simulink library "outp"  (R2021b)
(part 10 of 11)

  UnitConverter274/1 -> VOUTP_AmbDimENFlash_enum/1  "VOUTP_AmbDimENFlash_enum"
  VBCM_AmbLinkDriStaFlash_enum/1 -> VBCM_AmbLinkDriStaFlash_enum_Inproc/1  "VBCM_AmbLinkDriStaFlash_enum"
  VBCM_AmbLinkDriStaFlash_enum_Inproc/1 -> UnitConverter275/1
  UnitConverter275/1 -> VOUTP_AmbLinkDriStaFlash_enum/1  "VOUTP_AmbLinkDriStaFlash_enum"
  VBCM_AmbPwrWarnENFlash_enum/1 -> VBCM_AmbPwrWarnENFlash_enum_Inproc/1  "VBCM_AmbPwrWarnENFlash_enum"
  VBCM_AmbPwrWarnENFlash_enum_Inproc/1 -> UnitConverter276/1
  UnitConverter276/1 -> VOUTP_AmbPwrWarnENFlash_enum/1  "VOUTP_AmbPwrWarnENFlash_enum"
  VBCM_AmbODAENFlash_enum/1 -> VBCM_AmbODAENFlash_enum_Inproc/1  "VBCM_AmbODAENFlash_enum"
  VBCM_AmbODAENFlash_enum_Inproc/1 -> UnitConverter277/1
  UnitConverter277/1 -> VOUTP_AmbODAENFlash_enum/1  "VOUTP_AmbODAENFlash_enum"
  VBCM_AmbColorSta1_enum/1 -> VBCM_AmbColorSta1_enum_Inproc/1  "VBCM_AmbColorSta1_enum"
  VBCM_AmbColorSta1_enum_Inproc/1 -> UnitConverter278/1
  UnitConverter278/1 -> VOUTP_AmbColorSta1_enum/1  "VOUTP_AmbColorSta1_enum"
  VBCM_AmbColorSta2_enum/1 -> VBCM_AmbColorSta2_enum_Inproc/1  "VBCM_AmbColorSta2_enum"
  VBCM_AmbColorSta2_enum_Inproc/1 -> UnitConverter279/1
  UnitConverter279/1 -> VOUTP_AmbColorSta2_enum/1  "VOUTP_AmbColorSta2_enum"
  VBCM_AmbColorSta3_enum/1 -> VBCM_AmbColorSta3_enum_Inproc/1  "VBCM_AmbColorSta3_enum"
  VBCM_AmbColorSta3_enum_Inproc/1 -> UnitConverter280/1
  UnitConverter280/1 -> VOUTP_AmbColorSta3_enum/1  "VOUTP_AmbColorSta3_enum"
  VBCM_AmbColorSta4_enum/1 -> VBCM_AmbColorSta4_enum_Inproc/1  "VBCM_AmbColorSta4_enum"
  VBCM_AmbColorSta4_enum_Inproc/1 -> UnitConverter281/1
  UnitConverter281/1 -> VOUTP_AmbColorSta4_enum/1  "VOUTP_AmbColorSta4_enum"
  VBCM_AmbColorSta5_enum/1 -> VBCM_AmbColorSta5_enum_Inproc/1  "VBCM_AmbColorSta5_enum"
  VBCM_AmbColorSta5_enum_Inproc/1 -> UnitConverter282/1
  UnitConverter282/1 -> VOUTP_AmbColorSta5_enum/1  "VOUTP_AmbColorSta5_enum"
  VBCM_AmbColorSta7_enum/1 -> VBCM_AmbColorSta7_enum_Inproc/1  "VBCM_AmbColorSta7_enum"
  VBCM_AmbColorSta7_enum_Inproc/1 -> UnitConverter283/1
  UnitConverter283/1 -> VOUTP_AmbColorSta7_enum/1  "VOUTP_AmbColorSta7_enum"
  VBCM_AmbBrightnessSta1_enum/1 -> VBCM_AmbBrightnessSta1_enum_Inproc/1  "VBCM_AmbBrightnessSta1_enum"
  VBCM_AmbBrightnessSta1_enum_Inproc/1 -> UnitConverter284/1
  UnitConverter284/1 -> VOUTP_AmbBrightnessSta1_enum/1  "VOUTP_AmbBrightnessSta1_enum"
  VBCM_AmbBrightnessSta2_enum/1 -> VBCM_AmbBrightnessSta2_enum_Inproc/1  "VBCM_AmbBrightnessSta2_enum"
  VBCM_AmbBrightnessSta2_enum_Inproc/1 -> UnitConverter285/1
  UnitConverter285/1 -> VOUTP_AmbBrightnessSta2_enum/1  "VOUTP_AmbBrightnessSta2_enum"
  VBCM_AmbBrightnessSta3_enum/1 -> VBCM_AmbBrightnessSta3_enum_Inproc/1  "VBCM_AmbBrightnessSta3_enum"
  VBCM_AmbBrightnessSta3_enum_Inproc/1 -> UnitConverter286/1
  UnitConverter286/1 -> VOUTP_AmbBrightnessSta3_enum/1  "VOUTP_AmbBrightnessSta3_enum"
  VBCM_AmbBrightnessSta4_enum/1 -> VBCM_AmbBrightnessSta4_enum_Inproc/1  "VBCM_AmbBrightnessSta4_enum"
  VBCM_AmbBrightnessSta4_enum_Inproc/1 -> UnitConverter287/1
  UnitConverter287/1 -> VOUTP_AmbBrightnessSta4_enum/1  "VOUTP_AmbBrightnessSta4_enum"
  VBCM_AmbBrightnessSta5_enum/1 -> VBCM_AmbBrightnessSta5_enum_Inproc/1  "VBCM_AmbBrightnessSta5_enum"
  VBCM_AmbBrightnessSta5_enum_Inproc/1 -> UnitConverter288/1
  UnitConverter288/1 -> VOUTP_AmbBrightnessSta5_enum/1  "VOUTP_AmbBrightnessSta5_enum"
  VBCM_AmbBrightnessSta7_enum/1 -> VBCM_AmbBrightnessSta7_enum_Inproc/1  "VBCM_AmbBrightnessSta7_enum"
  VBCM_AmbBrightnessSta7_enum_Inproc/1 -> UnitConverter289/1
  UnitConverter289/1 -> VOUTP_AmbBrightnessSta7_enum/1  "VOUTP_AmbBrightnessSta7_enum"
  VBCM_HazardIND_flg/1 -> VBCM_HazardIND_flg_Inproc/1  "VBCM_HazardIND_flg"
  VBCM_HazardIND_flg_Inproc/1 -> UnitConverter290/1
  UnitConverter290/1 -> VOUTP_HazardIND_flg/1  "VOUTP_HazardIND_flg"
  VBCM_DimSwSta_flg/1 -> VBCM_DimSwSta_flg_Inproc/1  "VBCM_DimSwSta_flg"
  VBCM_DimSwSta_flg_Inproc/1 -> UnitConverter291/1
  UnitConverter291/1 -> VOUTP_DimSwSta_flg/1  "VOUTP_DimSwSta_flg"
  VBCM_PassSWSta_flg/1 -> VBCM_PassSWSta_flg_Inproc/1  "VBCM_PassSWSta_flg"
  VBCM_PassSWSta_flg_Inproc/1 -> UnitConverter292/1
  UnitConverter292/1 -> VOUTP_PassSWSta_flg/1  "VOUTP_PassSWSta_flg"
  VBCM_FWipSwSta_enum/1 -> VBCM_FWipSwSta_enum_Inproc/1  "VBCM_FWipSwSta_enum"
  VBCM_FWipSwSta_enum_Inproc/1 -> UnitConverter293/1
  UnitConverter293/1 -> VOUTP_FWipSwSta_enum/1  "VOUTP_FWipSwSta_enum"
  VBCM_FWasSwSta_enum/1 -> VBCM_FWasSwSta_enum_Inproc/1  "VBCM_FWasSwSta_enum"
  VBCM_FWasSwSta_enum_Inproc/1 -> UnitConverter294/1
  UnitConverter294/1 -> VOUTP_FWasSwSta_enum/1  "VOUTP_FWasSwSta_enum"
  VBCM_TurnSwSta_enum/1 -> VBCM_TurnSwSta_enum_Inproc/1  "VBCM_TurnSwSta_enum"
  VBCM_TurnSwSta_enum_Inproc/1 -> UnitConverter295/1
  UnitConverter295/1 -> VOUTP_TurnSwSta_enum/1  "VOUTP_TurnSwSta_enum"
  VBCM_TurnSwTSetSta_enum/1 -> VBCM_TurnSwTSetSta_enum_Inproc/1  "VBCM_TurnSwTSetSta_enum"
  VBCM_TurnSwTSetSta_enum_Inproc/1 -> UnitConverter296/1
  UnitConverter296/1 -> VOUTP_TurnSwTSetSta_enum/1  "VOUTP_TurnSwTSetSta_enum"
  VBCM_SPTGENFun_flg/1 -> VBCM_SPTGENFun_flg_Inproc/1  "VBCM_SPTGENFun_flg"
  VBCM_SPTGENFun_flg_Inproc/1 -> UnitConverter297/1
  UnitConverter297/1 -> VOUTP_SPTGENFun_flg/1  "VOUTP_SPTGENFun_flg"
  VBCM_SPTGENFunMem_enum/1 -> VBCM_SPTGENFunMem_enum_Inproc/1  "VBCM_SPTGENFunMem_enum"
  VBCM_SPTGENFunMem_enum_Inproc/1 -> UnitConverter298/1
  UnitConverter298/1 -> VOUTP_SPTGENFunMem_enum/1  "VOUTP_SPTGENFunMem_enum"
  VBCM_OutMode_enum/1 -> VBCM_OutMode_enum_Inproc/1  "VBCM_OutMode_enum"
  VBCM_OutMode_enum_Inproc/1 -> UnitConverter299/1
  UnitConverter299/1 -> VOUTP_OutMode_enum/1  "VOUTP_OutMode_enum"
  VBCM_TurnSwTimeSetSta123_enum/1 -> VBCM_TurnSwTimeSetSta123_enum_Inproc/1  "VBCM_TurnSwTimeSetSta123_enum"
  VBCM_TurnSwTimeSetSta123_enum_Inproc/1 -> UnitConverter300/1
  UnitConverter300/1 -> VOUTP_TurnSwTimeSetSta123_enum/1  "VOUTP_TurnSwTimeSetSta123_enum"
  VBCM_TurnSwTimeSetSta457_enum/1 -> VBCM_TurnSwTimeSetSta457_enum_Inproc/1  "VBCM_TurnSwTimeSetSta457_enum"
  VBCM_TurnSwTimeSetSta457_enum_Inproc/1 -> UnitConverter301/1
  UnitConverter301/1 -> VOUTP_TurnSwTimeSetSta457_enum/1  "VOUTP_TurnSwTimeSetSta457_enum"
  VBCM_FDLHandleLampCmd_flg/1 -> VBCM_FDLHandleLampCmd_flg_Inproc/1  "VBCM_FDLHandleLampCmd_flg"
  VBCM_FDLHandleLampCmd_flg_Inproc/1 -> UnitConverter302/1
  UnitConverter302/1 -> VOUTP_FDLHandleLampCmd_flg/1  "VOUTP_FDLHandleLampCmd_flg"
  VBCM_FDRHandleLampCmd_flg/1 -> VBCM_FDRHandleLampCmd_flg_Inproc/1  "VBCM_FDRHandleLampCmd_flg"
  VBCM_FDRHandleLampCmd_flg_Inproc/1 -> UnitConverter303/1
  UnitConverter303/1 -> VOUTP_FDRHandleLampCmd_flg/1  "VOUTP_FDRHandleLampCmd_flg"
  VBCM_FDHandleCmd_enum/1 -> VBCM_FDHandleCmd_enum_Inproc/1  "VBCM_FDHandleCmd_enum"
  VBCM_FDHandleCmd_enum_Inproc/1 -> UnitConverter304/1
  UnitConverter304/1 -> VOUTP_FDHandleCmd_enum/1  "VOUTP_FDHandleCmd_enum"
  VBCM_HBeamADB_flg/1 -> VBCM_HBeamADB_flg_Inproc/1  "VBCM_HBeamADB_flg"
  VBCM_HBeamADB_flg_Inproc/1 -> UnitConverter305/1
  UnitConverter305/1 -> VOUTP_HBeamADB_flg/1  "VOUTP_HBeamADB_flg"
  VBCM_WalkInUnLkENMem_enum/1 -> VBCM_WalkInUnLkENMem_enum_Inproc/1  "VBCM_WalkInUnLkENMem_enum"
  VBCM_WalkInUnLkENMem_enum_Inproc/1 -> UnitConverter306/1
  UnitConverter306/1 -> VOUTP_WalkInUnLkENMem_enum/1  "VOUTP_WalkInUnLkENMem_enum"
  VBCM_WalkOutLkENMem_enum/1 -> VBCM_WalkOutLkENMem_enum_Inproc/1  "VBCM_WalkOutLkENMem_enum"
  VBCM_WalkOutLkENMem_enum_Inproc/1 -> UnitConverter307/1
  UnitConverter307/1 -> VOUTP_WalkOutLkENMem_enum/1  "VOUTP_WalkOutLkENMem_enum"
  VBCM_RmLpModeENMem_enum/1 -> VBCM_RmLpModeENMem_enum_Inproc/1  "VBCM_RmLpModeENMem_enum"
  VBCM_RmLpModeENMem_enum_Inproc/1 -> UnitConverter308/1
  UnitConverter308/1 -> VOUTP_RmLpModeENMem_enum/1  "VOUTP_RmLpModeENMem_enum"
  VBCM_LockSettingStaMem_enum/1 -> VBCM_LockSettingStaMem_enum_Inproc/1  "VBCM_LockSettingStaMem_enum"
  VBCM_LockSettingStaMem_enum_Inproc/1 -> UnitConverter309/1
  UnitConverter309/1 -> VOUTP_LockSettingStaMem_enum/1  "VOUTP_LockSettingStaMem_enum"
  VBCM_FollowMeENMem_enum/1 -> VBCM_FollowMeENMem_enum_Inproc/1  "VBCM_FollowMeENMem_enum"
  VBCM_FollowMeENMem_enum_Inproc/1 -> UnitConverter310/1
  UnitConverter310/1 -> VOUTP_FollowMeENMem_enum/1  "VOUTP_FollowMeENMem_enum"
  VBCM_WalkInUnLkENFunSta_flg/1 -> VBCM_WalkInUnLkENFunSta_flg_Inproc/1  "VBCM_WalkInUnLkENFunSta_flg"
  VBCM_WalkInUnLkENFunSta_flg_Inproc/1 -> UnitConverter311/1
  UnitConverter311/1 -> VOUTP_WalkInUnLkENFunSta_flg/1  "VOUTP_WalkInUnLkENFunSta_flg"
  VBCM_WalkOutLkENFunSta_flg/1 -> VBCM_WalkOutLkENFunSta_flg_Inproc/1  "VBCM_WalkOutLkENFunSta_flg"
  VBCM_WalkOutLkENFunSta_flg_Inproc/1 -> UnitConverter312/1
  UnitConverter312/1 -> VOUTP_WalkOutLkENFunSta_flg/1  "VOUTP_WalkOutLkENFunSta_flg"
  VBCM_RmLpModeENFunSta_flg/1 -> VBCM_RmLpModeENFunSta_flg_Inproc/1  "VBCM_RmLpModeENFunSta_flg"
  VBCM_RmLpModeENFunSta_flg_Inproc/1 -> UnitConverter313/1
  UnitConverter313/1 -> VOUTP_RmLpModeENFunSta_flg/1  "VOUTP_RmLpModeENFunSta_flg"
  VBCM_FollowMeENFunSta_flg/1 -> VBCM_FollowMeENFunSta_flg_Inproc/1  "VBCM_FollowMeENFunSta_flg"
  VBCM_FollowMeENFunSta_flg_Inproc/1 -> UnitConverter314/1
  UnitConverter314/1 -> VOUTP_FollowMeENFunSta_flg/1  "VOUTP_FollowMeENFunSta_flg"
  VBCM_HoodRelCmd_flg/1 -> VBCM_HoodRelCmd_flg_Inproc/1  "VBCM_HoodRelCmd_flg"
  VBCM_HoodRelCmd_flg_Inproc/1 -> UnitConverter315/1
  UnitConverter315/1 -> VOUTP_HoodRelCmd_flg/1  "VOUTP_HoodRelCmd_flg"
  VBCM_WelcomeLight_enum/1 -> VBCM_WelcomeLight_enum_Inproc/1  "VBCM_WelcomeLight_enum"
  VBCM_WelcomeLight_enum_Inproc/1 -> UnitConverter316/1
  UnitConverter316/1 -> VOUTP_WelcomeLight_enum/1  "VOUTP_WelcomeLight_enum"
  VBCM_PTGOpenHeightSta_enum/1 -> VBCM_PTGOpenHeightSta_enum_Inproc/1  "VBCM_PTGOpenHeightSta_enum"
  VBCM_PTGOpenHeightSta_enum_Inproc/1 -> UnitConverter317/1
  UnitConverter317/1 -> VOUTP_PTGOpenHeightSta_enum/1  "VOUTP_PTGOpenHeightSta_enum"
  VBCM_UserHeightSet_cnt/1 -> VBCM_UserHeightSet_cnt_Inproc/1  "VBCM_UserHeightSet_cnt"
  VBCM_UserHeightSet_cnt_Inproc/1 -> UnitConverter318/1
  UnitConverter318/1 -> VOUTP_UserHeightSet_cnt/1  "VOUTP_UserHeightSet_cnt"
  VBCM_PTGUserHeight1_cnt/1 -> VBCM_PTGUserHeight1_cnt_Inproc/1  "VBCM_PTGUserHeight1_cnt"
  VBCM_PTGUserHeight1_cnt_Inproc/1 -> UnitConverter319/1
  UnitConverter319/1 -> VOUTP_PTGUserHeight1_cnt/1  "VOUTP_PTGUserHeight1_cnt"
  VBCM_PTGUserHeight2_cnt/1 -> VBCM_PTGUserHeight2_cnt_Inproc/1  "VBCM_PTGUserHeight2_cnt"
  VBCM_PTGUserHeight2_cnt_Inproc/1 -> UnitConverter320/1
  UnitConverter320/1 -> VOUTP_PTGUserHeight2_cnt/1  "VOUTP_PTGUserHeight2_cnt"
  VBCM_PTGUserHeight3_cnt/1 -> VBCM_PTGUserHeight3_cnt_Inproc/1  "VBCM_PTGUserHeight3_cnt"
  VBCM_PTGUserHeight3_cnt_Inproc/1 -> UnitConverter321/1
  UnitConverter321/1 -> VOUTP_PTGUserHeight3_cnt/1  "VOUTP_PTGUserHeight3_cnt"
  VBCM_PTGUserHeight4_cnt/1 -> VBCM_PTGUserHeight4_cnt_Inproc/1  "VBCM_PTGUserHeight4_cnt"
  VBCM_PTGUserHeight4_cnt_Inproc/1 -> UnitConverter322/1
  UnitConverter322/1 -> VOUTP_PTGUserHeight4_cnt/1  "VOUTP_PTGUserHeight4_cnt"
  VBCM_PTGUserHeight5_cnt/1 -> VBCM_PTGUserHeight5_cnt_Inproc/1  "VBCM_PTGUserHeight5_cnt"
  VBCM_PTGUserHeight5_cnt_Inproc/1 -> UnitConverter323/1
  UnitConverter323/1 -> VOUTP_PTGUserHeight5_cnt/1  "VOUTP_PTGUserHeight5_cnt"
  VBCM_PTGUserHeight7_cnt/1 -> VBCM_PTGUserHeight7_cnt_Inproc/1  "VBCM_PTGUserHeight7_cnt"
  VBCM_PTGUserHeight7_cnt_Inproc/1 -> UnitConverter324/1
  UnitConverter324/1 -> VOUTP_PTGUserHeight7_cnt/1  "VOUTP_PTGUserHeight7_cnt"
  VBCM_PTGOpenHeight12_enum/1 -> VBCM_PTGOpenHeight12_enum_Inproc/1  "VBCM_PTGOpenHeight12_enum"
  VBCM_PTGOpenHeight12_enum_Inproc/1 -> UnitConverter325/1
  UnitConverter325/1 -> VOUTP_PTGOpenHeight12_enum/1  "VOUTP_PTGOpenHeight12_enum"
  VBCM_PTGOpenHeight34_enum/1 -> VBCM_PTGOpenHeight34_enum_Inproc/1  "VBCM_PTGOpenHeight34_enum"
  VBCM_PTGOpenHeight34_enum_Inproc/1 -> UnitConverter326/1
  UnitConverter326/1 -> VOUTP_PTGOpenHeight34_enum/1  "VOUTP_PTGOpenHeight34_enum"
  VBCM_PTGOpenHeight57_enum/1 -> VBCM_PTGOpenHeight57_enum_Inproc/1  "VBCM_PTGOpenHeight57_enum"
  VBCM_PTGOpenHeight57_enum_Inproc/1 -> UnitConverter327/1
  UnitConverter327/1 -> VOUTP_PTGOpenHeight57_enum/1  "VOUTP_PTGOpenHeight57_enum"
  VBCM_SenstivityPosnCmd_enum/1 -> VBCM_SenstivityPosnCmd_enum_Inproc/1  "VBCM_SenstivityPosnCmd_enum"
  VBCM_SenstivityPosnCmd_enum_Inproc/1 -> UnitConverter328/1
  UnitConverter328/1 -> VOUTP_SenstivityPosnCmd_enum/1  "VOUTP_SenstivityPosnCmd_enum"
  VBCM_TimeGapLevelSta_enum/1 -> VBCM_TimeGapLevelSta_enum_Inproc/1  "VBCM_TimeGapLevelSta_enum"
  VBCM_TimeGapLevelSta_enum_Inproc/1 -> UnitConverter329/1
  UnitConverter329/1 -> VOUTP_TimeGapLevelSta_enum/1  "VOUTP_TimeGapLevelSta_enum"
  VBCM_ACCLevelMem12_enum/1 -> VBCM_ACCLevelMem12_enum_Inproc/1  "VBCM_ACCLevelMem12_enum"
  VBCM_ACCLevelMem12_enum_Inproc/1 -> UnitConverter330/1
  UnitConverter330/1 -> VOUTP_ACCLevelMem12_enum/1  "VOUTP_ACCLevelMem12_enum"
  VBCM_ACCLevelMem34_enum/1 -> VBCM_ACCLevelMem34_enum_Inproc/1  "VBCM_ACCLevelMem34_enum"
  VBCM_ACCLevelMem34_enum_Inproc/1 -> UnitConverter331/1
  UnitConverter331/1 -> VOUTP_ACCLevelMem34_enum/1  "VOUTP_ACCLevelMem34_enum"
  VBCM_ACCLevelMem57_enum/1 -> VBCM_ACCLevelMem57_enum_Inproc/1  "VBCM_ACCLevelMem57_enum"
  VBCM_ACCLevelMem57_enum_Inproc/1 -> UnitConverter332/1
  UnitConverter332/1 -> VOUTP_ACCLevelMem57_enum/1  "VOUTP_ACCLevelMem57_enum"
  VBCM_LRightStaCmd_flg/1 -> VBCM_LRightStaCmd_flg_Inproc/1  "VBCM_LRightStaCmd_flg"
  VBCM_LRightStaCmd_flg_Inproc/1 -> UnitConverter333/1
  UnitConverter333/1 -> VOUTP_LRightStaCmd_flg/1  "VOUTP_LRightStaCmd_flg"
  VBCM_LLeftStaCmd_flg/1 -> VBCM_LLeftStaCmd_flg_Inproc/1  "VBCM_LLeftStaCmd_flg"
  VBCM_LLeftStaCmd_flg_Inproc/1 -> UnitConverter334/1
  UnitConverter334/1 -> VOUTP_LLeftStaCmd_flg/1  "VOUTP_LLeftStaCmd_flg"
  VBCM_AutoLockSta_flg/1 -> VBCM_AutoLockSta_flg_Inproc/1  "VBCM_AutoLockSta_flg"
  VBCM_AutoLockSta_flg_Inproc/1 -> UnitConverter335/1
  UnitConverter335/1 -> VOUTP_AutoLockSta_flg/1  "VOUTP_AutoLockSta_flg"
  VBCM_AutoLockMem_enum/1 -> VBCM_AutoLockMem_enum_Inproc/1  "VBCM_AutoLockMem_enum"
  VBCM_AutoLockMem_enum_Inproc/1 -> UnitConverter336/1
  UnitConverter336/1 -> VOUTP_AutoLockMem_enum/1  "VOUTP_AutoLockMem_enum"
  VBCM_AutoUnlockSta_flg/1 -> VBCM_AutoUnlockSta_flg_Inproc/1  "VBCM_AutoUnlockSta_flg"
  VBCM_AutoUnlockSta_flg_Inproc/1 -> UnitConverter337/1
  UnitConverter337/1 -> VOUTP_AutoUnlockSta_flg/1  "VOUTP_AutoUnlockSta_flg"
  VBCM_AutoUnlockMem_enum/1 -> VBCM_AutoUnlockMem_enum_Inproc/1  "VBCM_AutoUnlockMem_enum"
  VBCM_AutoUnlockMem_enum_Inproc/1 -> UnitConverter338/1
  UnitConverter338/1 -> VOUTP_AutoUnlockMem_enum/1  "VOUTP_AutoUnlockMem_enum"
  VBCM_HMIKey1FuncSta_enum/1 -> VBCM_HMIKey1FuncSta_enum_Inproc/1  "VBCM_HMIKey1FuncSta_enum"
  VBCM_HMIKey1FuncSta_enum_Inproc/1 -> UnitConverter339/1
  UnitConverter339/1 -> VOUTP_HMIKey1FuncSta_enum/1  "VOUTP_HMIKey1FuncSta_enum"
  VBCM_HMIKey2FuncSta_enum/1 -> VBCM_HMIKey2FuncSta_enum_Inproc/1  "VBCM_HMIKey2FuncSta_enum"
  VBCM_HMIKey2FuncSta_enum_Inproc/1 -> UnitConverter340/1
  UnitConverter340/1 -> VOUTP_HMIKey2FuncSta_enum/1  "VOUTP_HMIKey2FuncSta_enum"
  VBCM_HMIKey3FuncSta_enum/1 -> VBCM_HMIKey3FuncSta_enum_Inproc/1  "VBCM_HMIKey3FuncSta_enum"
  VBCM_HMIKey3FuncSta_enum_Inproc/1 -> UnitConverter341/1
  UnitConverter341/1 -> VOUTP_HMIKey3FuncSta_enum/1  "VOUTP_HMIKey3FuncSta_enum"
  VBCM_HMIKey4FuncSta_enum/1 -> VBCM_HMIKey4FuncSta_enum_Inproc/1  "VBCM_HMIKey4FuncSta_enum"
  VBCM_HMIKey4FuncSta_enum_Inproc/1 -> UnitConverter342/1
  UnitConverter342/1 -> VOUTP_HMIKey4FuncSta_enum/1  "VOUTP_HMIKey4FuncSta_enum"
  VBCM_HMIKey5FuncSta_enum/1 -> VBCM_HMIKey5FuncSta_enum_Inproc/1  "VBCM_HMIKey5FuncSta_enum"
  VBCM_HMIKey5FuncSta_enum_Inproc/1 -> UnitConverter343/1
  UnitConverter343/1 -> VOUTP_HMIKey5FuncSta_enum/1  "VOUTP_HMIKey5FuncSta_enum"
  VBCM_HMIKey6FuncSta_enum/1 -> VBCM_HMIKey6FuncSta_enum_Inproc/1  "VBCM_HMIKey6FuncSta_enum"
  VBCM_HMIKey6FuncSta_enum_Inproc/1 -> UnitConverter344/1
  UnitConverter344/1 -> VOUTP_HMIKey6FuncSta_enum/1  "VOUTP_HMIKey6FuncSta_enum"
  VBCM_HMIKey7FuncSta_enum/1 -> VBCM_HMIKey7FuncSta_enum_Inproc/1  "VBCM_HMIKey7FuncSta_enum"
  VBCM_HMIKey7FuncSta_enum_Inproc/1 -> UnitConverter345/1
  UnitConverter345/1 -> VOUTP_HMIKey7FuncSta_enum/1  "VOUTP_HMIKey7FuncSta_enum"
  VBCM_HMIKey8FuncSta_enum/1 -> VBCM_HMIKey8FuncSta_enum_Inproc/1  "VBCM_HMIKey8FuncSta_enum"
  VBCM_HMIKey8FuncSta_enum_Inproc/1 -> UnitConverter346/1
  UnitConverter346/1 -> VOUTP_HMIKey8FuncSta_enum/1  "VOUTP_HMIKey8FuncSta_enum"
  VBCM_AutoWipHSpdENSta_flg/1 -> VBCM_AutoWipHSpdENSta_flg_Inproc/1  "VBCM_AutoWipHSpdENSta_flg"
  VBCM_AutoWipHSpdENSta_flg_Inproc/1 -> UnitConverter347/1
  UnitConverter347/1 -> VOUTP_AutoWipHSpdENSta_flg/1  "VOUTP_AutoWipHSpdENSta_flg"
  VBCM_DrvWdwReqAP_enum/1 -> VBCM_DrvWdwReqAP_enum_Inproc/1  "VBCM_DrvWdwReqAP_enum"
  VBCM_DrvWdwReqAP_enum_Inproc/1 -> UnitConverter348/1
  UnitConverter348/1 -> VOUTP_DrvWdwReqAP_enum/1  "VOUTP_DrvWdwReqAP_enum"
  VBCM_PasWdwReqAP_enum/1 -> VBCM_PasWdwReqAP_enum_Inproc/1  "VBCM_PasWdwReqAP_enum"
  VBCM_PasWdwReqAP_enum_Inproc/1 -> UnitConverter349/1
  UnitConverter349/1 -> VOUTP_PasWdwReqAP_enum/1  "VOUTP_PasWdwReqAP_enum"
  VBCM_DrRWdwReqAP_enum/1 -> VBCM_DrRWdwReqAP_enum_Inproc/1  "VBCM_DrRWdwReqAP_enum"
  VBCM_DrRWdwReqAP_enum_Inproc/1 -> UnitConverter350/1
  UnitConverter350/1 -> VOUTP_DrRWdwReqAP_enum/1  "VOUTP_DrRWdwReqAP_enum"
  VBCM_PsRWdwReqAP_enum/1 -> VBCM_PsRWdwReqAP_enum_Inproc/1  "VBCM_PsRWdwReqAP_enum"
  VBCM_PsRWdwReqAP_enum_Inproc/1 -> UnitConverter351/1
  UnitConverter351/1 -> VOUTP_PsRWdwReqAP_enum/1  "VOUTP_PsRWdwReqAP_enum"
  VBCM_CLWinLockDrSta_flg/1 -> VBCM_CLWinLockDrSta_flg_Inproc/1  "VBCM_CLWinLockDrSta_flg"
  VBCM_CLWinLockDrSta_flg_Inproc/1 -> UnitConverter352/1
  UnitConverter352/1 -> VOUTP_CLWinLockDrSta_flg/1  "VOUTP_CLWinLockDrSta_flg"
  VBCM_CLWinLockDrStaMem_enum/1 -> VBCM_CLWinLockDrStaMem_enum_Inproc/1  "VBCM_CLWinLockDrStaMem_enum"
  VBCM_CLWinLockDrStaMem_enum_Inproc/1 -> UnitConverter353/1
  UnitConverter353/1 -> VOUTP_CLWinLockDrStaMem_enum/1  "VOUTP_CLWinLockDrStaMem_enum"
  VBCM_WinLFOpenedSta_pct/1 -> VBCM_WinLFOpenedSta_pct_Inproc/1  "VBCM_WinLFOpenedSta_pct"
  VBCM_WinLFOpenedSta_pct_Inproc/1 -> UnitConverter354/1
  UnitConverter354/1 -> VOUTP_WinLFOpenedSta_pct/1  "VOUTP_WinLFOpenedSta_pct"
  VBCM_WinRFOpenedSta_pct/1 -> VBCM_WinRFOpenedSta_pct_Inproc/1  "VBCM_WinRFOpenedSta_pct"
  VBCM_WinRFOpenedSta_pct_Inproc/1 -> UnitConverter355/1
  UnitConverter355/1 -> VOUTP_WinRFOpenedSta_pct/1  "VOUTP_WinRFOpenedSta_pct"
  VBCM_WinLROpenedSta_pct/1 -> VBCM_WinLROpenedSta_pct_Inproc/1  "VBCM_WinLROpenedSta_pct"
  VBCM_WinLROpenedSta_pct_Inproc/1 -> UnitConverter356/1
  UnitConverter356/1 -> VOUTP_WinLROpenedSta_pct/1  "VOUTP_WinLROpenedSta_pct"
  VBCM_WinRROpenedSta_pct/1 -> VBCM_WinRROpenedSta_pct_Inproc/1  "VBCM_WinRROpenedSta_pct"
  VBCM_WinRROpenedSta_pct_Inproc/1 -> UnitConverter357/1
  UnitConverter357/1 -> VOUTP_WinRROpenedSta_pct/1  "VOUTP_WinRROpenedSta_pct"
  VDDM_C3BMS6RCDTC_raw32/1 -> VDDM_C3BMS6RCDTC_raw32_Inproc/1  "VDDM_C3BMS6RCDTC_raw32"
  VDDM_C3BMS6RCDTC_raw32_Inproc/1 -> UnitConverter358/1
  UnitConverter358/1 -> VOUTP_C3BMS6RCDTC_raw32/1  "VOUTP_C3BMS6RCDTC_raw32"
  VDDM_C3BMS6CSDTC_raw32/1 -> VDDM_C3BMS6CSDTC_raw32_Inproc/1  "VDDM_C3BMS6CSDTC_raw32"
  VDDM_C3BMS6CSDTC_raw32_Inproc/1 -> UnitConverter359/1
  UnitConverter359/1 -> VOUTP_C3BMS6CSDTC_raw32/1  "VOUTP_C3BMS6CSDTC_raw32"
  VDDM_C3BMS6LCDTC_raw32/1 -> VDDM_C3BMS6LCDTC_raw32_Inproc/1  "VDDM_C3BMS6LCDTC_raw32"
  VDDM_C3BMS6LCDTC_raw32_Inproc/1 -> UnitConverter360/1
  UnitConverter360/1 -> VOUTP_C3BMS6LCDTC_raw32/1  "VOUTP_C3BMS6LCDTC_raw32"
  VDDM_C3BMS1RCDTC_raw32/1 -> VDDM_C3BMS1RCDTC_raw32_Inproc/1  "VDDM_C3BMS1RCDTC_raw32"
  VDDM_C3BMS1RCDTC_raw32_Inproc/1 -> UnitConverter361/1
  UnitConverter361/1 -> VOUTP_C3BMS1RCDTC_raw32/1  "VOUTP_C3BMS1RCDTC_raw32"
  VDDM_C3BMS1CSDTC_raw32/1 -> VDDM_C3BMS1CSDTC_raw32_Inproc/1  "VDDM_C3BMS1CSDTC_raw32"
  VDDM_C3BMS1CSDTC_raw32_Inproc/1 -> UnitConverter362/1
  UnitConverter362/1 -> VOUTP_C3BMS1CSDTC_raw32/1  "VOUTP_C3BMS1CSDTC_raw32"
  VDDM_C3BMS1LCDTC_raw32/1 -> VDDM_C3BMS1LCDTC_raw32_Inproc/1  "VDDM_C3BMS1LCDTC_raw32"
  VDDM_C3BMS1LCDTC_raw32_Inproc/1 -> UnitConverter363/1
  UnitConverter363/1 -> VOUTP_C3BMS1LCDTC_raw32/1  "VOUTP_C3BMS1LCDTC_raw32"
  VDDM_C3CCU1RCDTC_raw32/1 -> VDDM_C3CCU1RCDTC_raw32_Inproc/1  "VDDM_C3CCU1RCDTC_raw32"
  VDDM_C3CCU1RCDTC_raw32_Inproc/1 -> UnitConverter364/1
  UnitConverter364/1 -> VOUTP_C3CCU1RCDTC_raw32/1  "VOUTP_C3CCU1RCDTC_raw32"
  VDDM_C3CCU1CSDTC_raw32/1 -> VDDM_C3CCU1CSDTC_raw32_Inproc/1  "VDDM_C3CCU1CSDTC_raw32"
  VDDM_C3CCU1CSDTC_raw32_Inproc/1 -> UnitConverter365/1
  UnitConverter365/1 -> VOUTP_C3CCU1CSDTC_raw32/1  "VOUTP_C3CCU1CSDTC_raw32"
  VDDM_C3CCU1LCDTC_raw32/1 -> VDDM_C3CCU1LCDTC_raw32_Inproc/1  "VDDM_C3CCU1LCDTC_raw32"
  VDDM_C3CCU1LCDTC_raw32_Inproc/1 -> UnitConverter366/1
  UnitConverter366/1 -> VOUTP_C3CCU1LCDTC_raw32/1  "VOUTP_C3CCU1LCDTC_raw32"
  VDDM_C3CCU2RCDTC_raw32/1 -> VDDM_C3CCU2RCDTC_raw32_Inproc/1  "VDDM_C3CCU2RCDTC_raw32"
  VDDM_C3CCU2RCDTC_raw32_Inproc/1 -> UnitConverter367/1
  UnitConverter367/1 -> VOUTP_C3CCU2RCDTC_raw32/1  "VOUTP_C3CCU2RCDTC_raw32"
  VDDM_C3CCU2CSDTC_raw32/1 -> VDDM_C3CCU2CSDTC_raw32_Inproc/1  "VDDM_C3CCU2CSDTC_raw32"
  VDDM_C3CCU2CSDTC_raw32_Inproc/1 -> UnitConverter368/1
  UnitConverter368/1 -> VOUTP_C3CCU2CSDTC_raw32/1  "VOUTP_C3CCU2CSDTC_raw32"
  VDDM_C3CCU2LCDTC_raw32/1 -> VDDM_C3CCU2LCDTC_raw32_Inproc/1  "VDDM_C3CCU2LCDTC_raw32"
  VDDM_C3CCU2LCDTC_raw32_Inproc/1 -> UnitConverter369/1
  UnitConverter369/1 -> VOUTP_C3CCU2LCDTC_raw32/1  "VOUTP_C3CCU2LCDTC_raw32"
  VDDM_C1ABM1RCDTC_raw32/1 -> VDDM_C1ABM1RCDTC_raw32_Inproc/1  "VDDM_C1ABM1RCDTC_raw32"
  VDDM_C1ABM1RCDTC_raw32_Inproc/1 -> UnitConverter370/1
  UnitConverter370/1 -> VOUTP_C1ABM1RCDTC_raw32/1  "VOUTP_C1ABM1RCDTC_raw32"
  VDDM_C1ABM1CSDTC_raw32/1 -> VDDM_C1ABM1CSDTC_raw32_Inproc/1  "VDDM_C1ABM1CSDTC_raw32"
  VDDM_C1ABM1CSDTC_raw32_Inproc/1 -> UnitConverter371/1
  UnitConverter371/1 -> VOUTP_C1ABM1CSDTC_raw32/1  "VOUTP_C1ABM1CSDTC_raw32"
  VDDM_C1ABM1LCDTC_raw32/1 -> VDDM_C1ABM1LCDTC_raw32_Inproc/1  "VDDM_C1ABM1LCDTC_raw32"
  VDDM_C1ABM1LCDTC_raw32_Inproc/1 -> UnitConverter372/1
  UnitConverter372/1 -> VOUTP_C1ABM1LCDTC_raw32/1  "VOUTP_C1ABM1LCDTC_raw32"
  VDDM_Lv1ErrDTC_raw32/1 -> VDDM_Lv1ErrDTC_raw32_Inproc/1  "VDDM_Lv1ErrDTC_raw32"
  VDDM_Lv1ErrDTC_raw32_Inproc/1 -> UnitConverter373/1
  UnitConverter373/1 -> VOUTP_Lv1ErrDTC_raw32/1  "VOUTP_Lv1ErrDTC_raw32"
  VDDM_Lv2ErrDTC_raw32/1 -> VDDM_Lv2ErrDTC_raw32_Inproc/1  "VDDM_Lv2ErrDTC_raw32"
  VDDM_Lv2ErrDTC_raw32_Inproc/1 -> UnitConverter374/1
  UnitConverter374/1 -> VOUTP_Lv2ErrDTC_raw32/1  "VOUTP_Lv2ErrDTC_raw32"
  VDDM_Lv3ErrDTC_raw32/1 -> VDDM_Lv3ErrDTC_raw32_Inproc/1  "VDDM_Lv3ErrDTC_raw32"
  VDDM_Lv3ErrDTC_raw32_Inproc/1 -> UnitConverter375/1
  UnitConverter375/1 -> VOUTP_Lv3ErrDTC_raw32/1  "VOUTP_Lv3ErrDTC_raw32"
  VDDM_Lv4ErrDTC_raw32/1 -> VDDM_Lv4ErrDTC_raw32_Inproc/1  "VDDM_Lv4ErrDTC_raw32"
  VDDM_Lv4ErrDTC_raw32_Inproc/1 -> UnitConverter376/1
  UnitConverter376/1 -> VOUTP_Lv4ErrDTC_raw32/1  "VOUTP_Lv4ErrDTC_raw32"
  VDDM_BrkSWErrDTC_raw32/1 -> VDDM_BrkSWErrDTC_raw32_Inproc/1  "VDDM_BrkSWErrDTC_raw32"
  VDDM_BrkSWErrDTC_raw32_Inproc/1 -> UnitConverter377/1
  UnitConverter377/1 -> VOUTP_BrkSWErrDTC_raw32/1  "VOUTP_BrkSWErrDTC_raw32"
  VDDM_BrkSWNoBacDTC_raw32/1 -> VDDM_BrkSWNoBacDTC_raw32_Inproc/1  "VDDM_BrkSWNoBacDTC_raw32"
  VDDM_BrkSWNoBacDTC_raw32_Inproc/1 -> UnitConverter378/1
  UnitConverter378/1 -> VOUTP_BrkSWNoBacDTC_raw32/1  "VOUTP_BrkSWNoBacDTC_raw32"
  VDDM_KeyAuthDTC_raw32/1 -> VDDM_KeyAuthDTC_raw32_Inproc/1  "VDDM_KeyAuthDTC_raw32"
  VDDM_KeyAuthDTC_raw32_Inproc/1 -> UnitConverter379/1
  UnitConverter379/1 -> VOUTP_KeyAuthDTC_raw32/1  "VOUTP_KeyAuthDTC_raw32"
  VDDM_ONtoRdyDTC_raw32/1 -> VDDM_ONtoRdyDTC_raw32_Inproc/1  "VDDM_ONtoRdyDTC_raw32"
  VDDM_ONtoRdyDTC_raw32_Inproc/1 -> UnitConverter380/1
  UnitConverter380/1 -> VOUTP_ONtoRdyDTC_raw32/1  "VOUTP_ONtoRdyDTC_raw32"
  VDDM_HVB4PreDTC_raw32/1 -> VDDM_HVB4PreDTC_raw32_Inproc/1  "VDDM_HVB4PreDTC_raw32"
  VDDM_HVB4PreDTC_raw32_Inproc/1 -> UnitConverter381/1
  UnitConverter381/1 -> VOUTP_HVB4PreDTC_raw32/1  "VOUTP_HVB4PreDTC_raw32"
  VDDM_MCU4PreDTC_raw32/1 -> VDDM_MCU4PreDTC_raw32_Inproc/1  "VDDM_MCU4PreDTC_raw32"
  VDDM_MCU4PreDTC_raw32_Inproc/1 -> UnitConverter382/1
  UnitConverter382/1 -> VOUTP_MCU4PreDTC_raw32/1  "VOUTP_MCU4PreDTC_raw32"
  VDDM_DCDC4PreDTC_raw32/1 -> VDDM_DCDC4PreDTC_raw32_Inproc/1  "VDDM_DCDC4PreDTC_raw32"
  VDDM_DCDC4PreDTC_raw32_Inproc/1 -> UnitConverter383/1
  UnitConverter383/1 -> VOUTP_DCDC4PreDTC_raw32/1  "VOUTP_DCDC4PreDTC_raw32"
  VDDM_HVRlyCloDTC_raw32/1 -> VDDM_HVRlyCloDTC_raw32_Inproc/1  "VDDM_HVRlyCloDTC_raw32"
  VDDM_HVRlyCloDTC_raw32_Inproc/1 -> UnitConverter384/1
  UnitConverter384/1 -> VOUTP_HVRlyCloDTC_raw32/1  "VOUTP_HVRlyCloDTC_raw32"
  VDDM_BMSRdyDTC_raw32/1 -> VDDM_BMSRdyDTC_raw32_Inproc/1  "VDDM_BMSRdyDTC_raw32"
  VDDM_BMSRdyDTC_raw32_Inproc/1 -> UnitConverter385/1
  UnitConverter385/1 -> VOUTP_BMSRdyDTC_raw32/1  "VOUTP_BMSRdyDTC_raw32"
  VDDM_DCDCEnaDTC_raw32/1 -> VDDM_DCDCEnaDTC_raw32_Inproc/1  "VDDM_DCDCEnaDTC_raw32"
  VDDM_DCDCEnaDTC_raw32_Inproc/1 -> UnitConverter386/1
  UnitConverter386/1 -> VOUTP_DCDCEnaDTC_raw32/1  "VOUTP_DCDCEnaDTC_raw32"
  VDDM_HiLvSaChkDTC_raw32/1 -> VDDM_HiLvSaChkDTC_raw32_Inproc/1  "VDDM_HiLvSaChkDTC_raw32"
  VDDM_HiLvSaChkDTC_raw32_Inproc/1 -> UnitConverter387/1
  UnitConverter387/1 -> VOUTP_HiLvSaChkDTC_raw32/1  "VOUTP_HiLvSaChkDTC_raw32"
  VDDM_MidLvSaChkDTC_raw32/1 -> VDDM_MidLvSaChkDTC_raw32_Inproc/1  "VDDM_MidLvSaChkDTC_raw32"
  VDDM_MidLvSaChkDTC_raw32_Inproc/1 -> UnitConverter388/1
  UnitConverter388/1 -> VOUTP_MidLvSaChkDTC_raw32/1  "VOUTP_MidLvSaChkDTC_raw32"
  VDDM_MCUDisDTC_raw32/1 -> VDDM_MCUDisDTC_raw32_Inproc/1  "VDDM_MCUDisDTC_raw32"
  VDDM_MCUDisDTC_raw32_Inproc/1 -> UnitConverter389/1
  UnitConverter389/1 -> VOUTP_MCUDisDTC_raw32/1  "VOUTP_MCUDisDTC_raw32"
  VDDM_DCDCDisDTC_raw32/1 -> VDDM_DCDCDisDTC_raw32_Inproc/1  "VDDM_DCDCDisDTC_raw32"
  VDDM_DCDCDisDTC_raw32_Inproc/1 -> UnitConverter390/1
  UnitConverter390/1 -> VOUTP_DCDCDisDTC_raw32/1  "VOUTP_DCDCDisDTC_raw32"
  VDDM_HVRlyOpDTC_raw32/1 -> VDDM_HVRlyOpDTC_raw32_Inproc/1  "VDDM_HVRlyOpDTC_raw32"
  VDDM_HVRlyOpDTC_raw32_Inproc/1 -> UnitConverter391/1
  UnitConverter391/1 -> VOUTP_HVRlyOpDTC_raw32/1  "VOUTP_HVRlyOpDTC_raw32"
  VDDM_MCUActDTC_raw32/1 -> VDDM_MCUActDTC_raw32_Inproc/1  "VDDM_MCUActDTC_raw32"
  VDDM_MCUActDTC_raw32_Inproc/1 -> UnitConverter392/1
  UnitConverter392/1 -> VOUTP_MCUActDTC_raw32/1  "VOUTP_MCUActDTC_raw32"
  VDDM_OBC4PreDTC_raw32/1 -> VDDM_OBC4PreDTC_raw32_Inproc/1  "VDDM_OBC4PreDTC_raw32"
  VDDM_OBC4PreDTC_raw32_Inproc/1 -> UnitConverter393/1
  UnitConverter393/1 -> VOUTP_OBC4PreDTC_raw32/1  "VOUTP_OBC4PreDTC_raw32"
  VDDM_IniLVLoDTC_raw32/1 -> VDDM_IniLVLoDTC_raw32_Inproc/1  "VDDM_IniLVLoDTC_raw32"
  VDDM_IniLVLoDTC_raw32_Inproc/1 -> UnitConverter394/1
  UnitConverter394/1 -> VOUTP_IniLVLoDTC_raw32/1  "VOUTP_IniLVLoDTC_raw32"
  VDDM_LVSupLoDTC_raw32/1 -> VDDM_LVSupLoDTC_raw32_Inproc/1  "VDDM_LVSupLoDTC_raw32"
  VDDM_LVSupLoDTC_raw32_Inproc/1 -> UnitConverter395/1
  UnitConverter395/1 -> VOUTP_LVSupLoDTC_raw32/1  "VOUTP_LVSupLoDTC_raw32"
  VDDM_LVSupHiDTC_raw32/1 -> VDDM_LVSupHiDTC_raw32_Inproc/1  "VDDM_LVSupHiDTC_raw32"
  VDDM_LVSupHiDTC_raw32_Inproc/1 -> UnitConverter396/1
  UnitConverter396/1 -> VOUTP_LVSupHiDTC_raw32/1  "VOUTP_LVSupHiDTC_raw32"
  VDDM_DrStSWDTC_raw32/1 -> VDDM_DrStSWDTC_raw32_Inproc/1  "VDDM_DrStSWDTC_raw32"
  VDDM_DrStSWDTC_raw32_Inproc/1 -> UnitConverter397/1
  UnitConverter397/1 -> VOUTP_DrStSWDTC_raw32/1  "VOUTP_DrStSWDTC_raw32"
  VDDM_FLDoorSWDTC_raw32/1 -> VDDM_FLDoorSWDTC_raw32_Inproc/1  "VDDM_FLDoorSWDTC_raw32"
  VDDM_FLDoorSWDTC_raw32_Inproc/1 -> UnitConverter398/1
  UnitConverter398/1 -> VOUTP_FLDoorSWDTC_raw32/1  "VOUTP_FLDoorSWDTC_raw32"
  VDDM_RLDoorSWDTC_raw32/1 -> VDDM_RLDoorSWDTC_raw32_Inproc/1  "VDDM_RLDoorSWDTC_raw32"
  VDDM_RLDoorSWDTC_raw32_Inproc/1 -> UnitConverter399/1
  UnitConverter399/1 -> VOUTP_RLDoorSWDTC_raw32/1  "VOUTP_RLDoorSWDTC_raw32"
  VDDM_FRDoorSWDTC_raw32/1 -> VDDM_FRDoorSWDTC_raw32_Inproc/1  "VDDM_FRDoorSWDTC_raw32"
  VDDM_FRDoorSWDTC_raw32_Inproc/1 -> UnitConverter400/1
  UnitConverter400/1 -> VOUTP_FRDoorSWDTC_raw32/1  "VOUTP_FRDoorSWDTC_raw32"
  VDDM_RRDoorSWDTC_raw32/1 -> VDDM_RRDoorSWDTC_raw32_Inproc/1  "VDDM_RRDoorSWDTC_raw32"
  VDDM_RRDoorSWDTC_raw32_Inproc/1 -> UnitConverter401/1
  UnitConverter401/1 -> VOUTP_RRDoorSWDTC_raw32/1  "VOUTP_RRDoorSWDTC_raw32"
  VDDM_HoodSWDTC_raw32/1 -> VDDM_HoodSWDTC_raw32_Inproc/1  "VDDM_HoodSWDTC_raw32"
  VDDM_HoodSWDTC_raw32_Inproc/1 -> UnitConverter402/1
  UnitConverter402/1 -> VOUTP_HoodSWDTC_raw32/1  "VOUTP_HoodSWDTC_raw32"
  VDDM_TailgaSWDTC_raw32/1 -> VDDM_TailgaSWDTC_raw32_Inproc/1  "VDDM_TailgaSWDTC_raw32"
  VDDM_TailgaSWDTC_raw32_Inproc/1 -> UnitConverter403/1
  UnitConverter403/1 -> VOUTP_TailgaSWDTC_raw32/1  "VOUTP_TailgaSWDTC_raw32"
  VDDM_EDriveSysErrVCUErr_flg/1 -> VDDM_EDriveSysErrVCUErr_flg_Inproc/1  "VDDM_EDriveSysErrVCUErr_flg"
  VDDM_EDriveSysErrVCUErr_flg_Inproc/1 -> UnitConverter404/1
  UnitConverter404/1 -> VOUTP_EDriveSysErrVCUErr_flg/1  "VOUTP_EDriveSysErrVCUErr_flg"
  VDDM_VehMalfunLevel_enum/1 -> VDDM_VehMalfunLevel_enum_Inproc/1  "VDDM_VehMalfunLevel_enum"
  VDDM_VehMalfunLevel_enum_Inproc/1 -> UnitConverter405/1
  UnitConverter405/1 -> VOUTP_VehMalfunLevel_enum/1  "VOUTP_VehMalfunLevel_enum"
  VDDM_APS1SigOoRDTC_raw32/1 -> VDDM_APS1SigOoRDTC_raw32_Inproc/1  "VDDM_APS1SigOoRDTC_raw32"
  VDDM_APS1SigOoRDTC_raw32_Inproc/1 -> UnitConverter406/1
  UnitConverter406/1 -> VOUTP_APS1SigOoRDTC_raw32/1  "VOUTP_APS1SigOoRDTC_raw32"
  VDDM_APS2SigOoRDTC_raw32/1 -> VDDM_APS2SigOoRDTC_raw32_Inproc/1  "VDDM_APS2SigOoRDTC_raw32"
  VDDM_APS2SigOoRDTC_raw32_Inproc/1 -> UnitConverter407/1
  UnitConverter407/1 -> VOUTP_APS2SigOoRDTC_raw32/1  "VOUTP_APS2SigOoRDTC_raw32"
  VDDM_APSCorrErrDTC_raw32/1 -> VDDM_APSCorrErrDTC_raw32_Inproc/1  "VDDM_APSCorrErrDTC_raw32"
  VDDM_APSCorrErrDTC_raw32_Inproc/1 -> UnitConverter408/1
  UnitConverter408/1 -> VOUTP_APSCorrErrDTC_raw32/1  "VOUTP_APSCorrErrDTC_raw32"
  VDDM_MCUF1NoComDTC_raw32/1 -> VDDM_MCUF1NoComDTC_raw32_Inproc/1  "VDDM_MCUF1NoComDTC_raw32"
  VDDM_MCUF1NoComDTC_raw32_Inproc/1 -> UnitConverter409/1
  UnitConverter409/1 -> VOUTP_MCUF1NoComDTC_raw32/1  "VOUTP_MCUF1NoComDTC_raw32"
  VDDM_MCUR1NoComDTC_raw32/1 -> VDDM_MCUR1NoComDTC_raw32_Inproc/1  "VDDM_MCUR1NoComDTC_raw32"
  VDDM_MCUR1NoComDTC_raw32_Inproc/1 -> UnitConverter410/1
  UnitConverter410/1 -> VOUTP_MCUR1NoComDTC_raw32/1  "VOUTP_MCUR1NoComDTC_raw32"
  VDDM_Shifter1NoComDTC_raw32/1 -> VDDM_Shifter1NoComDTC_raw32_Inproc/1  "VDDM_Shifter1NoComDTC_raw32"
  VDDM_Shifter1NoComDTC_raw32_Inproc/1 -> UnitConverter411/1
  UnitConverter411/1 -> VOUTP_Shifter1NoComDTC_raw32/1  "VOUTP_Shifter1NoComDTC_raw32"
  VDDM_ESC7NoComDTC_raw32/1 -> VDDM_ESC7NoComDTC_raw32_Inproc/1  "VDDM_ESC7NoComDTC_raw32"
  VDDM_ESC7NoComDTC_raw32_Inproc/1 -> UnitConverter412/1
  UnitConverter412/1 -> VOUTP_ESC7NoComDTC_raw32/1  "VOUTP_ESC7NoComDTC_raw32"
  VDDM_ESC1NoComDTC_raw32/1 -> VDDM_ESC1NoComDTC_raw32_Inproc/1  "VDDM_ESC1NoComDTC_raw32"
  VDDM_ESC1NoComDTC_raw32_Inproc/1 -> UnitConverter413/1
  UnitConverter413/1 -> VOUTP_ESC1NoComDTC_raw32/1  "VOUTP_ESC1NoComDTC_raw32"
  VDDM_ESC5NoComDTC_raw32/1 -> VDDM_ESC5NoComDTC_raw32_Inproc/1  "VDDM_ESC5NoComDTC_raw32"
  VDDM_ESC5NoComDTC_raw32_Inproc/1 -> UnitConverter414/1
  UnitConverter414/1 -> VOUTP_ESC5NoComDTC_raw32/1  "VOUTP_ESC5NoComDTC_raw32"
  VDDM_EnterNewOperCyc_flg/1 -> VDDM_EnterNewOperCyc_flg_Inproc/1  "VDDM_EnterNewOperCyc_flg"
  VDDM_EnterNewOperCyc_flg_Inproc/1 -> UnitConverter415/1
  UnitConverter415/1 -> VOUTP_EnterNewOperCyc_flg/1  "VOUTP_EnterNewOperCyc_flg"
  VDDM_DiagHCrashDTC_raw32/1 -> VDDM_DiagHCrashDTC_raw32_Inproc/1  "VDDM_DiagHCrashDTC_raw32"
  VDDM_DiagHCrashDTC_raw32_Inproc/1 -> UnitConverter416/1
  UnitConverter416/1 -> VOUTP_DiagHCrashDTC_raw32/1  "VOUTP_DiagHCrashDTC_raw32"
  VDDM_DiagFLTSDTC_raw32/1 -> VDDM_DiagFLTSDTC_raw32_Inproc/1  "VDDM_DiagFLTSDTC_raw32"
  VDDM_DiagFLTSDTC_raw32_Inproc/1 -> UnitConverter417/1
  UnitConverter417/1 -> VOUTP_DiagFLTSDTC_raw32/1  "VOUTP_DiagFLTSDTC_raw32"
  VDDM_DiagFRTSDTC_raw32/1 -> VDDM_DiagFRTSDTC_raw32_Inproc/1  "VDDM_DiagFRTSDTC_raw32"
  VDDM_DiagFRTSDTC_raw32_Inproc/1 -> UnitConverter418/1
  UnitConverter418/1 -> VOUTP_DiagFRTSDTC_raw32/1  "VOUTP_DiagFRTSDTC_raw32"
  VDDM_DiagRLTSDTC_raw32/1 -> VDDM_DiagRLTSDTC_raw32_Inproc/1  "VDDM_DiagRLTSDTC_raw32"
  VDDM_DiagRLTSDTC_raw32_Inproc/1 -> UnitConverter419/1
  UnitConverter419/1 -> VOUTP_DiagRLTSDTC_raw32/1  "VOUTP_DiagRLTSDTC_raw32"
  VDDM_DiagRRTSDTC_raw32/1 -> VDDM_DiagRRTSDTC_raw32_Inproc/1  "VDDM_DiagRRTSDTC_raw32"
  VDDM_DiagRRTSDTC_raw32_Inproc/1 -> UnitConverter420/1
  UnitConverter420/1 -> VOUTP_DiagRRTSDTC_raw32/1  "VOUTP_DiagRRTSDTC_raw32"
  VDDM_FCLUSSDTC_raw32/1 -> VDDM_FCLUSSDTC_raw32_Inproc/1  "VDDM_FCLUSSDTC_raw32"
  VDDM_FCLUSSDTC_raw32_Inproc/1 -> UnitConverter421/1
  UnitConverter421/1 -> VOUTP_FCLUSSDTC_raw32/1  "VOUTP_FCLUSSDTC_raw32"
  VDDM_FMLUSSDTC_raw32/1 -> VDDM_FMLUSSDTC_raw32_Inproc/1  "VDDM_FMLUSSDTC_raw32"
  VDDM_FMLUSSDTC_raw32_Inproc/1 -> UnitConverter422/1
  UnitConverter422/1 -> VOUTP_FMLUSSDTC_raw32/1  "VOUTP_FMLUSSDTC_raw32"
  VDDM_FMRUSSDTC_raw32/1 -> VDDM_FMRUSSDTC_raw32_Inproc/1  "VDDM_FMRUSSDTC_raw32"
  VDDM_FMRUSSDTC_raw32_Inproc/1 -> UnitConverter423/1
  UnitConverter423/1 -> VOUTP_FMRUSSDTC_raw32/1  "VOUTP_FMRUSSDTC_raw32"
  VDDM_FCRUSSDTC_raw32/1 -> VDDM_FCRUSSDTC_raw32_Inproc/1  "VDDM_FCRUSSDTC_raw32"
  VDDM_FCRUSSDTC_raw32_Inproc/1 -> UnitConverter424/1
  UnitConverter424/1 -> VOUTP_FCRUSSDTC_raw32/1  "VOUTP_FCRUSSDTC_raw32"
  VDDM_RCLUSSDTC_raw32/1 -> VDDM_RCLUSSDTC_raw32_Inproc/1  "VDDM_RCLUSSDTC_raw32"
  VDDM_RCLUSSDTC_raw32_Inproc/1 -> UnitConverter425/1
  UnitConverter425/1 -> VOUTP_RCLUSSDTC_raw32/1  "VOUTP_RCLUSSDTC_raw32"
  VDDM_RMLUSSDTC_raw32/1 -> VDDM_RMLUSSDTC_raw32_Inproc/1  "VDDM_RMLUSSDTC_raw32"
  VDDM_RMLUSSDTC_raw32_Inproc/1 -> UnitConverter426/1
  UnitConverter426/1 -> VOUTP_RMLUSSDTC_raw32/1  "VOUTP_RMLUSSDTC_raw32"
  VDDM_RMRUSSDTC_raw32/1 -> VDDM_RMRUSSDTC_raw32_Inproc/1  "VDDM_RMRUSSDTC_raw32"
  VDDM_RMRUSSDTC_raw32_Inproc/1 -> UnitConverter427/1
  UnitConverter427/1 -> VOUTP_RMRUSSDTC_raw32/1  "VOUTP_RMRUSSDTC_raw32"
  VDDM_RCRUSSDTC_raw32/1 -> VDDM_RCRUSSDTC_raw32_Inproc/1  "VDDM_RCRUSSDTC_raw32"
  VDDM_RCRUSSDTC_raw32_Inproc/1 -> UnitConverter428/1
  UnitConverter428/1 -> VOUTP_RCRUSSDTC_raw32/1  "VOUTP_RCRUSSDTC_raw32"
  VDDM_FLLUSSDTC_raw32/1 -> VDDM_FLLUSSDTC_raw32_Inproc/1  "VDDM_FLLUSSDTC_raw32"
  VDDM_FLLUSSDTC_raw32_Inproc/1 -> UnitConverter429/1
  UnitConverter429/1 -> VOUTP_FLLUSSDTC_raw32/1  "VOUTP_FLLUSSDTC_raw32"
  VDDM_FLRUSSDTC_raw32/1 -> VDDM_FLRUSSDTC_raw32_Inproc/1  "VDDM_FLRUSSDTC_raw32"
  VDDM_FLRUSSDTC_raw32_Inproc/1 -> UnitConverter430/1
  UnitConverter430/1 -> VOUTP_FLRUSSDTC_raw32/1  "VOUTP_FLRUSSDTC_raw32"
  VDDM_RLLUSSDTC_raw32/1 -> VDDM_RLLUSSDTC_raw32_Inproc/1  "VDDM_RLLUSSDTC_raw32"
  VDDM_RLLUSSDTC_raw32_Inproc/1 -> UnitConverter431/1
  UnitConverter431/1 -> VOUTP_RLLUSSDTC_raw32/1  "VOUTP_RLLUSSDTC_raw32"
  VDDM_RLRUSSDTC_raw32/1 -> VDDM_RLRUSSDTC_raw32_Inproc/1  "VDDM_RLRUSSDTC_raw32"
  VDDM_RLRUSSDTC_raw32_Inproc/1 -> UnitConverter432/1
  UnitConverter432/1 -> VOUTP_RLRUSSDTC_raw32/1  "VOUTP_RLRUSSDTC_raw32"
  VDDM_FCM2NoComDTC_raw32/1 -> VDDM_FCM2NoComDTC_raw32_Inproc/1  "VDDM_FCM2NoComDTC_raw32"
  VDDM_FCM2NoComDTC_raw32_Inproc/1 -> UnitConverter433/1
  UnitConverter433/1 -> VOUTP_FCM2NoComDTC_raw32/1  "VOUTP_FCM2NoComDTC_raw32"
  VDDM_FCM2RCErrDTC_raw32/1 -> VDDM_FCM2RCErrDTC_raw32_Inproc/1  "VDDM_FCM2RCErrDTC_raw32"
  VDDM_FCM2RCErrDTC_raw32_Inproc/1 -> UnitConverter434/1
  UnitConverter434/1 -> VOUTP_FCM2RCErrDTC_raw32/1  "VOUTP_FCM2RCErrDTC_raw32"
  VDDM_FCM2CSErrDTC_raw32/1 -> VDDM_FCM2CSErrDTC_raw32_Inproc/1  "VDDM_FCM2CSErrDTC_raw32"
  VDDM_FCM2CSErrDTC_raw32_Inproc/1 -> UnitConverter435/1
  UnitConverter435/1 -> VOUTP_FCM2CSErrDTC_raw32/1  "VOUTP_FCM2CSErrDTC_raw32"
  VDDM_FCM3NoComDTC_raw32/1 -> VDDM_FCM3NoComDTC_raw32_Inproc/1  "VDDM_FCM3NoComDTC_raw32"
  VDDM_FCM3NoComDTC_raw32_Inproc/1 -> UnitConverter436/1
  UnitConverter436/1 -> VOUTP_FCM3NoComDTC_raw32/1  "VOUTP_FCM3NoComDTC_raw32"
  VDDM_FCM3RCErrDTC_raw32/1 -> VDDM_FCM3RCErrDTC_raw32_Inproc/1  "VDDM_FCM3RCErrDTC_raw32"
  VDDM_FCM3RCErrDTC_raw32_Inproc/1 -> UnitConverter437/1
  UnitConverter437/1 -> VOUTP_FCM3RCErrDTC_raw32/1  "VOUTP_FCM3RCErrDTC_raw32"
  VDDM_FCM3CSErrDTC_raw32/1 -> VDDM_FCM3CSErrDTC_raw32_Inproc/1  "VDDM_FCM3CSErrDTC_raw32"
  VDDM_FCM3CSErrDTC_raw32_Inproc/1 -> UnitConverter438/1
  UnitConverter438/1 -> VOUTP_FCM3CSErrDTC_raw32/1  "VOUTP_FCM3CSErrDTC_raw32"
  VDDM_FCM4NoComDTC_raw32/1 -> VDDM_FCM4NoComDTC_raw32_Inproc/1  "VDDM_FCM4NoComDTC_raw32"
  VDDM_FCM4NoComDTC_raw32_Inproc/1 -> UnitConverter439/1
  UnitConverter439/1 -> VOUTP_FCM4NoComDTC_raw32/1  "VOUTP_FCM4NoComDTC_raw32"
  VDDM_FCM4CSErrDTC_raw32/1 -> VDDM_FCM4CSErrDTC_raw32_Inproc/1  "VDDM_FCM4CSErrDTC_raw32"
  VDDM_FCM4CSErrDTC_raw32_Inproc/1 -> UnitConverter440/1
  UnitConverter440/1 -> VOUTP_FCM4CSErrDTC_raw32/1  "VOUTP_FCM4CSErrDTC_raw32"
  VDDM_FCM5NoComDTC_raw32/1 -> VDDM_FCM5NoComDTC_raw32_Inproc/1  "VDDM_FCM5NoComDTC_raw32"
  VDDM_FCM5NoComDTC_raw32_Inproc/1 -> UnitConverter441/1
  UnitConverter441/1 -> VOUTP_FCM5NoComDTC_raw32/1  "VOUTP_FCM5NoComDTC_raw32"
  VDDM_FCM5CSErrDTC_raw32/1 -> VDDM_FCM5CSErrDTC_raw32_Inproc/1  "VDDM_FCM5CSErrDTC_raw32"
  VDDM_FCM5CSErrDTC_raw32_Inproc/1 -> UnitConverter442/1
  UnitConverter442/1 -> VOUTP_FCM5CSErrDTC_raw32/1  "VOUTP_FCM5CSErrDTC_raw32"
  VDDM_ZoneSCPNoComDTC_raw32/1 -> VDDM_ZoneSCPNoComDTC_raw32_Inproc/1  "VDDM_ZoneSCPNoComDTC_raw32"
  VDDM_ZoneSCPNoComDTC_raw32_Inproc/1 -> UnitConverter443/1
  UnitConverter443/1 -> VOUTP_ZoneSCPNoComDTC_raw32/1  "VOUTP_ZoneSCPNoComDTC_raw32"
  VDDM_BMSSigErrDetDTC_raw32/1 -> VDDM_BMSSigErrDetDTC_raw32_Inproc/1  "VDDM_BMSSigErrDetDTC_raw32"
  VDDM_BMSSigErrDetDTC_raw32_Inproc/1 -> UnitConverter444/1
  UnitConverter444/1 -> VOUTP_BMSSigErrDetDTC_raw32/1  "VOUTP_BMSSigErrDetDTC_raw32"
  VDDM_FCMACCSigErrDetDTC_raw32/1 -> VDDM_FCMACCSigErrDetDTC_raw32_Inproc/1  "VDDM_FCMACCSigErrDetDTC_raw32"
  VDDM_FCMACCSigErrDetDTC_raw32_Inproc/1 -> UnitConverter445/1
  UnitConverter445/1 -> VOUTP_FCMACCSigErrDetDTC_raw32/1  "VOUTP_FCMACCSigErrDetDTC_raw32"
  VDDM_FrMCUSigErrDetDTC_raw32/1 -> VDDM_FrMCUSigErrDetDTC_raw32_Inproc/1  "VDDM_FrMCUSigErrDetDTC_raw32"
  VDDM_FrMCUSigErrDetDTC_raw32_Inproc/1 -> UnitConverter446/1
  UnitConverter446/1 -> VOUTP_FrMCUSigErrDetDTC_raw32/1  "VOUTP_FrMCUSigErrDetDTC_raw32"
  VDDM_RrMCUSigErrDetDTC_raw32/1 -> VDDM_RrMCUSigErrDetDTC_raw32_Inproc/1  "VDDM_RrMCUSigErrDetDTC_raw32"
  VDDM_RrMCUSigErrDetDTC_raw32_Inproc/1 -> UnitConverter447/1
  UnitConverter447/1 -> VOUTP_RrMCUSigErrDetDTC_raw32/1  "VOUTP_RrMCUSigErrDetDTC_raw32"
  VDDM_CCUSigErrDetDTC_raw32/1 -> VDDM_CCUSigErrDetDTC_raw32_Inproc/1  "VDDM_CCUSigErrDetDTC_raw32"
  VDDM_CCUSigErrDetDTC_raw32_Inproc/1 -> UnitConverter448/1
  UnitConverter448/1 -> VOUTP_CCUSigErrDetDTC_raw32/1  "VOUTP_CCUSigErrDetDTC_raw32"
  VDDM_ACCAccelCmdErrDetDTC_raw32/1 -> VDDM_ACCAccelCmdErrDetDTC_raw32_Inproc/1  "VDDM_ACCAccelCmdErrDetDTC_raw32"
  VDDM_ACCAccelCmdErrDetDTC_raw32_Inproc/1 -> UnitConverter449/1
  UnitConverter449/1 -> VOUTP_ACCAccelCmdErrDetDTC_raw32/1  "VOUTP_ACCAccelCmdErrDetDTC_raw32"
  VDDM_ACCMalfuncDetDTC_raw32/1 -> VDDM_ACCMalfuncDetDTC_raw32_Inproc/1  "VDDM_ACCMalfuncDetDTC_raw32"
  VDDM_ACCMalfuncDetDTC_raw32_Inproc/1 -> UnitConverter450/1
  UnitConverter450/1 -> VOUTP_ACCMalfuncDetDTC_raw32/1  "VOUTP_ACCMalfuncDetDTC_raw32"
  VDDM_CCMalfuncDetDTC_raw32/1 -> VDDM_CCMalfuncDetDTC_raw32_Inproc/1  "VDDM_CCMalfuncDetDTC_raw32"
  VDDM_CCMalfuncDetDTC_raw32_Inproc/1 -> UnitConverter451/1
  UnitConverter451/1 -> VOUTP_CCMalfuncDetDTC_raw32/1  "VOUTP_CCMalfuncDetDTC_raw32"
  VDDM_MSAMalfuncDetDTC_raw32/1 -> VDDM_MSAMalfuncDetDTC_raw32_Inproc/1  "VDDM_MSAMalfuncDetDTC_raw32"
  VDDM_MSAMalfuncDetDTC_raw32_Inproc/1 -> UnitConverter452/1
  UnitConverter452/1 -> VOUTP_MSAMalfuncDetDTC_raw32/1  "VOUTP_MSAMalfuncDetDTC_raw32"
  VDDM_ISAMalfuncDetDTC_raw32/1 -> VDDM_ISAMalfuncDetDTC_raw32_Inproc/1  "VDDM_ISAMalfuncDetDTC_raw32"
  VDDM_ISAMalfuncDetDTC_raw32_Inproc/1 -> UnitConverter453/1
  UnitConverter453/1 -> VOUTP_ISAMalfuncDetDTC_raw32/1  "VOUTP_ISAMalfuncDetDTC_raw32"
  VDDM_MCUF1RCErrDTC_raw32/1 -> VDDM_MCUF1RCErrDTC_raw32_Inproc/1  "VDDM_MCUF1RCErrDTC_raw32"
  VDDM_MCUF1RCErrDTC_raw32_Inproc/1 -> UnitConverter454/1
  UnitConverter454/1 -> VOUTP_MCUF1RCErrDTC_raw32/1  "VOUTP_MCUF1RCErrDTC_raw32"
  VDDM_MCUR1RCErrDTC_raw32/1 -> VDDM_MCUR1RCErrDTC_raw32_Inproc/1  "VDDM_MCUR1RCErrDTC_raw32"
  VDDM_MCUR1RCErrDTC_raw32_Inproc/1 -> UnitConverter455/1
  UnitConverter455/1 -> VOUTP_MCUR1RCErrDTC_raw32/1  "VOUTP_MCUR1RCErrDTC_raw32"
  VDDM_MCUF1CSErrDTC_raw32/1 -> VDDM_MCUF1CSErrDTC_raw32_Inproc/1  "VDDM_MCUF1CSErrDTC_raw32"
  VDDM_MCUF1CSErrDTC_raw32_Inproc/1 -> UnitConverter456/1
  UnitConverter456/1 -> VOUTP_MCUF1CSErrDTC_raw32/1  "VOUTP_MCUF1CSErrDTC_raw32"
  VDDM_MCUR1CSErrDTC_raw32/1 -> VDDM_MCUR1CSErrDTC_raw32_Inproc/1  "VDDM_MCUR1CSErrDTC_raw32"
  VDDM_MCUR1CSErrDTC_raw32_Inproc/1 -> UnitConverter457/1
  UnitConverter457/1 -> VOUTP_MCUR1CSErrDTC_raw32/1  "VOUTP_MCUR1CSErrDTC_raw32"
  VDDM_Shifter1RCErrDTC_raw32/1 -> VDDM_Shifter1RCErrDTC_raw32_Inproc/1  "VDDM_Shifter1RCErrDTC_raw32"
  VDDM_Shifter1RCErrDTC_raw32_Inproc/1 -> UnitConverter458/1
  UnitConverter458/1 -> VOUTP_Shifter1RCErrDTC_raw32/1  "VOUTP_Shifter1RCErrDTC_raw32"
  VDDM_Shifter1CSErrDTC_raw32/1 -> VDDM_Shifter1CSErrDTC_raw32_Inproc/1  "VDDM_Shifter1CSErrDTC_raw32"
  VDDM_Shifter1CSErrDTC_raw32_Inproc/1 -> UnitConverter459/1
  UnitConverter459/1 -> VOUTP_Shifter1CSErrDTC_raw32/1  "VOUTP_Shifter1CSErrDTC_raw32"
  VDDM_ESC7RCErrDTC_raw32/1 -> VDDM_ESC7RCErrDTC_raw32_Inproc/1  "VDDM_ESC7RCErrDTC_raw32"
  VDDM_ESC7RCErrDTC_raw32_Inproc/1 -> UnitConverter460/1
  UnitConverter460/1 -> VOUTP_ESC7RCErrDTC_raw32/1  "VOUTP_ESC7RCErrDTC_raw32"
  VDDM_ESC7CSErrDTC_raw32/1 -> VDDM_ESC7CSErrDTC_raw32_Inproc/1  "VDDM_ESC7CSErrDTC_raw32"
  VDDM_ESC7CSErrDTC_raw32_Inproc/1 -> UnitConverter461/1
  UnitConverter461/1 -> VOUTP_ESC7CSErrDTC_raw32/1  "VOUTP_ESC7CSErrDTC_raw32"
  VDDM_ESC1RCErrDTC_raw32/1 -> VDDM_ESC1RCErrDTC_raw32_Inproc/1  "VDDM_ESC1RCErrDTC_raw32"
  VDDM_ESC1RCErrDTC_raw32_Inproc/1 -> UnitConverter462/1
  UnitConverter462/1 -> VOUTP_ESC1RCErrDTC_raw32/1  "VOUTP_ESC1RCErrDTC_raw32"
  VDDM_ESC1CSErrDTC_raw32/1 -> VDDM_ESC1CSErrDTC_raw32_Inproc/1  "VDDM_ESC1CSErrDTC_raw32"
  VDDM_ESC1CSErrDTC_raw32_Inproc/1 -> UnitConverter463/1
  UnitConverter463/1 -> VOUTP_ESC1CSErrDTC_raw32/1  "VOUTP_ESC1CSErrDTC_raw32"
  VDDM_ESC5RCErrDTC_raw32/1 -> VDDM_ESC5RCErrDTC_raw32_Inproc/1  "VDDM_ESC5RCErrDTC_raw32"
  VDDM_ESC5RCErrDTC_raw32_Inproc/1 -> UnitConverter464/1
  UnitConverter464/1 -> VOUTP_ESC5RCErrDTC_raw32/1  "VOUTP_ESC5RCErrDTC_raw32"
  VDDM_ESC5CSErrDTC_raw32/1 -> VDDM_ESC5CSErrDTC_raw32_Inproc/1  "VDDM_ESC5CSErrDTC_raw32"
  VDDM_ESC5CSErrDTC_raw32_Inproc/1 -> UnitConverter465/1
  UnitConverter465/1 -> VOUTP_ESC5CSErrDTC_raw32/1  "VOUTP_ESC5CSErrDTC_raw32"
  VDDM_FrMCUTqErrDTC_raw32/1 -> VDDM_FrMCUTqErrDTC_raw32_Inproc/1  "VDDM_FrMCUTqErrDTC_raw32"
  VDDM_FrMCUTqErrDTC_raw32_Inproc/1 -> UnitConverter466/1
  UnitConverter466/1 -> VOUTP_FrMCUTqErrDTC_raw32/1  "VOUTP_FrMCUTqErrDTC_raw32"
  VDDM_RrMCUTqErrDTC_raw32/1 -> VDDM_RrMCUTqErrDTC_raw32_Inproc/1  "VDDM_RrMCUTqErrDTC_raw32"
  VDDM_RrMCUTqErrDTC_raw32_Inproc/1 -> UnitConverter467/1
  UnitConverter467/1 -> VOUTP_RrMCUTqErrDTC_raw32/1  "VOUTP_RrMCUTqErrDTC_raw32"
  VDDM_LFBatwarnDTC_raw32/1 -> VDDM_LFBatwarnDTC_raw32_Inproc/1  "VDDM_LFBatwarnDTC_raw32"
  VDDM_LFBatwarnDTC_raw32_Inproc/1 -> UnitConverter468/1
  UnitConverter468/1 -> VOUTP_LFBatwarnDTC_raw32/1  "VOUTP_LFBatwarnDTC_raw32"
  VDDM_RFBatwarnDTC_raw32/1 -> VDDM_RFBatwarnDTC_raw32_Inproc/1  "VDDM_RFBatwarnDTC_raw32"
  VDDM_RFBatwarnDTC_raw32_Inproc/1 -> UnitConverter469/1
  UnitConverter469/1 -> VOUTP_RFBatwarnDTC_raw32/1  "VOUTP_RFBatwarnDTC_raw32"
  VDDM_LRBatwarnDTC_raw32/1 -> VDDM_LRBatwarnDTC_raw32_Inproc/1  "VDDM_LRBatwarnDTC_raw32"
  VDDM_LRBatwarnDTC_raw32_Inproc/1 -> UnitConverter470/1
  UnitConverter470/1 -> VOUTP_LRBatwarnDTC_raw32/1  "VOUTP_LRBatwarnDTC_raw32"
  VDDM_RRBatwarnDTC_raw32/1 -> VDDM_RRBatwarnDTC_raw32_Inproc/1  "VDDM_RRBatwarnDTC_raw32"
  VDDM_RRBatwarnDTC_raw32_Inproc/1 -> UnitConverter471/1
  UnitConverter471/1 -> VOUTP_RRBatwarnDTC_raw32/1  "VOUTP_RRBatwarnDTC_raw32"
  VDDM_LFPressIndiDTC_raw32/1 -> VDDM_LFPressIndiDTC_raw32_Inproc/1  "VDDM_LFPressIndiDTC_raw32"
  VDDM_LFPressIndiDTC_raw32_Inproc/1 -> UnitConverter472/1
  UnitConverter472/1 -> VOUTP_LFPressIndiDTC_raw32/1  "VOUTP_LFPressIndiDTC_raw32"
  VDDM_RFPressIndiDTC_raw32/1 -> VDDM_RFPressIndiDTC_raw32_Inproc/1  "VDDM_RFPressIndiDTC_raw32"
  VDDM_RFPressIndiDTC_raw32_Inproc/1 -> UnitConverter473/1
  UnitConverter473/1 -> VOUTP_RFPressIndiDTC_raw32/1  "VOUTP_RFPressIndiDTC_raw32"
  VDDM_LRPressIndiDTC_raw32/1 -> VDDM_LRPressIndiDTC_raw32_Inproc/1  "VDDM_LRPressIndiDTC_raw32"
  VDDM_LRPressIndiDTC_raw32_Inproc/1 -> UnitConverter474/1
  UnitConverter474/1 -> VOUTP_LRPressIndiDTC_raw32/1  "VOUTP_LRPressIndiDTC_raw32"
  VDDM_RRPressIndiDTC_raw32/1 -> VDDM_RRPressIndiDTC_raw32_Inproc/1  "VDDM_RRPressIndiDTC_raw32"
  VDDM_RRPressIndiDTC_raw32_Inproc/1 -> UnitConverter475/1
  UnitConverter475/1 -> VOUTP_RRPressIndiDTC_raw32/1  "VOUTP_RRPressIndiDTC_raw32"
  VDDM_LFWheelTmpHighDTC_raw32/1 -> VDDM_LFWheelTmpHighDTC_raw32_Inproc/1  "VDDM_LFWheelTmpHighDTC_raw32"
  VDDM_LFWheelTmpHighDTC_raw32_Inproc/1 -> UnitConverter476/1
  UnitConverter476/1 -> VOUTP_LFWheelTmpHighDTC_raw32/1  "VOUTP_LFWheelTmpHighDTC_raw32"
  VDDM_RFWheelTmpHighDTC_raw32/1 -> VDDM_RFWheelTmpHighDTC_raw32_Inproc/1  "VDDM_RFWheelTmpHighDTC_raw32"
  VDDM_RFWheelTmpHighDTC_raw32_Inproc/1 -> UnitConverter477/1
  UnitConverter477/1 -> VOUTP_RFWheelTmpHighDTC_raw32/1  "VOUTP_RFWheelTmpHighDTC_raw32"
  VDDM_LRWheelTmpHighDTC_raw32/1 -> VDDM_LRWheelTmpHighDTC_raw32_Inproc/1  "VDDM_LRWheelTmpHighDTC_raw32"
  VDDM_LRWheelTmpHighDTC_raw32_Inproc/1 -> UnitConverter478/1
  UnitConverter478/1 -> VOUTP_LRWheelTmpHighDTC_raw32/1  "VOUTP_LRWheelTmpHighDTC_raw32"
  VDDM_RRWheelTmpHighDTC_raw32/1 -> VDDM_RRWheelTmpHighDTC_raw32_Inproc/1  "VDDM_RRWheelTmpHighDTC_raw32"
  VDDM_RRWheelTmpHighDTC_raw32_Inproc/1 -> UnitConverter479/1
  UnitConverter479/1 -> VOUTP_RRWheelTmpHighDTC_raw32/1  "VOUTP_RRWheelTmpHighDTC_raw32"
  VDDM_LFSensorFailDTC_raw32/1 -> VDDM_LFSensorFailDTC_raw32_Inproc/1  "VDDM_LFSensorFailDTC_raw32"
  VDDM_LFSensorFailDTC_raw32_Inproc/1 -> UnitConverter480/1
  UnitConverter480/1 -> VOUTP_LFSensorFailDTC_raw32/1  "VOUTP_LFSensorFailDTC_raw32"
  VDDM_RFSensorFailDTC_raw32/1 -> VDDM_RFSensorFailDTC_raw32_Inproc/1  "VDDM_RFSensorFailDTC_raw32"
  VDDM_RFSensorFailDTC_raw32_Inproc/1 -> UnitConverter481/1
  UnitConverter481/1 -> VOUTP_RFSensorFailDTC_raw32/1  "VOUTP_RFSensorFailDTC_raw32"
  VDDM_LRSensorFailDTC_raw32/1 -> VDDM_LRSensorFailDTC_raw32_Inproc/1  "VDDM_LRSensorFailDTC_raw32"
  VDDM_LRSensorFailDTC_raw32_Inproc/1 -> UnitConverter482/1
  UnitConverter482/1 -> VOUTP_LRSensorFailDTC_raw32/1  "VOUTP_LRSensorFailDTC_raw32"
  VDDM_RRSensorFailDTC_raw32/1 -> VDDM_RRSensorFailDTC_raw32_Inproc/1  "VDDM_RRSensorFailDTC_raw32"
  VDDM_RRSensorFailDTC_raw32_Inproc/1 -> UnitConverter483/1
  UnitConverter483/1 -> VOUTP_RRSensorFailDTC_raw32/1  "VOUTP_RRSensorFailDTC_raw32"
  VDDM_C1EPAS2LCDTC_raw32/1 -> VDDM_C1EPAS2LCDTC_raw32_Inproc/1  "VDDM_C1EPAS2LCDTC_raw32"
  VDDM_C1EPAS2LCDTC_raw32_Inproc/1 -> UnitConverter484/1
  UnitConverter484/1 -> VOUTP_C1EPAS2LCDTC_raw32/1  "VOUTP_C1EPAS2LCDTC_raw32"
  VDDM_5vAPS1PwrErrDTC_raw32/1 -> VDDM_5vAPS1PwrErrDTC_raw32_Inproc/1  "VDDM_5vAPS1PwrErrDTC_raw32"
  VDDM_5vAPS1PwrErrDTC_raw32_Inproc/1 -> UnitConverter485/1
  UnitConverter485/1 -> VOUTP_5vAPS1PwrErrDTC_raw32/1  "VOUTP_5vAPS1PwrErrDTC_raw32"
  VDDM_5vAPS2PwrErrDTC_raw32/1 -> VDDM_5vAPS2PwrErrDTC_raw32_Inproc/1  "VDDM_5vAPS2PwrErrDTC_raw32"
  VDDM_5vAPS2PwrErrDTC_raw32_Inproc/1 -> UnitConverter486/1
  UnitConverter486/1 -> VOUTP_5vAPS2PwrErrDTC_raw32/1  "VOUTP_5vAPS2PwrErrDTC_raw32"
  VDDM_EPBLockTODTC_raw32/1 -> VDDM_EPBLockTODTC_raw32_Inproc/1  "VDDM_EPBLockTODTC_raw32"
  VDDM_EPBLockTODTC_raw32_Inproc/1 -> UnitConverter487/1
  UnitConverter487/1 -> VOUTP_EPBLockTODTC_raw32/1  "VOUTP_EPBLockTODTC_raw32"
  VDDM_EPBUnlockTODTC_raw32/1 -> VDDM_EPBUnlockTODTC_raw32_Inproc/1  "VDDM_EPBUnlockTODTC_raw32"
  VDDM_EPBUnlockTODTC_raw32_Inproc/1 -> UnitConverter488/1
  UnitConverter488/1 -> VOUTP_EPBUnlockTODTC_raw32/1  "VOUTP_EPBUnlockTODTC_raw32"
  VDDM_LimpHomeActTmp_flg/1 -> VDDM_LimpHomeActTmp_flg_Inproc/1  "VDDM_LimpHomeActTmp_flg"
  VDDM_LimpHomeActTmp_flg_Inproc/1 -> UnitConverter489/1
  UnitConverter489/1 -> VOUTP_LimpHomeActTmp_flg/1  "VOUTP_LimpHomeActTmp_flg"
  VDDM_DTCDetect_enum/1 -> VDDM_DTCDetect_enum_Inproc/1  "VDDM_DTCDetect_enum"
  VDDM_DTCDetect_enum_Inproc/1 -> UnitConverter490/1
  UnitConverter490/1 -> VOUTP_DTCDetect_enum/1  "VOUTP_DTCDetect_enum"
  VDDM_EngagePFail_flg/1 -> VDDM_EngagePFail_flg_Inproc/1  "VDDM_EngagePFail_flg"
  VDDM_EngagePFail_flg_Inproc/1 -> UnitConverter491/1
  UnitConverter491/1 -> VOUTP_EngagePFail_flg/1  "VOUTP_EngagePFail_flg"
  VDDM_DisengagePFail_flg/1 -> VDDM_DisengagePFail_flg_Inproc/1  "VDDM_DisengagePFail_flg"
  VDDM_DisengagePFail_flg_Inproc/1 -> UnitConverter492/1
  UnitConverter492/1 -> VOUTP_DisengagePFail_flg/1  "VOUTP_DisengagePFail_flg"
  VDDM_VCURAPSErrLv2_flg/1 -> VDDM_VCURAPSErrLv2_flg_Inproc/1  "VDDM_VCURAPSErrLv2_flg"
  VDDM_VCURAPSErrLv2_flg_Inproc/1 -> UnitConverter493/1
  UnitConverter493/1 -> VOUTP_VCURAPSErrLv2_flg/1  "VOUTP_VCURAPSErrLv2_flg"
  VDDM_VCURAPSErrLv3_flg/1 -> VDDM_VCURAPSErrLv3_flg_Inproc/1  "VDDM_VCURAPSErrLv3_flg"
  VDDM_VCURAPSErrLv3_flg_Inproc/1 -> UnitConverter494/1
  UnitConverter494/1 -> VOUTP_VCURAPSErrLv3_flg/1  "VOUTP_VCURAPSErrLv3_flg"
  VDDM_EDriveSysErrShifterErr_flg/1 -> VDDM_EDriveSysErrShifterErr_flg_Inproc/1  "VDDM_EDriveSysErrShifterErr_flg"
  VDDM_EDriveSysErrShifterErr_flg_Inproc/1 -> UnitConverter495/1
  UnitConverter495/1 -> VOUTP_EDriveSysErrShifterErr_flg/1  "VOUTP_EDriveSysErrShifterErr_flg"
  VDDM_LVSysErrPwrOutErr_flg/1 -> VDDM_LVSysErrPwrOutErr_flg_Inproc/1  "VDDM_LVSysErrPwrOutErr_flg"
  VDDM_LVSysErrPwrOutErr_flg_Inproc/1 -> UnitConverter496/1
  UnitConverter496/1 -> VOUTP_LVSysErrPwrOutErr_flg/1  "VOUTP_LVSysErrPwrOutErr_flg"
  VDDM_HVRlyOpFail_flg/1 -> VDDM_HVRlyOpFail_flg_Inproc/1  "VDDM_HVRlyOpFail_flg"
  VDDM_HVRlyOpFail_flg_Inproc/1 -> UnitConverter497/1
  UnitConverter497/1 -> VOUTP_HVRlyOpFail_flg/1  "VOUTP_HVRlyOpFail_flg"
  VDDM_MCUActDisFail_flg/1 -> VDDM_MCUActDisFail_flg_Inproc/1  "VDDM_MCUActDisFail_flg"
  VDDM_MCUActDisFail_flg_Inproc/1 -> UnitConverter498/1
  UnitConverter498/1 -> VOUTP_MCUActDisFail_flg/1  "VOUTP_MCUActDisFail_flg"
  VDDM_VCUBrkSWSta_enum/1 -> VDDM_VCUBrkSWSta_enum_Inproc/1  "VDDM_VCUBrkSWSta_enum"
  VDDM_VCUBrkSWSta_enum_Inproc/1 -> UnitConverter499/1
  UnitConverter499/1 -> VOUTP_VCUBrkSWSta_enum/1  "VOUTP_VCUBrkSWSta_enum"
  VDDM_VCUFLDoorSta_flg/1 -> VDDM_VCUFLDoorSta_flg_Inproc/1  "VDDM_VCUFLDoorSta_flg"
  VDDM_VCUFLDoorSta_flg_Inproc/1 -> UnitConverter500/1
  UnitConverter500/1 -> VOUTP_VCUFLDoorSta_flg/1  "VOUTP_VCUFLDoorSta_flg"
  VDDM_VCUFRDoorSta_flg/1 -> VDDM_VCUFRDoorSta_flg_Inproc/1  "VDDM_VCUFRDoorSta_flg"
  VDDM_VCUFRDoorSta_flg_Inproc/1 -> UnitConverter501/1
  UnitConverter501/1 -> VOUTP_VCUFRDoorSta_flg/1  "VOUTP_VCUFRDoorSta_flg"
  VDDM_VCURLDoorSta_flg/1 -> VDDM_VCURLDoorSta_flg_Inproc/1  "VDDM_VCURLDoorSta_flg"
  VDDM_VCURLDoorSta_flg_Inproc/1 -> UnitConverter502/1
  UnitConverter502/1 -> VOUTP_VCURLDoorSta_flg/1  "VOUTP_VCURLDoorSta_flg"
  VDDM_VCURRDoorSta_flg/1 -> VDDM_VCURRDoorSta_flg_Inproc/1  "VDDM_VCURRDoorSta_flg"
  VDDM_VCURRDoorSta_flg_Inproc/1 -> UnitConverter503/1
  UnitConverter503/1 -> VOUTP_VCURRDoorSta_flg/1  "VOUTP_VCURRDoorSta_flg"
  VDDM_SysAllowReadySta_flg/1 -> VDDM_SysAllowReadySta_flg_Inproc/1  "VDDM_SysAllowReadySta_flg"
  VDDM_SysAllowReadySta_flg_Inproc/1 -> UnitConverter504/1
  UnitConverter504/1 -> VOUTP_SysAllowReadySta_flg/1  "VOUTP_SysAllowReadySta_flg"
  VDDM_VCUHoodSWSta_flg/1 -> VDDM_VCUHoodSWSta_flg_Inproc/1  "VDDM_VCUHoodSWSta_flg"
  VDDM_VCUHoodSWSta_flg_Inproc/1 -> UnitConverter505/1
  UnitConverter505/1 -> VOUTP_VCUHoodSWSta_flg/1  "VOUTP_VCUHoodSWSta_flg"
  VDDM_VCUTailgateSWSta_flg/1 -> VDDM_VCUTailgateSWSta_flg_Inproc/1  "VDDM_VCUTailgateSWSta_flg"
  VDDM_VCUTailgateSWSta_flg_Inproc/1 -> UnitConverter506/1
  UnitConverter506/1 -> VOUTP_VCUTailgateSWSta_flg/1  "VOUTP_VCUTailgateSWSta_flg"
  VDDM_CAN1BusErrorDTC_raw32/1 -> VDDM_CAN1BusErrorDTC_raw32_Inproc/1  "VDDM_CAN1BusErrorDTC_raw32"
  VDDM_CAN1BusErrorDTC_raw32_Inproc/1 -> UnitConverter507/1
  UnitConverter507/1 -> VOUTP_CAN1BusErrorDTC_raw32/1  "VOUTP_CAN1BusErrorDTC_raw32"
  VDDM_CAN2BusErrorDTC_raw32/1 -> VDDM_CAN2BusErrorDTC_raw32_Inproc/1  "VDDM_CAN2BusErrorDTC_raw32"
  VDDM_CAN2BusErrorDTC_raw32_Inproc/1 -> UnitConverter508/1
  UnitConverter508/1 -> VOUTP_CAN2BusErrorDTC_raw32/1  "VOUTP_CAN2BusErrorDTC_raw32"
  VDDM_CAN3BusErrorDTC_raw32/1 -> VDDM_CAN3BusErrorDTC_raw32_Inproc/1  "VDDM_CAN3BusErrorDTC_raw32"
  VDDM_CAN3BusErrorDTC_raw32_Inproc/1 -> UnitConverter509/1
  UnitConverter509/1 -> VOUTP_CAN3BusErrorDTC_raw32/1  "VOUTP_CAN3BusErrorDTC_raw32"
  VDDM_CAN4BusErrorDTC_raw32/1 -> VDDM_CAN4BusErrorDTC_raw32_Inproc/1  "VDDM_CAN4BusErrorDTC_raw32"
  VDDM_CAN4BusErrorDTC_raw32_Inproc/1 -> UnitConverter510/1
  UnitConverter510/1 -> VOUTP_CAN4BusErrorDTC_raw32/1  "VOUTP_CAN4BusErrorDTC_raw32"
  VDDM_CAN5BusErrorDTC_raw32/1 -> VDDM_CAN5BusErrorDTC_raw32_Inproc/1  "VDDM_CAN5BusErrorDTC_raw32"
  VDDM_CAN5BusErrorDTC_raw32_Inproc/1 -> UnitConverter511/1
  UnitConverter511/1 -> VOUTP_CAN5BusErrorDTC_raw32/1  "VOUTP_CAN5BusErrorDTC_raw32"
  VDDM_CAN6BusErrorDTC_raw32/1 -> VDDM_CAN6BusErrorDTC_raw32_Inproc/1  "VDDM_CAN6BusErrorDTC_raw32"
  VDDM_CAN6BusErrorDTC_raw32_Inproc/1 -> UnitConverter512/1
  UnitConverter512/1 -> VOUTP_CAN6BusErrorDTC_raw32/1  "VOUTP_CAN6BusErrorDTC_raw32"
  VDDM_CAN1BusOffDTC_raw32/1 -> VDDM_CAN1BusOffDTC_raw32_Inproc/1  "VDDM_CAN1BusOffDTC_raw32"
  VDDM_CAN1BusOffDTC_raw32_Inproc/1 -> UnitConverter513/1
  UnitConverter513/1 -> VOUTP_CAN1BusOffDTC_raw32/1  "VOUTP_CAN1BusOffDTC_raw32"
  VDDM_CAN2BusOffDTC_raw32/1 -> VDDM_CAN2BusOffDTC_raw32_Inproc/1  "VDDM_CAN2BusOffDTC_raw32"
  VDDM_CAN2BusOffDTC_raw32_Inproc/1 -> UnitConverter514/1
  UnitConverter514/1 -> VOUTP_CAN2BusOffDTC_raw32/1  "VOUTP_CAN2BusOffDTC_raw32"
  VDDM_CAN3BusOffDTC_raw32/1 -> VDDM_CAN3BusOffDTC_raw32_Inproc/1  "VDDM_CAN3BusOffDTC_raw32"
  VDDM_CAN3BusOffDTC_raw32_Inproc/1 -> UnitConverter515/1
  UnitConverter515/1 -> VOUTP_CAN3BusOffDTC_raw32/1  "VOUTP_CAN3BusOffDTC_raw32"
  VDDM_CAN4BusOffDTC_raw32/1 -> VDDM_CAN4BusOffDTC_raw32_Inproc/1  "VDDM_CAN4BusOffDTC_raw32"
  VDDM_CAN4BusOffDTC_raw32_Inproc/1 -> UnitConverter516/1
  UnitConverter516/1 -> VOUTP_CAN4BusOffDTC_raw32/1  "VOUTP_CAN4BusOffDTC_raw32"
  VDDM_CAN5BusOffDTC_raw32/1 -> VDDM_CAN5BusOffDTC_raw32_Inproc/1  "VDDM_CAN5BusOffDTC_raw32"
  VDDM_CAN5BusOffDTC_raw32_Inproc/1 -> UnitConverter517/1
  UnitConverter517/1 -> VOUTP_CAN5BusOffDTC_raw32/1  "VOUTP_CAN5BusOffDTC_raw32"
  VDDM_CAN6BusOffDTC_raw32/1 -> VDDM_CAN6BusOffDTC_raw32_Inproc/1  "VDDM_CAN6BusOffDTC_raw32"
  VDDM_CAN6BusOffDTC_raw32_Inproc/1 -> UnitConverter518/1
  UnitConverter518/1 -> VOUTP_CAN6BusOffDTC_raw32/1  "VOUTP_CAN6BusOffDTC_raw32"
  VDHP_ActAPSPosn_pct/1 -> VDHP_ActAPSPosn_pct_Inproc/1  "VDHP_ActAPSPosn_pct"
  VDHP_ActAPSPosn_pct_Inproc/1 -> UnitConverter519/1
  UnitConverter519/1 -> VOUTP_ActAPSPosn_pct/1  "VOUTP_ActAPSPosn_pct"
  VDHP_EAPS1MIN_pct/1 -> VDHP_EAPS1MIN_pct_Inproc/1  "VDHP_EAPS1MIN_pct"
  VDHP_EAPS1MIN_pct_Inproc/1 -> UnitConverter520/1
  UnitConverter520/1 -> VOUTP_EAPS1MIN_pct/1  "VOUTP_EAPS1MIN_pct"
  VDHP_EAPS2MIN_pct/1 -> VDHP_EAPS2MIN_pct_Inproc/1  "VDHP_EAPS2MIN_pct"
  VDHP_EAPS2MIN_pct_Inproc/1 -> UnitConverter521/1
  UnitConverter521/1 -> VOUTP_EAPS2MIN_pct/1  "VOUTP_EAPS2MIN_pct"
  VDHP_ResetPedalZeroPosStart_flg/1 -> VDHP_ResetPedalZeroPosStart_flg_Inproc/1  "VDHP_ResetPedalZeroPosStart_flg"
  VDHP_ResetPedalZeroPosStart_flg_Inproc/1 -> UnitConverter522/1
  UnitConverter522/1 -> VOUTP_ResetPedalZeroPosStart_flg/1  "VOUTP_ResetPedalZeroPosStart_flg"
  VDHP_EAPS1NRM_pct/1 -> VDHP_EAPS1NRM_pct_Inproc/1  "VDHP_EAPS1NRM_pct"
  VDHP_EAPS1NRM_pct_Inproc/1 -> UnitConverter523/1
  UnitConverter523/1 -> VOUTP_EAPS1NRM_pct/1  "VOUTP_EAPS1NRM_pct"
  VDHP_EAPS2NRM_pct/1 -> VDHP_EAPS2NRM_pct_Inproc/1  "VDHP_EAPS2NRM_pct"
  VDHP_EAPS2NRM_pct_Inproc/1 -> UnitConverter524/1
  UnitConverter524/1 -> VOUTP_EAPS2NRM_pct/1  "VOUTP_EAPS2NRM_pct"
  VDKC_DKCTimeSN_cnt/1 -> VDKC_DKCTimeSN_cnt_Inproc/1  "VDKC_DKCTimeSN_cnt"
  VDKC_DKCTimeSN_cnt_Inproc/1 -> UnitConverter525/1
  UnitConverter525/1 -> VOUTP_DKCTimeSN_cnt/1  "VOUTP_DKCTimeSN_cnt"
  VDKC_DKCAuthSta_enum/1 -> VDKC_DKCAuthSta_enum_Inproc/1  "VDKC_DKCAuthSta_enum"
  VDKC_DKCAuthSta_enum_Inproc/1 -> UnitConverter526/1
  UnitConverter526/1 -> VOUTP_DKCAuthSta_enum/1  "VOUTP_DKCAuthSta_enum"
  VDKC_TimeSNDKCFbk_cnt/1 -> VDKC_TimeSNDKCFbk_cnt_Inproc/1  "VDKC_TimeSNDKCFbk_cnt"
  VDKC_TimeSNDKCFbk_cnt_Inproc/1 -> UnitConverter527/1
  UnitConverter527/1 -> VOUTP_TimeSNDKCFbk_cnt/1  "VOUTP_TimeSNDKCFbk_cnt"
  VDKC_KeyMissSta_flg/1 -> VDKC_KeyMissSta_flg_Inproc/1  "VDKC_KeyMissSta_flg"
  VDKC_KeyMissSta_flg_Inproc/1 -> UnitConverter528/1
  UnitConverter528/1 -> VOUTP_KeyMissSta_flg/1  "VOUTP_KeyMissSta_flg"
  VDKC_KeyModeSta_enum/1 -> VDKC_KeyModeSta_enum_Inproc/1  "VDKC_KeyModeSta_enum"
  VDKC_KeyModeSta_enum_Inproc/1 -> UnitConverter529/1
  UnitConverter529/1 -> VOUTP_KeyModeSta_enum/1  "VOUTP_KeyModeSta_enum"
  VDKC_DkeyShowIVISta_enum/1 -> VDKC_DkeyShowIVISta_enum_Inproc/1  "VDKC_DkeyShowIVISta_enum"
  VDKC_DkeyShowIVISta_enum_Inproc/1 -> UnitConverter530/1
  UnitConverter530/1 -> VOUTP_DkeyShowIVISta_enum/1  "VOUTP_DkeyShowIVISta_enum"
  VDKC_KeyAreaPS_enum/1 -> VDKC_KeyAreaPS_enum_Inproc/1  "VDKC_KeyAreaPS_enum"
  VDKC_KeyAreaPS_enum_Inproc/1 -> UnitConverter531/1
  UnitConverter531/1 -> VOUTP_KeyAreaPS_enum/1  "VOUTP_KeyAreaPS_enum"
  VDKC_KeyAreaLockUnlock_enum/1 -> VDKC_KeyAreaLockUnlock_enum_Inproc/1  "VDKC_KeyAreaLockUnlock_enum"
  VDKC_KeyAreaLockUnlock_enum_Inproc/1 -> UnitConverter532/1
  UnitConverter532/1 -> VOUTP_KeyAreaLockUnlock_enum/1  "VOUTP_KeyAreaLockUnlock_enum"
  VDKC_PCommandToBCM_enum/1 -> VDKC_PCommandToBCM_enum_Inproc/1  "VDKC_PCommandToBCM_enum"
  VDKC_PCommandToBCM_enum_Inproc/1 -> UnitConverter533/1
  UnitConverter533/1 -> VOUTP_PCommandToBCM_enum/1  "VOUTP_PCommandToBCM_enum"
  VDKC_DKeyWelcomeSta_enum/1 -> VDKC_DKeyWelcomeSta_enum_Inproc/1  "VDKC_DKeyWelcomeSta_enum"
  VDKC_DKeyWelcomeSta_enum_Inproc/1 -> UnitConverter534/1
  UnitConverter534/1 -> VOUTP_DKeyWelcomeSta_enum/1  "VOUTP_DKeyWelcomeSta_enum"
  VDKC_KeyAreaPTG_enum/1 -> VDKC_KeyAreaPTG_enum_Inproc/1  "VDKC_KeyAreaPTG_enum"
  VDKC_KeyAreaPTG_enum_Inproc/1 -> UnitConverter535/1
  UnitConverter535/1 -> VOUTP_KeyAreaPTG_enum/1  "VOUTP_KeyAreaPTG_enum"
  VDKC_KeyAreaSPTGSta_enum/1 -> VDKC_KeyAreaSPTGSta_enum_Inproc/1  "VDKC_KeyAreaSPTGSta_enum"
  VDKC_KeyAreaSPTGSta_enum_Inproc/1 -> UnitConverter536/1
  UnitConverter536/1 -> VOUTP_KeyAreaSPTGSta_enum/1  "VOUTP_KeyAreaSPTGSta_enum"
  VDKC_UIDLowPowerSta_enum/1 -> VDKC_UIDLowPowerSta_enum_Inproc/1  "VDKC_UIDLowPowerSta_enum"
  VDKC_UIDLowPowerSta_enum_Inproc/1 -> UnitConverter537/1
  UnitConverter537/1 -> VOUTP_UIDLowPowerSta_enum/1  "VOUTP_UIDLowPowerSta_enum"
  VDKC_DkeyAreaRAPSSta_enum/1 -> VDKC_DkeyAreaRAPSSta_enum_Inproc/1  "VDKC_DkeyAreaRAPSSta_enum"
  VDKC_DkeyAreaRAPSSta_enum_Inproc/1 -> UnitConverter538/1
  UnitConverter538/1 -> VOUTP_DkeyAreaRAPSSta_enum/1  "VOUTP_DkeyAreaRAPSSta_enum"
  VDKC_ParkingModeCmd_enum/1 -> VDKC_ParkingModeCmd_enum_Inproc/1  "VDKC_ParkingModeCmd_enum"
  VDKC_ParkingModeCmd_enum_Inproc/1 -> UnitConverter539/1
  UnitConverter539/1 -> VOUTP_ParkingModeCmd_enum/1  "VOUTP_ParkingModeCmd_enum"
  VDKC_KeyNumSta_enum/1 -> VDKC_KeyNumSta_enum_Inproc/1  "VDKC_KeyNumSta_enum"
  VDKC_KeyNumSta_enum_Inproc/1 -> UnitConverter540/1
  UnitConverter540/1 -> VOUTP_KeyNumSta_enum/1  "VOUTP_KeyNumSta_enum"
  VDKC_KeyTypeSta_enum/1 -> VDKC_KeyTypeSta_enum_Inproc/1  "VDKC_KeyTypeSta_enum"
  VDKC_KeyTypeSta_enum_Inproc/1 -> UnitConverter541/1
  UnitConverter541/1 -> VOUTP_KeyTypeSta_enum/1  "VOUTP_KeyTypeSta_enum"
  VDKC_FDCDKCAllowSleep_flg/1 -> VDKC_FDCDKCAllowSleep_flg_Inproc/1  "VDKC_FDCDKCAllowSleep_flg"
  VDKC_FDCDKCAllowSleep_flg_Inproc/1 -> UnitConverter542/1
  UnitConverter542/1 -> VOUTP_FDCDKCAllowSleep_flg/1  "VOUTP_FDCDKCAllowSleep_flg"
  VDSC_DISCTurn_flg/1 -> VDSC_DISCTurn_flg_Inproc/1  "VDSC_DISCTurn_flg"
  VDSC_DISCTurn_flg_Inproc/1 -> UnitConverter543/1
  UnitConverter543/1 -> VOUTP_DISCTurn_flg/1  "VOUTP_DISCTurn_flg"
  VDSC_DISCTargetSpd_kph/1 -> VDSC_DISCTargetSpd_kph_Inproc/1  "VDSC_DISCTargetSpd_kph"
  VDSC_DISCTargetSpd_kph_Inproc/1 -> UnitConverter544/1
  UnitConverter544/1 -> VOUTP_DISCTargetSpd_kph/1  "VOUTP_DISCTargetSpd_kph"
  VDSC_DISCSta_enum/1 -> VDSC_DISCSta_enum_Inproc/1  "VDSC_DISCSta_enum"
  VDSC_DISCSta_enum_Inproc/1 -> UnitConverter545/1
  UnitConverter545/1 -> VOUTP_DISCSta_enum/1  "VOUTP_DISCSta_enum"
  VDSC_DISCButtSta_flg/1 -> VDSC_DISCButtSta_flg_Inproc/1  "VDSC_DISCButtSta_flg"
  VDSC_DISCButtSta_flg_Inproc/1 -> UnitConverter546/1
  UnitConverter546/1 -> VOUTP_DISCButtSta_flg/1  "VOUTP_DISCButtSta_flg"
  VNMM_AllCANTxReq_flg/1 -> VNMM_AllCANTxReq_flg_Inproc/1  "VNMM_AllCANTxReq_flg"
  VNMM_AllCANTxReq_flg_Inproc/1 -> UnitConverter547/1
  UnitConverter547/1 -> VOUTP_AllCANTxReq_flg/1  "VOUTP_AllCANTxReq_flg"
  VNMM_NMmTxReq_flg/1 -> VNMM_NMmTxReq_flg_Inproc/1  "VNMM_NMmTxReq_flg"
  VNMM_NMmTxReq_flg_Inproc/1 -> UnitConverter548/1
  UnitConverter548/1 -> VOUTP_NMmTxReq_flg/1  "VOUTP_NMmTxReq_flg"
  VNMM_Awake_enum/1 -> VNMM_Awake_enum_Inproc/1  "VNMM_Awake_enum"
  VNMM_Awake_enum_Inproc/1 -> UnitConverter549/1
  UnitConverter549/1 -> VOUTP_Awake_enum/1  "VOUTP_Awake_enum"
  VNMM_CSB_flg/1 -> VNMM_CSB_flg_Inproc/1  "VNMM_CSB_flg"
  VNMM_CSB_flg_Inproc/1 -> UnitConverter550/1
  UnitConverter550/1 -> VOUTP_CSB_flg/1  "VOUTP_CSB_flg"
  VNMM_ErrorState_enum/1 -> VNMM_ErrorState_enum_Inproc/1  "VNMM_ErrorState_enum"
  VNMM_ErrorState_enum_Inproc/1 -> UnitConverter551/1
  UnitConverter551/1 -> VOUTP_ErrorState_enum/1  "VOUTP_ErrorState_enum"
  VNMM_NodeID_enum/1 -> VNMM_NodeID_enum_Inproc/1  "VNMM_NodeID_enum"
  VNMM_NodeID_enum_Inproc/1 -> UnitConverter552/1
  UnitConverter552/1 -> VOUTP_NodeID_enum/1  "VOUTP_NodeID_enum"
  VNMM_PNI_flg/1 -> VNMM_PNI_flg_Inproc/1  "VNMM_PNI_flg"
  VNMM_PNI_flg_Inproc/1 -> UnitConverter553/1
  UnitConverter553/1 -> VOUTP_PNI_flg/1  "VOUTP_PNI_flg"
  VNMM_RptMsgReq_flg/1 -> VNMM_RptMsgReq_flg_Inproc/1  "VNMM_RptMsgReq_flg"
  VNMM_RptMsgReq_flg_Inproc/1 -> UnitConverter554/1
  UnitConverter554/1 -> VOUTP_RptMsgReq_flg/1  "VOUTP_RptMsgReq_flg"
  VNMM_WakeUp_enum/1 -> VNMM_WakeUp_enum_Inproc/1  "VNMM_WakeUp_enum"
  VNMM_WakeUp_enum_Inproc/1 -> UnitConverter555/1
  UnitConverter555/1 -> VOUTP_WakeUp_enum/1  "VOUTP_WakeUp_enum"
  VNMM_ActiveWU_flg/1 -> VNMM_ActiveWU_flg_Inproc/1  "VNMM_ActiveWU_flg"
  VNMM_ActiveWU_flg_Inproc/1 -> UnitConverter556/1
  UnitConverter556/1 -> VOUTP_ActiveWU_flg/1  "VOUTP_ActiveWU_flg"
  VNMM_SysNMmSta_enum/1 -> VNMM_SysNMmSta_enum_Inproc/1  "VNMM_SysNMmSta_enum"
  VNMM_SysNMmSta_enum_Inproc/1 -> UnitConverter557/1
  UnitConverter557/1 -> VOUTP_SysNMmSta_enum/1  "VOUTP_SysNMmSta_enum"
  VNMM_NetworkReq_flg/1 -> VNMM_NetworkReq_flg_Inproc/1  "VNMM_NetworkReq_flg"
  VNMM_NetworkReq_flg_Inproc/1 -> UnitConverter558/1
  UnitConverter558/1 -> VOUTP_NetworkReq_flg/1  "VOUTP_NetworkReq_flg"
  VPMM_PowerUpState_enum/1 -> VPMM_PowerUpState_enum_Inproc/1  "VPMM_PowerUpState_enum"
  VPMM_PowerUpState_enum_Inproc/1 -> UnitConverter559/1
  UnitConverter559/1 -> VOUTP_PowerUpState_enum/1  "VOUTP_PowerUpState_enum"
  VPMM_PowerDownState_enum/1 -> VPMM_PowerDownState_enum_Inproc/1  "VPMM_PowerDownState_enum"
  VPMM_PowerDownState_enum_Inproc/1 -> UnitConverter560/1
  UnitConverter560/1 -> VOUTP_PowerDownState_enum/1  "VOUTP_PowerDownState_enum"
  VPMM_PowerUpFault_enum/1 -> VPMM_PowerUpFault_enum_Inproc/1  "VPMM_PowerUpFault_enum"
  VPMM_PowerUpFault_enum_Inproc/1 -> UnitConverter561/1
  UnitConverter561/1 -> VOUTP_PowerUpFault_enum/1  "VOUTP_PowerUpFault_enum"
  VPMM_PowerDownFault_enum/1 -> VPMM_PowerDownFault_enum_Inproc/1  "VPMM_PowerDownFault_enum"
  VPMM_PowerDownFault_enum_Inproc/1 -> UnitConverter562/1
  UnitConverter562/1 -> VOUTP_PowerDownFault_enum/1  "VOUTP_PowerDownFault_enum"
  VPMM_ActiveDischargeReq_flg/1 -> VPMM_ActiveDischargeReq_flg_Inproc/1  "VPMM_ActiveDischargeReq_flg"
  VPMM_ActiveDischargeReq_flg_Inproc/1 -> UnitConverter563/1
  UnitConverter563/1 -> VOUTP_ActiveDischargeReq_flg/1  "VOUTP_ActiveDischargeReq_flg"
  VPMM_DCDCEnaReq_flg/1 -> VPMM_DCDCEnaReq_flg_Inproc/1  "VPMM_DCDCEnaReq_flg"
  VPMM_DCDCEnaReq_flg_Inproc/1 -> UnitConverter564/1
  UnitConverter564/1 -> VOUTP_DCDCEnaReq_flg/1  "VOUTP_DCDCEnaReq_flg"
  VPMM_DCDCVoltSetpoint_V/1 -> VPMM_DCDCVoltSetpoint_V_Inproc/1  "VPMM_DCDCVoltSetpoint_V"
  VPMM_DCDCVoltSetpoint_V_Inproc/1 -> UnitConverter565/1
  UnitConverter565/1 -> VOUTP_DCDCVoltSetpoint_V/1  "VOUTP_DCDCVoltSetpoint_V"
  VPMM_HVBatCnctReq_flg/1 -> VPMM_HVBatCnctReq_flg_Inproc/1  "VPMM_HVBatCnctReq_flg"
  VPMM_HVBatCnctReq_flg_Inproc/1 -> UnitConverter566/1
  UnitConverter566/1 -> VOUTP_HVBatCnctReq_flg/1  "VOUTP_HVBatCnctReq_flg"
  VPMM_HVSysReadyToCharge_enum/1 -> VPMM_HVSysReadyToCharge_enum_Inproc/1  "VPMM_HVSysReadyToCharge_enum"
  VPMM_HVSysReadyToCharge_enum_Inproc/1 -> UnitConverter567/1
  UnitConverter567/1 -> VOUTP_HVSysReadyToCharge_enum/1  "VOUTP_HVSysReadyToCharge_enum"
  VPMM_PowerSta_enum/1 -> VPMM_PowerSta_enum_Inproc/1  "VPMM_PowerSta_enum"
  VPMM_PowerSta_enum_Inproc/1 -> UnitConverter568/1
  UnitConverter568/1 -> VOUTP_PowerSta_enum/1  "VOUTP_PowerSta_enum"
  VPMM_LVPwrSta_flg/1 -> VPMM_LVPwrSta_flg_Inproc/1  "VPMM_LVPwrSta_flg"
  VPMM_LVPwrSta_flg_Inproc/1 -> UnitConverter569/1
  UnitConverter569/1 -> VOUTP_LVPwrSta_flg/1  "VOUTP_LVPwrSta_flg"
  VPMM_HVPwrSta_flg/1 -> VPMM_HVPwrSta_flg_Inproc/1  "VPMM_HVPwrSta_flg"
  VPMM_HVPwrSta_flg_Inproc/1 -> UnitConverter570/1
  UnitConverter570/1 -> VOUTP_HVPwrSta_flg/1  "VOUTP_HVPwrSta_flg"
  VPMM_SysPowerMode_enum/1 -> VPMM_SysPowerMode_enum_Inproc/1  "VPMM_SysPowerMode_enum"
  VPMM_SysPowerMode_enum_Inproc/1 -> UnitConverter571/1
  UnitConverter571/1 -> VOUTP_SysPowerMode_enum/1  "VOUTP_SysPowerMode_enum"
  VPMM_FrMCUEnaReq_flg/1 -> VPMM_FrMCUEnaReq_flg_Inproc/1  "VPMM_FrMCUEnaReq_flg"
  VPMM_FrMCUEnaReq_flg_Inproc/1 -> UnitConverter572/1
  UnitConverter572/1 -> VOUTP_FrMCUEnaReq_flg/1  "VOUTP_FrMCUEnaReq_flg"
  VPMM_RrMCUEnaReq_flg/1 -> VPMM_RrMCUEnaReq_flg_Inproc/1  "VPMM_RrMCUEnaReq_flg"
  VPMM_RrMCUEnaReq_flg_Inproc/1 -> UnitConverter573/1
  UnitConverter573/1 -> VOUTP_RrMCUEnaReq_flg/1  "VOUTP_RrMCUEnaReq_flg"
  VPMM_DrivetrainSelect_enum/1 -> VPMM_DrivetrainSelect_enum_Inproc/1  "VPMM_DrivetrainSelect_enum"
  VPMM_DrivetrainSelect_enum_Inproc/1 -> UnitConverter574/1
  UnitConverter574/1 -> VOUTP_DrivetrainSelect_enum/1  "VOUTP_DrivetrainSelect_enum"
  VPMM_DrSeatSta_enum/1 -> VPMM_DrSeatSta_enum_Inproc/1  "VPMM_DrSeatSta_enum"
  VPMM_DrSeatSta_enum_Inproc/1 -> UnitConverter575/1
  UnitConverter575/1 -> VOUTP_DrSeatSta_enum/1  "VOUTP_DrSeatSta_enum"
  VPMM_PwrStaSelect_enum/1 -> VPMM_PwrStaSelect_enum_Inproc/1  "VPMM_PwrStaSelect_enum"
  VPMM_PwrStaSelect_enum_Inproc/1 -> UnitConverter576/1
  UnitConverter576/1 -> VOUTP_PwrStaSelect_enum/1  "VOUTP_PwrStaSelect_enum"
  VPMM_PwrStaConstraint_enum/1 -> VPMM_PwrStaConstraint_enum_Inproc/1  "VPMM_PwrStaConstraint_enum"
  VPMM_PwrStaConstraint_enum_Inproc/1 -> UnitConverter577/1
  UnitConverter577/1 -> VOUTP_PwrStaConstraint_enum/1  "VOUTP_PwrStaConstraint_enum"
  VPMM_TCountSta_enum/1 -> VPMM_TCountSta_enum_Inproc/1  "VPMM_TCountSta_enum"
  VPMM_TCountSta_enum_Inproc/1 -> UnitConverter578/1
  UnitConverter578/1 -> VOUTP_TCountSta_enum/1  "VOUTP_TCountSta_enum"
  VPMM_PwrUpReq_enum/1 -> VPMM_PwrUpReq_enum_Inproc/1  "VPMM_PwrUpReq_enum"
  VPMM_PwrUpReq_enum_Inproc/1 -> UnitConverter579/1
  UnitConverter579/1 -> VOUTP_PwrUpReq_enum/1  "VOUTP_PwrUpReq_enum"
  VPMM_PwrDownReq_enum/1 -> VPMM_PwrDownReq_enum_Inproc/1  "VPMM_PwrDownReq_enum"
  VPMM_PwrDownReq_enum_Inproc/1 -> UnitConverter580/1
  UnitConverter580/1 -> VOUTP_PwrDownReq_enum/1  "VOUTP_PwrDownReq_enum"
  VPMM_LowSOCWarn_enum/1 -> VPMM_LowSOCWarn_enum_Inproc/1  "VPMM_LowSOCWarn_enum"
  VPMM_LowSOCWarn_enum_Inproc/1 -> UnitConverter581/1
  UnitConverter581/1 -> VOUTP_LowSOCWarn_enum/1  "VOUTP_LowSOCWarn_enum"
  VPMM_ReVehThdChkSta_enum/1 -> VPMM_ReVehThdChkSta_enum_Inproc/1  "VPMM_ReVehThdChkSta_enum"
  VPMM_ReVehThdChkSta_enum_Inproc/1 -> UnitConverter582/1
  UnitConverter582/1 -> VOUTP_ReVehThdChkSta_enum/1  "VOUTP_ReVehThdChkSta_enum"
  VPMM_EvccAplusPwrUpReq_flg/1 -> VPMM_EvccAplusPwrUpReq_flg_Inproc/1  "VPMM_EvccAplusPwrUpReq_flg"
  VPMM_EvccAplusPwrUpReq_flg_Inproc/1 -> UnitConverter583/1
  UnitConverter583/1 -> VOUTP_EvccAplusPwrUpReq_flg/1  "VOUTP_EvccAplusPwrUpReq_flg"
  VPMM_PwrStaONTOPopReq_flg/1 -> VPMM_PwrStaONTOPopReq_flg_Inproc/1  "VPMM_PwrStaONTOPopReq_flg"
  VPMM_PwrStaONTOPopReq_flg_Inproc/1 -> UnitConverter584/1
  UnitConverter584/1 -> VOUTP_PwrStaONTOPopReq_flg/1  "VOUTP_PwrStaONTOPopReq_flg"
  VPMM_IVIPwrStaONTOPopT_s/1 -> VPMM_IVIPwrStaONTOPopT_s_Inproc/1  "VPMM_IVIPwrStaONTOPopT_s"
  VPMM_IVIPwrStaONTOPopT_s_Inproc/1 -> UnitConverter585/1
  UnitConverter585/1 -> VOUTP_IVIPwrStaONTOPopT_s/1  "VOUTP_IVIPwrStaONTOPopT_s"
  VPMM_LVChrgHoldTtimer_s/1 -> VPMM_LVChrgHoldTtimer_s_Inproc/1  "VPMM_LVChrgHoldTtimer_s"
  VPMM_LVChrgHoldTtimer_s_Inproc/1 -> UnitConverter586/1
  UnitConverter586/1 -> VOUTP_LVChrgHoldTtimer_s/1  "VOUTP_LVChrgHoldTtimer_s"
  VPMM_LVBattChrgTimeCnt_s/1 -> VPMM_LVBattChrgTimeCnt_s_Inproc/1  "VPMM_LVBattChrgTimeCnt_s"
  VPMM_LVBattChrgTimeCnt_s_Inproc/1 -> UnitConverter587/1
  UnitConverter587/1 -> VOUTP_LVBattChrgTimeCnt_s/1  "VOUTP_LVBattChrgTimeCnt_s"
  VPMM_SilentChkAllowSleep_flg/1 -> VPMM_SilentChkAllowSleep_flg_Inproc/1  "VPMM_SilentChkAllowSleep_flg"
  VPMM_SilentChkAllowSleep_flg_Inproc/1 -> UnitConverter588/1
  UnitConverter588/1 -> VOUTP_SilentChkAllowSleep_flg/1  "VOUTP_SilentChkAllowSleep_flg"
  VPMM_TimerAllowSleep_flg/1 -> VPMM_TimerAllowSleep_flg_Inproc/1  "VPMM_TimerAllowSleep_flg"
  VPMM_TimerAllowSleep_flg_Inproc/1 -> UnitConverter589/1
  UnitConverter589/1 -> VOUTP_TimerAllowSleep_flg/1  "VOUTP_TimerAllowSleep_flg"
  VPMM_FDADC12VDetAvg_mV/1 -> VPMM_FDADC12VDetAvg_mV_Inproc/1  "VPMM_FDADC12VDetAvg_mV"
  VPMM_FDADC12VDetAvg_mV_Inproc/1 -> UnitConverter590/1
  UnitConverter590/1 -> VOUTP_FDADC12VDetAvg_mV/1  "VOUTP_FDADC12VDetAvg_mV"
  VPMM_PMMAllowECUSleep_flg/1 -> VPMM_PMMAllowECUSleep_flg_Inproc/1  "VPMM_PMMAllowECUSleep_flg"
  VPMM_PMMAllowECUSleep_flg_Inproc/1 -> UnitConverter591/1
  UnitConverter591/1 -> VOUTP_PMMAllowECUSleep_flg/1  "VOUTP_PMMAllowECUSleep_flg"
  VPMM_LVSilentChrgSta_enum/1 -> VPMM_LVSilentChrgSta_enum_Inproc/1  "VPMM_LVSilentChrgSta_enum"
  VPMM_LVSilentChrgSta_enum_Inproc/1 -> UnitConverter592/1
  UnitConverter592/1 -> VOUTP_LVSilentChrgSta_enum/1  "VOUTP_LVSilentChrgSta_enum"
  VPMM_LVSilentChrgReq_flg/1 -> VPMM_LVSilentChrgReq_flg_Inproc/1  "VPMM_LVSilentChrgReq_flg"
  VPMM_LVSilentChrgReq_flg_Inproc/1 -> UnitConverter593/1
  UnitConverter593/1 -> VOUTP_LVSilentChrgReq_flg/1  "VOUTP_LVSilentChrgReq_flg"
  VPMM_LVSilentChrgLv_enum/1 -> VPMM_LVSilentChrgLv_enum_Inproc/1  "VPMM_LVSilentChrgLv_enum"
  VPMM_LVSilentChrgLv_enum_Inproc/1 -> UnitConverter594/1
  UnitConverter594/1 -> VOUTP_LVSilentChrgLv_enum/1  "VOUTP_LVSilentChrgLv_enum"
  VPMM_CtrlFrPwrStbA1P_flg/1 -> VPMM_CtrlFrPwrStbA1P_flg_Inproc/1  "VPMM_CtrlFrPwrStbA1P_flg"
  VPMM_CtrlFrPwrStbA1P_flg_Inproc/1 -> UnitConverter595/1
  UnitConverter595/1 -> VOUTP_CtrlFrPwrStbA1P_flg/1  "VOUTP_CtrlFrPwrStbA1P_flg"
  VPMM_CtrlFrRC1_flg/1 -> VPMM_CtrlFrRC1_flg_Inproc/1  "VPMM_CtrlFrRC1_flg"
  VPMM_CtrlFrRC1_flg_Inproc/1 -> UnitConverter596/1
  UnitConverter596/1 -> VOUTP_CtrlFrRC1_flg/1  "VOUTP_CtrlFrRC1_flg"
  VPMM_CtrlFrBMSCCUCIR_flg/1 -> VPMM_CtrlFrBMSCCUCIR_flg_Inproc/1  "VPMM_CtrlFrBMSCCUCIR_flg"
  VPMM_CtrlFrBMSCCUCIR_flg_Inproc/1 -> UnitConverter597/1
  UnitConverter597/1 -> VOUTP_CtrlFrBMSCCUCIR_flg/1  "VOUTP_CtrlFrBMSCCUCIR_flg"
  VPMM_CtrlFrEDUINVERTER_flg/1 -> VPMM_CtrlFrEDUINVERTER_flg_Inproc/1  "VPMM_CtrlFrEDUINVERTER_flg"
  VPMM_CtrlFrEDUINVERTER_flg_Inproc/1 -> UnitConverter598/1
  UnitConverter598/1 -> VOUTP_CtrlFrEDUINVERTER_flg/1  "VOUTP_CtrlFrEDUINVERTER_flg"
  VPMM_HWResetSta_enum/1 -> VPMM_HWResetSta_enum_Inproc/1  "VPMM_HWResetSta_enum"
  VPMM_HWResetSta_enum_Inproc/1 -> UnitConverter599/1
  UnitConverter599/1 -> VOUTP_HWResetSta_enum/1  "VOUTP_HWResetSta_enum"
  VPMM_CtrlDrPwrStbA2_flg/1 -> VPMM_CtrlDrPwrStbA2_flg_Inproc/1  "VPMM_CtrlDrPwrStbA2_flg"
  VPMM_CtrlDrPwrStbA2_flg_Inproc/1 -> UnitConverter600/1
  UnitConverter600/1 -> VOUTP_CtrlDrPwrStbA2_flg/1  "VOUTP_CtrlDrPwrStbA2_flg"
  VPMM_PwrStaTOSta_enum/1 -> VPMM_PwrStaTOSta_enum_Inproc/1  "VPMM_PwrStaTOSta_enum"
  VPMM_PwrStaTOSta_enum_Inproc/1 -> UnitConverter601/1
  UnitConverter601/1 -> VOUTP_PwrStaTOSta_enum/1  "VOUTP_PwrStaTOSta_enum"
  VPMM_Sched_ChgTOSta_enum/1 -> VPMM_Sched_ChgTOSta_enum_Inproc/1  "VPMM_Sched_ChgTOSta_enum"
  VPMM_Sched_ChgTOSta_enum_Inproc/1 -> UnitConverter602/1
  UnitConverter602/1 -> VOUTP_Sched_ChgTOSta_enum/1  "VOUTP_Sched_ChgTOSta_enum"
  VPMM_PwrReq_OTA_enum/1 -> VPMM_PwrReq_OTA_enum_Inproc/1  "VPMM_PwrReq_OTA_enum"
  VPMM_PwrReq_OTA_enum_Inproc/1 -> UnitConverter603/1
  UnitConverter603/1 -> VOUTP_PwrReq_OTA_enum/1  "VOUTP_PwrReq_OTA_enum"
  VPMM_OTAPwrReqOFFChkSta_enum/1 -> VPMM_OTAPwrReqOFFChkSta_enum_Inproc/1  "VPMM_OTAPwrReqOFFChkSta_enum"
  VPMM_OTAPwrReqOFFChkSta_enum_Inproc/1 -> UnitConverter604/1
  UnitConverter604/1 -> VOUTP_OTAPwrReqOFFChkSta_enum/1  "VOUTP_OTAPwrReqOFFChkSta_enum"
  VPMM_OTAPwrReqStdChkSta_enum/1 -> VPMM_OTAPwrReqStdChkSta_enum_Inproc/1  "VPMM_OTAPwrReqStdChkSta_enum"
  VPMM_OTAPwrReqStdChkSta_enum_Inproc/1 -> UnitConverter605/1
  UnitConverter605/1 -> VOUTP_OTAPwrReqStdChkSta_enum/1  "VOUTP_OTAPwrReqStdChkSta_enum"
  VPMM_PwrReqRAPSAvail_flg/1 -> VPMM_PwrReqRAPSAvail_flg_Inproc/1  "VPMM_PwrReqRAPSAvail_flg"
  VPMM_PwrReqRAPSAvail_flg_Inproc/1 -> UnitConverter606/1
  UnitConverter606/1 -> VOUTP_PwrReqRAPSAvail_flg/1  "VOUTP_PwrReqRAPSAvail_flg"
  VSYS_HWVer1_cnt/1 -> VSYS_HWVer1_cnt_Inproc/1  "VSYS_HWVer1_cnt"
  VSYS_HWVer1_cnt_Inproc/1 -> UnitConverter607/1
  UnitConverter607/1 -> VOUTP_HWVer1_cnt/1  "VOUTP_HWVer1_cnt"
  VSYS_HWVer2_cnt/1 -> VSYS_HWVer2_cnt_Inproc/1  "VSYS_HWVer2_cnt"
  VSYS_HWVer2_cnt_Inproc/1 -> UnitConverter608/1
  UnitConverter608/1 -> VOUTP_HWVer2_cnt/1  "VOUTP_HWVer2_cnt"
  VSYS_HWVer3_cnt/1 -> VSYS_HWVer3_cnt_Inproc/1  "VSYS_HWVer3_cnt"
  VSYS_HWVer3_cnt_Inproc/1 -> UnitConverter609/1
  UnitConverter609/1 -> VOUTP_HWVer3_cnt/1  "VOUTP_HWVer3_cnt"
  VSYS_CarModel1_cnt/1 -> VSYS_CarModel1_cnt_Inproc/1  "VSYS_CarModel1_cnt"
  VSYS_CarModel1_cnt_Inproc/1 -> UnitConverter610/1
  UnitConverter610/1 -> VOUTP_CarModel1_cnt/1  "VOUTP_CarModel1_cnt"
  VSYS_CarModel2_cnt/1 -> VSYS_CarModel2_cnt_Inproc/1  "VSYS_CarModel2_cnt"
  VSYS_CarModel2_cnt_Inproc/1 -> UnitConverter611/1
  UnitConverter611/1 -> VOUTP_CarModel2_cnt/1  "VOUTP_CarModel2_cnt"
  VSYS_CarModel3_cnt/1 -> VSYS_CarModel3_cnt_Inproc/1  "VSYS_CarModel3_cnt"
  VSYS_CarModel3_cnt_Inproc/1 -> UnitConverter612/1
  UnitConverter612/1 -> VOUTP_CarModel3_cnt/1  "VOUTP_CarModel3_cnt"
  VSYS_ECU1_cnt/1 -> VSYS_ECU1_cnt_Inproc/1  "VSYS_ECU1_cnt"
  VSYS_ECU1_cnt_Inproc/1 -> UnitConverter613/1
  UnitConverter613/1 -> VOUTP_ECU1_cnt/1  "VOUTP_ECU1_cnt"
  VSYS_ECU2_cnt/1 -> VSYS_ECU2_cnt_Inproc/1  "VSYS_ECU2_cnt"
  VSYS_ECU2_cnt_Inproc/1 -> UnitConverter614/1
  UnitConverter614/1 -> VOUTP_ECU2_cnt/1  "VOUTP_ECU2_cnt"
  VSYS_Major1_cnt/1 -> VSYS_Major1_cnt_Inproc/1  "VSYS_Major1_cnt"
  VSYS_Major1_cnt_Inproc/1 -> UnitConverter615/1
  UnitConverter615/1 -> VOUTP_Major1_cnt/1  "VOUTP_Major1_cnt"
  VSYS_Major2_cnt/1 -> VSYS_Major2_cnt_Inproc/1  "VSYS_Major2_cnt"
  VSYS_Major2_cnt_Inproc/1 -> UnitConverter616/1
  UnitConverter616/1 -> VOUTP_Major2_cnt/1  "VOUTP_Major2_cnt"
  VSYS_Minor1_cnt/1 -> VSYS_Minor1_cnt_Inproc/1  "VSYS_Minor1_cnt"
  VSYS_Minor1_cnt_Inproc/1 -> UnitConverter617/1
  UnitConverter617/1 -> VOUTP_Minor1_cnt/1  "VOUTP_Minor1_cnt"
  VSYS_Minor2_cnt/1 -> VSYS_Minor2_cnt_Inproc/1  "VSYS_Minor2_cnt"
  VSYS_Minor2_cnt_Inproc/1 -> UnitConverter618/1
  UnitConverter618/1 -> VOUTP_Minor2_cnt/1  "VOUTP_Minor2_cnt"
  VSYS_Patch1_cnt/1 -> VSYS_Patch1_cnt_Inproc/1  "VSYS_Patch1_cnt"
  VSYS_Patch1_cnt_Inproc/1 -> UnitConverter619/1
  UnitConverter619/1 -> VOUTP_Patch1_cnt/1  "VOUTP_Patch1_cnt"
  VSYS_Patch2_cnt/1 -> VSYS_Patch2_cnt_Inproc/1  "VSYS_Patch2_cnt"
  VSYS_Patch2_cnt_Inproc/1 -> UnitConverter620/1
  UnitConverter620/1 -> VOUTP_Patch2_cnt/1  "VOUTP_Patch2_cnt"
  VSYS_Country1_cnt/1 -> VSYS_Country1_cnt_Inproc/1  "VSYS_Country1_cnt"
  VSYS_Country1_cnt_Inproc/1 -> UnitConverter621/1
  UnitConverter621/1 -> VOUTP_Country1_cnt/1  "VOUTP_Country1_cnt"
  VSYS_Country2_cnt/1 -> VSYS_Country2_cnt_Inproc/1  "VSYS_Country2_cnt"
  VSYS_Country2_cnt_Inproc/1 -> UnitConverter622/1
  UnitConverter622/1 -> VOUTP_Country2_cnt/1  "VOUTP_Country2_cnt"
  VSYS_Variation_cnt/1 -> VSYS_Variation_cnt_Inproc/1  "VSYS_Variation_cnt"
  VSYS_Variation_cnt_Inproc/1 -> UnitConverter623/1
  UnitConverter623/1 -> VOUTP_Variation_cnt/1  "VOUTP_Variation_cnt"
  VSYS_Dash1_cnt/1 -> VSYS_Dash1_cnt_Inproc/1  "VSYS_Dash1_cnt"
  VSYS_Dash1_cnt_Inproc/1 -> UnitConverter624/1
  UnitConverter624/1 -> VOUTP_Dash1_cnt/1  "VOUTP_Dash1_cnt"
  VSYS_Change1_cnt/1 -> VSYS_Change1_cnt_Inproc/1  "VSYS_Change1_cnt"
  VSYS_Change1_cnt_Inproc/1 -> UnitConverter625/1
  UnitConverter625/1 -> VOUTP_Change1_cnt/1  "VOUTP_Change1_cnt"
  VSYS_Change2_cnt/1 -> VSYS_Change2_cnt_Inproc/1  "VSYS_Change2_cnt"
  VSYS_Change2_cnt_Inproc/1 -> UnitConverter626/1
  UnitConverter626/1 -> VOUTP_Change2_cnt/1  "VOUTP_Change2_cnt"
  VSYS_Dash2_cnt/1 -> VSYS_Dash2_cnt_Inproc/1  "VSYS_Dash2_cnt"
  VSYS_Dash2_cnt_Inproc/1 -> UnitConverter627/1
  UnitConverter627/1 -> VOUTP_Dash2_cnt/1  "VOUTP_Dash2_cnt"
  VSYS_SHA1_cnt/1 -> VSYS_SHA1_cnt_Inproc/1  "VSYS_SHA1_cnt"
  VSYS_SHA1_cnt_Inproc/1 -> UnitConverter628/1
  UnitConverter628/1 -> VOUTP_SHA1_cnt/1  "VOUTP_SHA1_cnt"
  VSYS_SHA2_cnt/1 -> VSYS_SHA2_cnt_Inproc/1  "VSYS_SHA2_cnt"
  VSYS_SHA2_cnt_Inproc/1 -> UnitConverter629/1
  UnitConverter629/1 -> VOUTP_SHA2_cnt/1  "VOUTP_SHA2_cnt"
  VSYS_SHA3_cnt/1 -> VSYS_SHA3_cnt_Inproc/1  "VSYS_SHA3_cnt"
  VSYS_SHA3_cnt_Inproc/1 -> UnitConverter630/1
  UnitConverter630/1 -> VOUTP_SHA3_cnt/1  "VOUTP_SHA3_cnt"
  VSYS_SHA4_cnt/1 -> VSYS_SHA4_cnt_Inproc/1  "VSYS_SHA4_cnt"
  VSYS_SHA4_cnt_Inproc/1 -> UnitConverter631/1
  UnitConverter631/1 -> VOUTP_SHA4_cnt/1  "VOUTP_SHA4_cnt"
  VSYS_SHA5_cnt/1 -> VSYS_SHA5_cnt_Inproc/1  "VSYS_SHA5_cnt"
  VSYS_SHA5_cnt_Inproc/1 -> UnitConverter632/1
  UnitConverter632/1 -> VOUTP_SHA5_cnt/1  "VOUTP_SHA5_cnt"
  VSYS_SHA6_cnt/1 -> VSYS_SHA6_cnt_Inproc/1  "VSYS_SHA6_cnt"
  VSYS_SHA6_cnt_Inproc/1 -> UnitConverter633/1
  UnitConverter633/1 -> VOUTP_SHA6_cnt/1  "VOUTP_SHA6_cnt"
  VSYS_SHA7_cnt/1 -> VSYS_SHA7_cnt_Inproc/1  "VSYS_SHA7_cnt"
  VSYS_SHA7_cnt_Inproc/1 -> UnitConverter634/1
  UnitConverter634/1 -> VOUTP_SHA7_cnt/1  "VOUTP_SHA7_cnt"
  VSYS_SHA8_cnt/1 -> VSYS_SHA8_cnt_Inproc/1  "VSYS_SHA8_cnt"
  VSYS_SHA8_cnt_Inproc/1 -> UnitConverter635/1
  UnitConverter635/1 -> VOUTP_SHA8_cnt/1  "VOUTP_SHA8_cnt"
  VSYS_NvWriteReqRisingEdge_flg/1 -> VSYS_NvWriteReqRisingEdge_flg_Inproc/1  "VSYS_NvWriteReqRisingEdge_flg"
  VSYS_NvWriteReqRisingEdge_flg_Inproc/1 -> UnitConverter636/1
  UnitConverter636/1 -> VOUTP_NvWriteReqRisingEdge_flg/1  "VOUTP_NvWriteReqRisingEdge_flg"
  VSYS_FdcSlpReqRisingEdge_flg/1 -> VSYS_FdcSlpReqRisingEdge_flg_Inproc/1  "VSYS_FdcSlpReqRisingEdge_flg"
  VSYS_FdcSlpReqRisingEdge_flg_Inproc/1 -> UnitConverter637/1
  UnitConverter637/1 -> VOUTP_FdcSlpReqRisingEdge_flg/1  "VOUTP_FdcSlpReqRisingEdge_flg"
  VSYS_FdcSlpTime_sec/1 -> VSYS_FdcSlpTime_sec_Inproc/1  "VSYS_FdcSlpTime_sec"
  VSYS_FdcSlpTime_sec_Inproc/1 -> UnitConverter638/1
  UnitConverter638/1 -> VOUTP_FdcSlpTime_sec/1  "VOUTP_FdcSlpTime_sec"
  VSYS_PmicBootReason_enum/1 -> VSYS_PmicBootReason_enum_Inproc/1  "VSYS_PmicBootReason_enum"
  VSYS_PmicBootReason_enum_Inproc/1 -> UnitConverter639/1
  UnitConverter639/1 -> VOUTP_PmicBootReason_enum/1  "VOUTP_PmicBootReason_enum"
  VSYS_WisrBootReason_raw32/1 -> VSYS_WisrBootReason_raw32_Inproc/1  "VSYS_WisrBootReason_raw32"
  VSYS_WisrBootReason_raw32_Inproc/1 -> UnitConverter640/1
  UnitConverter640/1 -> VOUTP_WisrBootReason_raw32/1  "VOUTP_WisrBootReason_raw32"
  VSYS_AcoreRebootCmdACK_flg/1 -> VSYS_AcoreRebootCmdACK_flg_Inproc/1  "VSYS_AcoreRebootCmdACK_flg"
  VSYS_AcoreRebootCmdACK_flg_Inproc/1 -> UnitConverter641/1
  UnitConverter641/1 -> VOUTP_AcoreRebootCmdACK_flg/1  "VOUTP_AcoreRebootCmdACK_flg"
  VSYS_CurrentNmState_enum/1 -> VSYS_CurrentNmState_enum_Inproc/1  "VSYS_CurrentNmState_enum"
  VSYS_CurrentNmState_enum_Inproc/1 -> UnitConverter642/1
  UnitConverter642/1 -> VOUTP_CurrentNmState_enum/1  "VOUTP_CurrentNmState_enum"
  VSYS_ECUGen1_cnt/1 -> VSYS_ECUGen1_cnt_Inproc/1  "VSYS_ECUGen1_cnt"
  VSYS_ECUGen1_cnt_Inproc/1 -> UnitConverter643/1
  UnitConverter643/1 -> VOUTP_ECUGen1_cnt/1  "VOUTP_ECUGen1_cnt"
  VSYS_ECUGen2_cnt/1 -> VSYS_ECUGen2_cnt_Inproc/1  "VSYS_ECUGen2_cnt"
  VSYS_ECUGen2_cnt_Inproc/1 -> UnitConverter644/1
  UnitConverter644/1 -> VOUTP_ECUGen2_cnt/1  "VOUTP_ECUGen2_cnt"
  VSYS_PmicBootPath_raw32/1 -> VSYS_PmicBootPath_raw32_Inproc/1  "VSYS_PmicBootPath_raw32"
  VSYS_PmicBootPath_raw32_Inproc/1 -> UnitConverter645/1
  UnitConverter645/1 -> VOUTP_PmicBootPath_raw32/1  "VOUTP_PmicBootPath_raw32"
  VSYS_DrivingMode_cnt/1 -> VSYS_DrivingMode_cnt_Inproc/1  "VSYS_DrivingMode_cnt"
  VSYS_DrivingMode_cnt_Inproc/1 -> UnitConverter646/1
  UnitConverter646/1 -> VOUTP_DrivingMode_cnt/1  "VOUTP_DrivingMode_cnt"
  VSYS_ModelYear_cnt/1 -> VSYS_ModelYear_cnt_Inproc/1  "VSYS_ModelYear_cnt"
  VSYS_ModelYear_cnt_Inproc/1 -> UnitConverter647/1
  UnitConverter647/1 -> VOUTP_ModelYear_cnt/1  "VOUTP_ModelYear_cnt"
  VSYS_Var4_cnt/1 -> VSYS_Var4_cnt_Inproc/1  "VSYS_Var4_cnt"
  VSYS_Var4_cnt_Inproc/1 -> UnitConverter648/1
  UnitConverter648/1 -> VOUTP_Var4_cnt/1  "VOUTP_Var4_cnt"
  VSYS_Var5_cnt/1 -> VSYS_Var5_cnt_Inproc/1  "VSYS_Var5_cnt"
  VSYS_Var5_cnt_Inproc/1 -> UnitConverter649/1
  UnitConverter649/1 -> VOUTP_Var5_cnt/1  "VOUTP_Var5_cnt"
  VTHC_FDCompCmd_rpm/1 -> VTHC_FDCompCmd_rpm_Inproc/1  "VTHC_FDCompCmd_rpm"
  VTHC_FDCompCmd_rpm_Inproc/1 -> UnitConverter650/1
  UnitConverter650/1 -> VOUTP_FDCompCmd_rpm/1  "VOUTP_FDCompCmd_rpm"
  VTHC_FDSOV1Cmd_flg/1 -> VTHC_FDSOV1Cmd_flg_Inproc/1  "VTHC_FDSOV1Cmd_flg"
  VTHC_FDSOV1Cmd_flg_Inproc/1 -> UnitConverter651/1
  UnitConverter651/1 -> VOUTP_FDSOV1Cmd_flg/1  "VOUTP_FDSOV1Cmd_flg"
  VTHC_FDSOV2Cmd_flg/1 -> VTHC_FDSOV2Cmd_flg_Inproc/1  "VTHC_FDSOV2Cmd_flg"
  VTHC_FDSOV2Cmd_flg_Inproc/1 -> UnitConverter652/1
  UnitConverter652/1 -> VOUTP_FDSOV2Cmd_flg/1  "VOUTP_FDSOV2Cmd_flg"
  VTHC_FDSOV3Cmd_flg/1 -> VTHC_FDSOV3Cmd_flg_Inproc/1  "VTHC_FDSOV3Cmd_flg"
  VTHC_FDSOV3Cmd_flg_Inproc/1 -> UnitConverter653/1
  UnitConverter653/1 -> VOUTP_FDSOV3Cmd_flg/1  "VOUTP_FDSOV3Cmd_flg"
  VTHC_FDEXV1Cmd_step/1 -> VTHC_FDEXV1Cmd_step_Inproc/1  "VTHC_FDEXV1Cmd_step"
  VTHC_FDEXV1Cmd_step_Inproc/1 -> UnitConverter654/1
  UnitConverter654/1 -> VOUTP_FDEXV1Cmd_step/1  "VOUTP_FDEXV1Cmd_step"
  VTHC_FDEXV2Cmd_step/1 -> VTHC_FDEXV2Cmd_step_Inproc/1  "VTHC_FDEXV2Cmd_step"
  VTHC_FDEXV2Cmd_step_Inproc/1 -> UnitConverter655/1
  UnitConverter655/1 -> VOUTP_FDEXV2Cmd_step/1  "VOUTP_FDEXV2Cmd_step"
  VTHC_FDSOTXVCmd_flg/1 -> VTHC_FDSOTXVCmd_flg_Inproc/1  "VTHC_FDSOTXVCmd_flg"
  VTHC_FDSOTXVCmd_flg_Inproc/1 -> UnitConverter656/1
  UnitConverter656/1 -> VOUTP_FDSOTXVCmd_flg/1  "VOUTP_FDSOTXVCmd_flg"
  VTHC_FDFWVCmd_flg/1 -> VTHC_FDFWVCmd_flg_Inproc/1  "VTHC_FDFWVCmd_flg"
  VTHC_FDFWVCmd_flg_Inproc/1 -> UnitConverter657/1
  UnitConverter657/1 -> VOUTP_FDFWVCmd_flg/1  "VOUTP_FDFWVCmd_flg"
  VTHC_FDTWVCmd_pct/1 -> VTHC_FDTWVCmd_pct_Inproc/1  "VTHC_FDTWVCmd_pct"
  VTHC_FDTWVCmd_pct_Inproc/1 -> UnitConverter658/1
  UnitConverter658/1 -> VOUTP_FDTWVCmd_pct/1  "VOUTP_FDTWVCmd_pct"
  VTHC_FDFrWPTCHeatPwrCmd_W/1 -> VTHC_FDFrWPTCHeatPwrCmd_W_Inproc/1  "VTHC_FDFrWPTCHeatPwrCmd_W"
  VTHC_FDFrWPTCHeatPwrCmd_W_Inproc/1 -> UnitConverter659/1
  UnitConverter659/1 -> VOUTP_FDFrWPTCHeatPwrCmd_W/1  "VOUTP_FDFrWPTCHeatPwrCmd_W"
  VTHC_CoolgFanActDuty_pct/1 -> VTHC_CoolgFanActDuty_pct_Inproc/1  "VTHC_CoolgFanActDuty_pct"
  VTHC_CoolgFanActDuty_pct_Inproc/1 -> UnitConverter660/1
  UnitConverter660/1 -> VOUTP_CoolgFanActDuty_pct/1  "VOUTP_CoolgFanActDuty_pct"
  VTHC_FDAGSCmd_enum/1 -> VTHC_FDAGSCmd_enum_Inproc/1  "VTHC_FDAGSCmd_enum"
  VTHC_FDAGSCmd_enum_Inproc/1 -> UnitConverter661/1
  UnitConverter661/1 -> VOUTP_FDAGSCmd_enum/1  "VOUTP_FDAGSCmd_enum"
  VTHC_FDEWP1Cmd_enum/1 -> VTHC_FDEWP1Cmd_enum_Inproc/1  "VTHC_FDEWP1Cmd_enum"
  VTHC_FDEWP1Cmd_enum_Inproc/1 -> UnitConverter662/1
  UnitConverter662/1 -> VOUTP_FDEWP1Cmd_enum/1  "VOUTP_FDEWP1Cmd_enum"
  VTHC_FDEWP2Cmd_enum/1 -> VTHC_FDEWP2Cmd_enum_Inproc/1  "VTHC_FDEWP2Cmd_enum"
  VTHC_FDEWP2Cmd_enum_Inproc/1 -> UnitConverter663/1
  UnitConverter663/1 -> VOUTP_FDEWP2Cmd_enum/1  "VOUTP_FDEWP2Cmd_enum"
  VTHC_FDEWP3Cmd_enum/1 -> VTHC_FDEWP3Cmd_enum_Inproc/1  "VTHC_FDEWP3Cmd_enum"
  VTHC_FDEWP3Cmd_enum_Inproc/1 -> UnitConverter664/1
  UnitConverter664/1 -> VOUTP_FDEWP3Cmd_enum/1  "VOUTP_FDEWP3Cmd_enum"
  VTHC_FDFrLeAPTCHeatPwrCmd_W/1 -> VTHC_FDFrLeAPTCHeatPwrCmd_W_Inproc/1  "VTHC_FDFrLeAPTCHeatPwrCmd_W"
  VTHC_FDFrLeAPTCHeatPwrCmd_W_Inproc/1 -> UnitConverter665/1
  UnitConverter665/1 -> VOUTP_FDFrLeAPTCHeatPwrCmd_W/1  "VOUTP_FDFrLeAPTCHeatPwrCmd_W"
  VTHC_FDFrRiAPTCHeatPwrCmd_W/1 -> VTHC_FDFrRiAPTCHeatPwrCmd_W_Inproc/1  "VTHC_FDFrRiAPTCHeatPwrCmd_W"
  VTHC_FDFrRiAPTCHeatPwrCmd_W_Inproc/1 -> UnitConverter666/1
  UnitConverter666/1 -> VOUTP_FDFrRiAPTCHeatPwrCmd_W/1  "VOUTP_FDFrRiAPTCHeatPwrCmd_W"
  VTHC_FDRrAPTCHeatPwrCmd_W/1 -> VTHC_FDRrAPTCHeatPwrCmd_W_Inproc/1  "VTHC_FDRrAPTCHeatPwrCmd_W"
  VTHC_FDRrAPTCHeatPwrCmd_W_Inproc/1 -> UnitConverter667/1
  UnitConverter667/1 -> VOUTP_FDRrAPTCHeatPwrCmd_W/1  "VOUTP_FDRrAPTCHeatPwrCmd_W"
  VTHC_FDBlowerCmd_pct/1 -> VTHC_FDBlowerCmd_pct_Inproc/1  "VTHC_FDBlowerCmd_pct"
  VTHC_FDBlowerCmd_pct_Inproc/1 -> UnitConverter668/1
  UnitConverter668/1 -> VOUTP_FDBlowerCmd_pct/1  "VOUTP_FDBlowerCmd_pct"
  VTHC_BatteryMode_enum/1 -> VTHC_BatteryMode_enum_Inproc/1  "VTHC_BatteryMode_enum"
  VTHC_BatteryMode_enum_Inproc/1 -> UnitConverter669/1
  UnitConverter669/1 -> VOUTP_BatteryMode_enum/1  "VOUTP_BatteryMode_enum"
  VTHC_EDriveMode_enum/1 -> VTHC_EDriveMode_enum_Inproc/1  "VTHC_EDriveMode_enum"
  VTHC_EDriveMode_enum_Inproc/1 -> UnitConverter670/1
  UnitConverter670/1 -> VOUTP_EDriveMode_enum/1  "VOUTP_EDriveMode_enum"
  VTHC_CabinMode_enum/1 -> VTHC_CabinMode_enum_Inproc/1  "VTHC_CabinMode_enum"
  VTHC_CabinMode_enum_Inproc/1 -> UnitConverter671/1
  UnitConverter671/1 -> VOUTP_CabinMode_enum/1  "VOUTP_CabinMode_enum"
  VTHC_CCUACLampSts_flg/1 -> VTHC_CCUACLampSts_flg_Inproc/1  "VTHC_CCUACLampSts_flg"
  VTHC_CCUACLampSts_flg_Inproc/1 -> UnitConverter672/1
  UnitConverter672/1 -> VOUTP_CCUACLampSts_flg/1  "VOUTP_CCUACLampSts_flg"
  VTHC_CCUAutoLampSts_flg/1 -> VTHC_CCUAutoLampSts_flg_Inproc/1  "VTHC_CCUAutoLampSts_flg"
  VTHC_CCUAutoLampSts_flg_Inproc/1 -> UnitConverter673/1
  UnitConverter673/1 -> VOUTP_CCUAutoLampSts_flg/1  "VOUTP_CCUAutoLampSts_flg"
  VTHC_CCUACMaxLampSts_flg/1 -> VTHC_CCUACMaxLampSts_flg_Inproc/1  "VTHC_CCUACMaxLampSts_flg"
  VTHC_CCUACMaxLampSts_flg_Inproc/1 -> UnitConverter674/1
  UnitConverter674/1 -> VOUTP_CCUACMaxLampSts_flg/1  "VOUTP_CCUACMaxLampSts_flg"
  VTHC_CCUSyncLampSts_flg/1 -> VTHC_CCUSyncLampSts_flg_Inproc/1  "VTHC_CCUSyncLampSts_flg"
  VTHC_CCUSyncLampSts_flg_Inproc/1 -> UnitConverter675/1
  UnitConverter675/1 -> VOUTP_CCUSyncLampSts_flg/1  "VOUTP_CCUSyncLampSts_flg"
  VTHC_sigAirIntenZon1St_enum/1 -> VTHC_sigAirIntenZon1St_enum_Inproc/1  "VTHC_sigAirIntenZon1St_enum"
  VTHC_sigAirIntenZon1St_enum_Inproc/1 -> UnitConverter676/1
  UnitConverter676/1 -> VOUTP_sigAirIntenZon1St_enum/1  "VOUTP_sigAirIntenZon1St_enum"
  VTHC_sigWindDirZon1St_enum/1 -> VTHC_sigWindDirZon1St_enum_Inproc/1  "VTHC_sigWindDirZon1St_enum"
  VTHC_sigWindDirZon1St_enum_Inproc/1 -> UnitConverter677/1
  UnitConverter677/1 -> VOUTP_sigWindDirZon1St_enum/1  "VOUTP_sigWindDirZon1St_enum"
  VTHC_sigRecircSt_flg/1 -> VTHC_sigRecircSt_flg_Inproc/1  "VTHC_sigRecircSt_flg"
  VTHC_sigRecircSt_flg_Inproc/1 -> UnitConverter678/1
  UnitConverter678/1 -> VOUTP_sigRecircSt_flg/1  "VOUTP_sigRecircSt_flg"
  VTHC_sigSetTempZon1St_C/1 -> VTHC_sigSetTempZon1St_C_Inproc/1  "VTHC_sigSetTempZon1St_C"
  VTHC_sigSetTempZon1St_C_Inproc/1 -> UnitConverter679/1
  UnitConverter679/1 -> VOUTP_sigSetTempZon1St_C/1  "VOUTP_sigSetTempZon1St_C"
  VTHC_sigSetTempZon2St_C/1 -> VTHC_sigSetTempZon2St_C_Inproc/1  "VTHC_sigSetTempZon2St_C"
  VTHC_sigSetTempZon2St_C_Inproc/1 -> UnitConverter680/1
  UnitConverter680/1 -> VOUTP_sigSetTempZon2St_C/1  "VOUTP_sigSetTempZon2St_C"
  VTHC_sigClntTHvBattOut_C/1 -> VTHC_sigClntTHvBattOut_C_Inproc/1  "VTHC_sigClntTHvBattOut_C"
  VTHC_sigClntTHvBattOut_C_Inproc/1 -> UnitConverter681/1
  UnitConverter681/1 -> VOUTP_sigClntTHvBattOut_C/1  "VOUTP_sigClntTHvBattOut_C"
  VTHC_sigCbnSolarLeft_W/1 -> VTHC_sigCbnSolarLeft_W_Inproc/1  "VTHC_sigCbnSolarLeft_W"
  VTHC_sigCbnSolarLeft_W_Inproc/1 -> UnitConverter682/1
  UnitConverter682/1 -> VOUTP_sigCbnSolarLeft_W/1  "VOUTP_sigCbnSolarLeft_W"
  VTHC_sigClntTHvBattIn_C/1 -> VTHC_sigClntTHvBattIn_C_Inproc/1  "VTHC_sigClntTHvBattIn_C"
  VTHC_sigClntTHvBattIn_C_Inproc/1 -> UnitConverter683/1
  UnitConverter683/1 -> VOUTP_sigClntTHvBattIn_C/1  "VOUTP_sigClntTHvBattIn_C"
  VTHC_sigCbnSolarRight_W/1 -> VTHC_sigCbnSolarRight_W_Inproc/1  "VTHC_sigCbnSolarRight_W"
  VTHC_sigCbnSolarRight_W_Inproc/1 -> UnitConverter684/1
  UnitConverter684/1 -> VOUTP_sigCbnSolarRight_W/1  "VOUTP_sigCbnSolarRight_W"
  VTHC_sigAmbAirT_C/1 -> VTHC_sigAmbAirT_C_Inproc/1  "VTHC_sigAmbAirT_C"
  VTHC_sigAmbAirT_C_Inproc/1 -> UnitConverter685/1
  UnitConverter685/1 -> VOUTP_sigAmbAirT_C/1  "VOUTP_sigAmbAirT_C"
  VTHC_sigCbnAirT_C/1 -> VTHC_sigCbnAirT_C_Inproc/1  "VTHC_sigCbnAirT_C"
  VTHC_sigCbnAirT_C_Inproc/1 -> UnitConverter686/1
  UnitConverter686/1 -> VOUTP_sigCbnAirT_C/1  "VOUTP_sigCbnAirT_C"
  VTHC_ACSubMode_enum/1 -> VTHC_ACSubMode_enum_Inproc/1  "VTHC_ACSubMode_enum"
  VTHC_ACSubMode_enum_Inproc/1 -> UnitConverter687/1
  UnitConverter687/1 -> VOUTP_ACSubMode_enum/1  "VOUTP_ACSubMode_enum"
  VTHC_FDRecyAutoCmd_enum/1 -> VTHC_FDRecyAutoCmd_enum_Inproc/1  "VTHC_FDRecyAutoCmd_enum"
  VTHC_FDRecyAutoCmd_enum_Inproc/1 -> UnitConverter688/1
  UnitConverter688/1 -> VOUTP_FDRecyAutoCmd_enum/1  "VOUTP_FDRecyAutoCmd_enum"
  VTHC_ACModeMem_enum/1 -> VTHC_ACModeMem_enum_Inproc/1  "VTHC_ACModeMem_enum"
  VTHC_ACModeMem_enum_Inproc/1 -> UnitConverter689/1
  UnitConverter689/1 -> VOUTP_ACModeMem_enum/1  "VOUTP_ACModeMem_enum"
  VTHC_Face_flg/1 -> VTHC_Face_flg_Inproc/1  "VTHC_Face_flg"
  VTHC_Face_flg_Inproc/1 -> UnitConverter690/1
  UnitConverter690/1 -> VOUTP_Face_flg/1  "VOUTP_Face_flg"
  VTHC_Foot_flg/1 -> VTHC_Foot_flg_Inproc/1  "VTHC_Foot_flg"
  VTHC_Foot_flg_Inproc/1 -> UnitConverter691/1
  UnitConverter691/1 -> VOUTP_Foot_flg/1  "VOUTP_Foot_flg"
  VTHC_Frost_flg/1 -> VTHC_Frost_flg_Inproc/1  "VTHC_Frost_flg"
  VTHC_Frost_flg_Inproc/1 -> UnitConverter692/1
  UnitConverter692/1 -> VOUTP_Frost_flg/1  "VOUTP_Frost_flg"
  VTHC_FaceM_flg/1 -> VTHC_FaceM_flg_Inproc/1  "VTHC_FaceM_flg"
  VTHC_FaceM_flg_Inproc/1 -> UnitConverter693/1
  UnitConverter693/1 -> VOUTP_FaceM_flg/1  "VOUTP_FaceM_flg"
  VTHC_FootM_flg/1 -> VTHC_FootM_flg_Inproc/1  "VTHC_FootM_flg"
  VTHC_FootM_flg_Inproc/1 -> UnitConverter694/1
  UnitConverter694/1 -> VOUTP_FootM_flg/1  "VOUTP_FootM_flg"
  VTHC_CCUSyncSts_flg/1 -> VTHC_CCUSyncSts_flg_Inproc/1  "VTHC_CCUSyncSts_flg"
  VTHC_CCUSyncSts_flg_Inproc/1 -> UnitConverter695/1
  UnitConverter695/1 -> VOUTP_CCUSyncSts_flg/1  "VOUTP_CCUSyncSts_flg"
  VTHC_RecAutoFlg_flg/1 -> VTHC_RecAutoFlg_flg_Inproc/1  "VTHC_RecAutoFlg_flg"
  VTHC_RecAutoFlg_flg_Inproc/1 -> UnitConverter696/1
  UnitConverter696/1 -> VOUTP_RecAutoFlg_flg/1  "VOUTP_RecAutoFlg_flg"
  VTHC_AirIntenZone1M_enum/1 -> VTHC_AirIntenZone1M_enum_Inproc/1  "VTHC_AirIntenZone1M_enum"
  VTHC_AirIntenZone1M_enum_Inproc/1 -> UnitConverter697/1
  UnitConverter697/1 -> VOUTP_AirIntenZone1M_enum/1  "VOUTP_AirIntenZone1M_enum"
  VTHC_fdefog_flg/1 -> VTHC_fdefog_flg_Inproc/1  "VTHC_fdefog_flg"
  VTHC_fdefog_flg_Inproc/1 -> UnitConverter698/1
  UnitConverter698/1 -> VOUTP_fdefog_flg/1  "VOUTP_fdefog_flg"
  VTHC_sigSetTempZon2StM_C/1 -> VTHC_sigSetTempZon2StM_C_Inproc/1  "VTHC_sigSetTempZon2StM_C"
  VTHC_sigSetTempZon2StM_C_Inproc/1 -> UnitConverter699/1
  UnitConverter699/1 -> VOUTP_sigSetTempZon2StM_C/1  "VOUTP_sigSetTempZon2StM_C"
  VTHC_sigDfrstSt_flg/1 -> VTHC_sigDfrstSt_flg_Inproc/1  "VTHC_sigDfrstSt_flg"
  VTHC_sigDfrstSt_flg_Inproc/1 -> UnitConverter700/1
  UnitConverter700/1 -> VOUTP_sigDfrstSt_flg/1  "VOUTP_sigDfrstSt_flg"
  VTHC_FDCTHCAirIntZ3Sta_enum/1 -> VTHC_FDCTHCAirIntZ3Sta_enum_Inproc/1  "VTHC_FDCTHCAirIntZ3Sta_enum"
  VTHC_FDCTHCAirIntZ3Sta_enum_Inproc/1 -> UnitConverter701/1
  UnitConverter701/1 -> VOUTP_FDCTHCAirIntZ3Sta_enum/1  "VOUTP_FDCTHCAirIntZ3Sta_enum"
  VTHC_FDCTHCLEVentModeSta_enum/1 -> VTHC_FDCTHCLEVentModeSta_enum_Inproc/1  "VTHC_FDCTHCLEVentModeSta_enum"
  VTHC_FDCTHCLEVentModeSta_enum_Inproc/1 -> UnitConverter702/1
  UnitConverter702/1 -> VOUTP_FDCTHCLEVentModeSta_enum/1  "VOUTP_FDCTHCLEVentModeSta_enum"
  VTHC_FDCTHCREVentModeSta_enum/1 -> VTHC_FDCTHCREVentModeSta_enum_Inproc/1  "VTHC_FDCTHCREVentModeSta_enum"
  VTHC_FDCTHCREVentModeSta_enum_Inproc/1 -> UnitConverter703/1
  UnitConverter703/1 -> VOUTP_FDCTHCREVentModeSta_enum/1  "VOUTP_FDCTHCREVentModeSta_enum"
  VTHC_FDCTHCLEVentZSta_enum/1 -> VTHC_FDCTHCLEVentZSta_enum_Inproc/1  "VTHC_FDCTHCLEVentZSta_enum"
  VTHC_FDCTHCLEVentZSta_enum_Inproc/1 -> UnitConverter704/1
  UnitConverter704/1 -> VOUTP_FDCTHCLEVentZSta_enum/1  "VOUTP_FDCTHCLEVentZSta_enum"
  VTHC_FDCTHCCLEVentZSta_enum/1 -> VTHC_FDCTHCCLEVentZSta_enum_Inproc/1  "VTHC_FDCTHCCLEVentZSta_enum"
  VTHC_FDCTHCCLEVentZSta_enum_Inproc/1 -> UnitConverter705/1
  UnitConverter705/1 -> VOUTP_FDCTHCCLEVentZSta_enum/1  "VOUTP_FDCTHCCLEVentZSta_enum"
  VTHC_FDCTHCREVentZSta_enum/1 -> VTHC_FDCTHCREVentZSta_enum_Inproc/1  "VTHC_FDCTHCREVentZSta_enum"
  VTHC_FDCTHCREVentZSta_enum_Inproc/1 -> UnitConverter706/1
  UnitConverter706/1 -> VOUTP_FDCTHCREVentZSta_enum/1  "VOUTP_FDCTHCREVentZSta_enum"
  VTHC_FDCTHCCREVentZSta_enum/1 -> VTHC_FDCTHCCREVentZSta_enum_Inproc/1  "VTHC_FDCTHCCREVentZSta_enum"
  VTHC_FDCTHCCREVentZSta_enum_Inproc/1 -> UnitConverter707/1
  UnitConverter707/1 -> VOUTP_FDCTHCCREVentZSta_enum/1  "VOUTP_FDCTHCCREVentZSta_enum"
  VTHC_FDCTHCLEVentYSta_enum/1 -> VTHC_FDCTHCLEVentYSta_enum_Inproc/1  "VTHC_FDCTHCLEVentYSta_enum"
  VTHC_FDCTHCLEVentYSta_enum_Inproc/1 -> UnitConverter708/1
  UnitConverter708/1 -> VOUTP_FDCTHCLEVentYSta_enum/1  "VOUTP_FDCTHCLEVentYSta_enum"
  VTHC_FDCTHCLVentENSta_flg/1 -> VTHC_FDCTHCLVentENSta_flg_Inproc/1  "VTHC_FDCTHCLVentENSta_flg"
  VTHC_FDCTHCLVentENSta_flg_Inproc/1 -> UnitConverter709/1
  UnitConverter709/1 -> VOUTP_FDCTHCLVentENSta_flg/1  "VOUTP_FDCTHCLVentENSta_flg"
  VTHC_FDCTHCCLEVentYSta_enum/1 -> VTHC_FDCTHCCLEVentYSta_enum_Inproc/1  "VTHC_FDCTHCCLEVentYSta_enum"
  VTHC_FDCTHCCLEVentYSta_enum_Inproc/1 -> UnitConverter710/1
  UnitConverter710/1 -> VOUTP_FDCTHCCLEVentYSta_enum/1  "VOUTP_FDCTHCCLEVentYSta_enum"
  VTHC_FDCTHCCLVentENSta_flg/1 -> VTHC_FDCTHCCLVentENSta_flg_Inproc/1  "VTHC_FDCTHCCLVentENSta_flg"
  VTHC_FDCTHCCLVentENSta_flg_Inproc/1 -> UnitConverter711/1
  UnitConverter711/1 -> VOUTP_FDCTHCCLVentENSta_flg/1  "VOUTP_FDCTHCCLVentENSta_flg"
  VTHC_FDCTHCREVentYSta_enum/1 -> VTHC_FDCTHCREVentYSta_enum_Inproc/1  "VTHC_FDCTHCREVentYSta_enum"
  VTHC_FDCTHCREVentYSta_enum_Inproc/1 -> UnitConverter712/1
  UnitConverter712/1 -> VOUTP_FDCTHCREVentYSta_enum/1  "VOUTP_FDCTHCREVentYSta_enum"
  VTHC_FDCTHCRVentENSta_flg/1 -> VTHC_FDCTHCRVentENSta_flg_Inproc/1  "VTHC_FDCTHCRVentENSta_flg"
  VTHC_FDCTHCRVentENSta_flg_Inproc/1 -> UnitConverter713/1
  UnitConverter713/1 -> VOUTP_FDCTHCRVentENSta_flg/1  "VOUTP_FDCTHCRVentENSta_flg"
  VTHC_FDCTHCCREVentYSta_enum/1 -> VTHC_FDCTHCCREVentYSta_enum_Inproc/1  "VTHC_FDCTHCCREVentYSta_enum"
  VTHC_FDCTHCCREVentYSta_enum_Inproc/1 -> UnitConverter714/1
  UnitConverter714/1 -> VOUTP_FDCTHCCREVentYSta_enum/1  "VOUTP_FDCTHCCREVentYSta_enum"
  VTHC_FDCTHCCRVentENSta_flg/1 -> VTHC_FDCTHCCRVentENSta_flg_Inproc/1  "VTHC_FDCTHCCRVentENSta_flg"
  VTHC_FDCTHCCRVentENSta_flg_Inproc/1 -> UnitConverter715/1
  UnitConverter715/1 -> VOUTP_FDCTHCCRVentENSta_flg/1  "VOUTP_FDCTHCCRVentENSta_flg"
  VTHC_FDCTHCMAPTCForceOFFSta_flg/1 -> VTHC_FDCTHCMAPTCForceOFFSta_flg_Inproc/1  "VTHC_FDCTHCMAPTCForceOFFSta_flg"
  VTHC_FDCTHCMAPTCForceOFFSta_flg_Inproc/1 -> UnitConverter716/1
  UnitConverter716/1 -> VOUTP_FDCTHCMAPTCForceOFFSta_flg/1  "VOUTP_FDCTHCMAPTCForceOFFSta_flg"
  VTHC_FDCFGSAirIntSta_enum/1 -> VTHC_FDCFGSAirIntSta_enum_Inproc/1  "VTHC_FDCFGSAirIntSta_enum"
  VTHC_FDCFGSAirIntSta_enum_Inproc/1 -> UnitConverter717/1
  UnitConverter717/1 -> VOUTP_FDCFGSAirIntSta_enum/1  "VOUTP_FDCFGSAirIntSta_enum"
  VTHC_FDCFGSChSta_enum/1 -> VTHC_FDCFGSChSta_enum_Inproc/1  "VTHC_FDCFGSChSta_enum"
  VTHC_FDCFGSChSta_enum_Inproc/1 -> UnitConverter718/1
  UnitConverter718/1 -> VOUTP_FDCFGSChSta_enum/1  "VOUTP_FDCFGSChSta_enum"
  VTHC_FDCFGSAirIntCmd_enum/1 -> VTHC_FDCFGSAirIntCmd_enum_Inproc/1  "VTHC_FDCFGSAirIntCmd_enum"
  VTHC_FDCFGSAirIntCmd_enum_Inproc/1 -> UnitConverter719/1
  UnitConverter719/1 -> VOUTP_FDCFGSAirIntCmd_enum/1  "VOUTP_FDCFGSAirIntCmd_enum"
  VTHC_FDCFGSFuncSta_enum/1 -> VTHC_FDCFGSFuncSta_enum_Inproc/1  "VTHC_FDCFGSFuncSta_enum"
  VTHC_FDCFGSFuncSta_enum_Inproc/1 -> UnitConverter720/1
  UnitConverter720/1 -> VOUTP_FDCFGSFuncSta_enum/1  "VOUTP_FDCFGSFuncSta_enum"
  VTHC_FDCFGSChCmd_enum/1 -> VTHC_FDCFGSChCmd_enum_Inproc/1  "VTHC_FDCFGSChCmd_enum"
  VTHC_FDCFGSChCmd_enum_Inproc/1 -> UnitConverter721/1
  UnitConverter721/1 -> VOUTP_FDCFGSChCmd_enum/1  "VOUTP_FDCFGSChCmd_enum"
  VTHC_FDCFGSIONSWSta_flg/1 -> VTHC_FDCFGSIONSWSta_flg_Inproc/1  "VTHC_FDCFGSIONSWSta_flg"
  VTHC_FDCFGSIONSWSta_flg_Inproc/1 -> UnitConverter722/1
  UnitConverter722/1 -> VOUTP_FDCFGSIONSWSta_flg/1  "VOUTP_FDCFGSIONSWSta_flg"
  VTHC_FDCFGSIONCmd_flg/1 -> VTHC_FDCFGSIONCmd_flg_Inproc/1  "VTHC_FDCFGSIONCmd_flg"
  VTHC_FDCFGSIONCmd_flg_Inproc/1 -> UnitConverter723/1
  UnitConverter723/1 -> VOUTP_FDCFGSIONCmd_flg/1  "VOUTP_FDCFGSIONCmd_flg"
  VTHC_FDCTHCMPreWPTCHeatSta_enum/1 -> VTHC_FDCTHCMPreWPTCHeatSta_enum_Inproc/1  "VTHC_FDCTHCMPreWPTCHeatSta_enum"
  VTHC_FDCTHCMPreWPTCHeatSta_enum_Inproc/1 -> UnitConverter724/1
  UnitConverter724/1 -> VOUTP_FDCTHCMPreWPTCHeatSta_enum/1  "VOUTP_FDCTHCMPreWPTCHeatSta_enum"
  VTHC_EWPBUflag1_flg/1 -> VTHC_EWPBUflag1_flg_Inproc/1  "VTHC_EWPBUflag1_flg"
  VTHC_EWPBUflag1_flg_Inproc/1 -> UnitConverter725/1
  UnitConverter725/1 -> VOUTP_EWPBUflag1_flg/1  "VOUTP_EWPBUflag1_flg"
  VTHC_EWPBUflag2_flg/1 -> VTHC_EWPBUflag2_flg_Inproc/1  "VTHC_EWPBUflag2_flg"
  VTHC_EWPBUflag2_flg_Inproc/1 -> UnitConverter726/1
  UnitConverter726/1 -> VOUTP_EWPBUflag2_flg/1  "VOUTP_EWPBUflag2_flg"
  VTHC_EWPBUflag3_flg/1 -> VTHC_EWPBUflag3_flg_Inproc/1  "VTHC_EWPBUflag3_flg"
  VTHC_EWPBUflag3_flg_Inproc/1 -> UnitConverter727/1
  UnitConverter727/1 -> VOUTP_EWPBUflag3_flg/1  "VOUTP_EWPBUflag3_flg"
  VTHC_FaceMSet_enum/1 -> VTHC_FaceMSet_enum_Inproc/1  "VTHC_FaceMSet_enum"
  VTHC_FaceMSet_enum_Inproc/1 -> UnitConverter728/1
  UnitConverter728/1 -> VOUTP_FaceMSet_enum/1  "VOUTP_FaceMSet_enum"
  VTHC_FootMSet_enum/1 -> VTHC_FootMSet_enum_Inproc/1  "VTHC_FootMSet_enum"
  VTHC_FootMSet_enum_Inproc/1 -> UnitConverter729/1
  UnitConverter729/1 -> VOUTP_FootMSet_enum/1  "VOUTP_FootMSet_enum"
  VTHC_fdefogSet_enum/1 -> VTHC_fdefogSet_enum_Inproc/1  "VTHC_fdefogSet_enum"
  VTHC_fdefogSet_enum_Inproc/1 -> UnitConverter730/1
  UnitConverter730/1 -> VOUTP_fdefogSet_enum/1  "VOUTP_fdefogSet_enum"
  VTHC_CCUSyncStsSet_enum/1 -> VTHC_CCUSyncStsSet_enum_Inproc/1  "VTHC_CCUSyncStsSet_enum"
  VTHC_CCUSyncStsSet_enum_Inproc/1 -> UnitConverter731/1
  UnitConverter731/1 -> VOUTP_CCUSyncStsSet_enum/1  "VOUTP_CCUSyncStsSet_enum"
  VTHC_sigRecircStSet_enum/1 -> VTHC_sigRecircStSet_enum_Inproc/1  "VTHC_sigRecircStSet_enum"
  VTHC_sigRecircStSet_enum_Inproc/1 -> UnitConverter732/1
  UnitConverter732/1 -> VOUTP_sigRecircStSet_enum/1  "VOUTP_sigRecircStSet_enum"
  VTHC_RecyAutoSet_enum/1 -> VTHC_RecyAutoSet_enum_Inproc/1  "VTHC_RecyAutoSet_enum"
  VTHC_RecyAutoSet_enum_Inproc/1 -> UnitConverter733/1
  UnitConverter733/1 -> VOUTP_RecyAutoSet_enum/1  "VOUTP_RecyAutoSet_enum"
  VTHC_AirIntenZone1MSet1_enum/1 -> VTHC_AirIntenZone1MSet1_enum_Inproc/1  "VTHC_AirIntenZone1MSet1_enum"
  VTHC_AirIntenZone1MSet1_enum_Inproc/1 -> UnitConverter734/1
  UnitConverter734/1 -> VOUTP_AirIntenZone1MSet1_enum/1  "VOUTP_AirIntenZone1MSet1_enum"
  VTHC_AirIntenZone1MSet2_enum/1 -> VTHC_AirIntenZone1MSet2_enum_Inproc/1  "VTHC_AirIntenZone1MSet2_enum"
  VTHC_AirIntenZone1MSet2_enum_Inproc/1 -> UnitConverter735/1
  UnitConverter735/1 -> VOUTP_AirIntenZone1MSet2_enum/1  "VOUTP_AirIntenZone1MSet2_enum"
  VTHC_AirIntenZone1MSet3_enum/1 -> VTHC_AirIntenZone1MSet3_enum_Inproc/1  "VTHC_AirIntenZone1MSet3_enum"
  VTHC_AirIntenZone1MSet3_enum_Inproc/1 -> UnitConverter736/1
  UnitConverter736/1 -> VOUTP_AirIntenZone1MSet3_enum/1  "VOUTP_AirIntenZone1MSet3_enum"
  VTHC_AirIntenZone1MSet4_enum/1 -> VTHC_AirIntenZone1MSet4_enum_Inproc/1  "VTHC_AirIntenZone1MSet4_enum"
  VTHC_AirIntenZone1MSet4_enum_Inproc/1 -> UnitConverter737/1
  UnitConverter737/1 -> VOUTP_AirIntenZone1MSet4_enum/1  "VOUTP_AirIntenZone1MSet4_enum"
  VTHC_AirIntenZone1MSet5_enum/1 -> VTHC_AirIntenZone1MSet5_enum_Inproc/1  "VTHC_AirIntenZone1MSet5_enum"
  VTHC_AirIntenZone1MSet5_enum_Inproc/1 -> UnitConverter738/1
  UnitConverter738/1 -> VOUTP_AirIntenZone1MSet5_enum/1  "VOUTP_AirIntenZone1MSet5_enum"
  VTHC_AirIntenZone1MSet7_enum/1 -> VTHC_AirIntenZone1MSet7_enum_Inproc/1  "VTHC_AirIntenZone1MSet7_enum"
  VTHC_AirIntenZone1MSet7_enum_Inproc/1 -> UnitConverter739/1
  UnitConverter739/1 -> VOUTP_AirIntenZone1MSet7_enum/1  "VOUTP_AirIntenZone1MSet7_enum"
  VTHC_AirIntenZone3MSet1_enum/1 -> VTHC_AirIntenZone3MSet1_enum_Inproc/1  "VTHC_AirIntenZone3MSet1_enum"
  VTHC_AirIntenZone3MSet1_enum_Inproc/1 -> UnitConverter740/1
  UnitConverter740/1 -> VOUTP_AirIntenZone3MSet1_enum/1  "VOUTP_AirIntenZone3MSet1_enum"
  VTHC_AirIntenZone3MSet2_enum/1 -> VTHC_AirIntenZone3MSet2_enum_Inproc/1  "VTHC_AirIntenZone3MSet2_enum"
  VTHC_AirIntenZone3MSet2_enum_Inproc/1 -> UnitConverter741/1
  UnitConverter741/1 -> VOUTP_AirIntenZone3MSet2_enum/1  "VOUTP_AirIntenZone3MSet2_enum"
  VTHC_AirIntenZone3MSet3_enum/1 -> VTHC_AirIntenZone3MSet3_enum_Inproc/1  "VTHC_AirIntenZone3MSet3_enum"
  VTHC_AirIntenZone3MSet3_enum_Inproc/1 -> UnitConverter742/1
  UnitConverter742/1 -> VOUTP_AirIntenZone3MSet3_enum/1  "VOUTP_AirIntenZone3MSet3_enum"
  VTHC_AirIntenZone3MSet4_enum/1 -> VTHC_AirIntenZone3MSet4_enum_Inproc/1  "VTHC_AirIntenZone3MSet4_enum"
  VTHC_AirIntenZone3MSet4_enum_Inproc/1 -> UnitConverter743/1
  UnitConverter743/1 -> VOUTP_AirIntenZone3MSet4_enum/1  "VOUTP_AirIntenZone3MSet4_enum"
  VTHC_AirIntenZone3MSet5_enum/1 -> VTHC_AirIntenZone3MSet5_enum_Inproc/1  "VTHC_AirIntenZone3MSet5_enum"
  VTHC_AirIntenZone3MSet5_enum_Inproc/1 -> UnitConverter744/1
  UnitConverter744/1 -> VOUTP_AirIntenZone3MSet5_enum/1  "VOUTP_AirIntenZone3MSet5_enum"
  VTHC_AirIntenZone3MSet7_enum/1 -> VTHC_AirIntenZone3MSet7_enum_Inproc/1  "VTHC_AirIntenZone3MSet7_enum"
  VTHC_AirIntenZone3MSet7_enum_Inproc/1 -> UnitConverter745/1
  UnitConverter745/1 -> VOUTP_AirIntenZone3MSet7_enum/1  "VOUTP_AirIntenZone3MSet7_enum"
  VTHC_IONSWStaSet_enum/1 -> VTHC_IONSWStaSet_enum_Inproc/1  "VTHC_IONSWStaSet_enum"
  VTHC_IONSWStaSet_enum_Inproc/1 -> UnitConverter746/1
  UnitConverter746/1 -> VOUTP_IONSWStaSet_enum/1  "VOUTP_IONSWStaSet_enum"
  VTHC_FDCFGSChStaSet123_enum/1 -> VTHC_FDCFGSChStaSet123_enum_Inproc/1  "VTHC_FDCFGSChStaSet123_enum"
  VTHC_FDCFGSChStaSet123_enum_Inproc/1 -> UnitConverter747/1
  UnitConverter747/1 -> VOUTP_FDCFGSChStaSet123_enum/1  "VOUTP_FDCFGSChStaSet123_enum"
  VTHC_FDCFGSChStaSet457_enum/1 -> VTHC_FDCFGSChStaSet457_enum_Inproc/1  "VTHC_FDCFGSChStaSet457_enum"
  VTHC_FDCFGSChStaSet457_enum_Inproc/1 -> UnitConverter748/1
  UnitConverter748/1 -> VOUTP_FDCFGSChStaSet457_enum/1  "VOUTP_FDCFGSChStaSet457_enum"
  VTHC_FDCFGSAirIntStaSet123_enum/1 -> VTHC_FDCFGSAirIntStaSet123_enum_Inproc/1  "VTHC_FDCFGSAirIntStaSet123_enum"
  VTHC_FDCFGSAirIntStaSet123_enum_Inproc/1 -> UnitConverter749/1
  UnitConverter749/1 -> VOUTP_FDCFGSAirIntStaSet123_enum/1  "VOUTP_FDCFGSAirIntStaSet123_enum"
  VTHC_FDCFGSAirIntStaSet457_enum/1 -> VTHC_FDCFGSAirIntStaSet457_enum_Inproc/1  "VTHC_FDCFGSAirIntStaSet457_enum"
  VTHC_FDCFGSAirIntStaSet457_enum_Inproc/1 -> UnitConverter750/1
  UnitConverter750/1 -> VOUTP_FDCFGSAirIntStaSet457_enum/1  "VOUTP_FDCFGSAirIntStaSet457_enum"
  VTHC_LVentENSet_enum/1 -> VTHC_LVentENSet_enum_Inproc/1  "VTHC_LVentENSet_enum"
  VTHC_LVentENSet_enum_Inproc/1 -> UnitConverter751/1
  UnitConverter751/1 -> VOUTP_LVentENSet_enum/1  "VOUTP_LVentENSet_enum"
  VTHC_CLVentENSet_enum/1 -> VTHC_CLVentENSet_enum_Inproc/1  "VTHC_CLVentENSet_enum"
  VTHC_CLVentENSet_enum_Inproc/1 -> UnitConverter752/1
  UnitConverter752/1 -> VOUTP_CLVentENSet_enum/1  "VOUTP_CLVentENSet_enum"
  VTHC_RVentENSet_enum/1 -> VTHC_RVentENSet_enum_Inproc/1  "VTHC_RVentENSet_enum"
  VTHC_RVentENSet_enum_Inproc/1 -> UnitConverter753/1
  UnitConverter753/1 -> VOUTP_RVentENSet_enum/1  "VOUTP_RVentENSet_enum"
  VTHC_CRVentENSet_enum/1 -> VTHC_CRVentENSet_enum_Inproc/1  "VTHC_CRVentENSet_enum"
  VTHC_CRVentENSet_enum_Inproc/1 -> UnitConverter754/1
  UnitConverter754/1 -> VOUTP_CRVentENSet_enum/1  "VOUTP_CRVentENSet_enum"
  VTHC_LEVentModeStaSet123_enum/1 -> VTHC_LEVentModeStaSet123_enum_Inproc/1  "VTHC_LEVentModeStaSet123_enum"
  VTHC_LEVentModeStaSet123_enum_Inproc/1 -> UnitConverter755/1
  UnitConverter755/1 -> VOUTP_LEVentModeStaSet123_enum/1  "VOUTP_LEVentModeStaSet123_enum"
  VTHC_LEVentModeStaSet457_enum/1 -> VTHC_LEVentModeStaSet457_enum_Inproc/1  "VTHC_LEVentModeStaSet457_enum"
  VTHC_LEVentModeStaSet457_enum_Inproc/1 -> UnitConverter756/1
  UnitConverter756/1 -> VOUTP_LEVentModeStaSet457_enum/1  "VOUTP_LEVentModeStaSet457_enum"
  VTHC_REVentModeStaSet123_enum/1 -> VTHC_REVentModeStaSet123_enum_Inproc/1  "VTHC_REVentModeStaSet123_enum"
  VTHC_REVentModeStaSet123_enum_Inproc/1 -> UnitConverter757/1
  UnitConverter757/1 -> VOUTP_REVentModeStaSet123_enum/1  "VOUTP_REVentModeStaSet123_enum"
  VTHC_REVentModeStaSet457_enum/1 -> VTHC_REVentModeStaSet457_enum_Inproc/1  "VTHC_REVentModeStaSet457_enum"
  VTHC_REVentModeStaSet457_enum_Inproc/1 -> UnitConverter758/1
  UnitConverter758/1 -> VOUTP_REVentModeStaSet457_enum/1  "VOUTP_REVentModeStaSet457_enum"
  VTHC_FDCTHCLEVentZStaSet1_enum/1 -> VTHC_FDCTHCLEVentZStaSet1_enum_Inproc/1  "VTHC_FDCTHCLEVentZStaSet1_enum"
  VTHC_FDCTHCLEVentZStaSet1_enum_Inproc/1 -> UnitConverter759/1
  UnitConverter759/1 -> VOUTP_FDCTHCLEVentZStaSet1_enum/1  "VOUTP_FDCTHCLEVentZStaSet1_enum"
  VTHC_FDCTHCLEVentZStaSet2_enum/1 -> VTHC_FDCTHCLEVentZStaSet2_enum_Inproc/1  "VTHC_FDCTHCLEVentZStaSet2_enum"
  VTHC_FDCTHCLEVentZStaSet2_enum_Inproc/1 -> UnitConverter760/1
  UnitConverter760/1 -> VOUTP_FDCTHCLEVentZStaSet2_enum/1  "VOUTP_FDCTHCLEVentZStaSet2_enum"
  VTHC_FDCTHCLEVentZStaSet3_enum/1 -> VTHC_FDCTHCLEVentZStaSet3_enum_Inproc/1  "VTHC_FDCTHCLEVentZStaSet3_enum"
  VTHC_FDCTHCLEVentZStaSet3_enum_Inproc/1 -> UnitConverter761/1
  UnitConverter761/1 -> VOUTP_FDCTHCLEVentZStaSet3_enum/1  "VOUTP_FDCTHCLEVentZStaSet3_enum"
  VTHC_FDCTHCLEVentZStaSet4_enum/1 -> VTHC_FDCTHCLEVentZStaSet4_enum_Inproc/1  "VTHC_FDCTHCLEVentZStaSet4_enum"
  VTHC_FDCTHCLEVentZStaSet4_enum_Inproc/1 -> UnitConverter762/1
  UnitConverter762/1 -> VOUTP_FDCTHCLEVentZStaSet4_enum/1  "VOUTP_FDCTHCLEVentZStaSet4_enum"
  VTHC_FDCTHCLEVentZStaSet5_enum/1 -> VTHC_FDCTHCLEVentZStaSet5_enum_Inproc/1  "VTHC_FDCTHCLEVentZStaSet5_enum"
  VTHC_FDCTHCLEVentZStaSet5_enum_Inproc/1 -> UnitConverter763/1
  UnitConverter763/1 -> VOUTP_FDCTHCLEVentZStaSet5_enum/1  "VOUTP_FDCTHCLEVentZStaSet5_enum"
  VTHC_FDCTHCLEVentZStaSet7_enum/1 -> VTHC_FDCTHCLEVentZStaSet7_enum_Inproc/1  "VTHC_FDCTHCLEVentZStaSet7_enum"
  VTHC_FDCTHCLEVentZStaSet7_enum_Inproc/1 -> UnitConverter764/1
  UnitConverter764/1 -> VOUTP_FDCTHCLEVentZStaSet7_enum/1  "VOUTP_FDCTHCLEVentZStaSet7_enum"
  VTHC_FDCTHCCLEVentZStaSet1_enum/1 -> VTHC_FDCTHCCLEVentZStaSet1_enum_Inproc/1  "VTHC_FDCTHCCLEVentZStaSet1_enum"
  VTHC_FDCTHCCLEVentZStaSet1_enum_Inproc/1 -> UnitConverter765/1
  UnitConverter765/1 -> VOUTP_FDCTHCCLEVentZStaSet1_enum/1  "VOUTP_FDCTHCCLEVentZStaSet1_enum"
  VTHC_FDCTHCCLEVentZStaSet2_enum/1 -> VTHC_FDCTHCCLEVentZStaSet2_enum_Inproc/1  "VTHC_FDCTHCCLEVentZStaSet2_enum"
  VTHC_FDCTHCCLEVentZStaSet2_enum_Inproc/1 -> UnitConverter766/1
  UnitConverter766/1 -> VOUTP_FDCTHCCLEVentZStaSet2_enum/1  "VOUTP_FDCTHCCLEVentZStaSet2_enum"
  VTHC_FDCTHCCLEVentZStaSet3_enum/1 -> VTHC_FDCTHCCLEVentZStaSet3_enum_Inproc/1  "VTHC_FDCTHCCLEVentZStaSet3_enum"
  VTHC_FDCTHCCLEVentZStaSet3_enum_Inproc/1 -> UnitConverter767/1
  UnitConverter767/1 -> VOUTP_FDCTHCCLEVentZStaSet3_enum/1  "VOUTP_FDCTHCCLEVentZStaSet3_enum"
  VTHC_FDCTHCCLEVentZStaSet4_enum/1 -> VTHC_FDCTHCCLEVentZStaSet4_enum_Inproc/1  "VTHC_FDCTHCCLEVentZStaSet4_enum"
  VTHC_FDCTHCCLEVentZStaSet4_enum_Inproc/1 -> UnitConverter768/1
  UnitConverter768/1 -> VOUTP_FDCTHCCLEVentZStaSet4_enum/1  "VOUTP_FDCTHCCLEVentZStaSet4_enum"
  VTHC_FDCTHCCLEVentZStaSet5_enum/1 -> VTHC_FDCTHCCLEVentZStaSet5_enum_Inproc/1  "VTHC_FDCTHCCLEVentZStaSet5_enum"
  VTHC_FDCTHCCLEVentZStaSet5_enum_Inproc/1 -> UnitConverter769/1
  UnitConverter769/1 -> VOUTP_FDCTHCCLEVentZStaSet5_enum/1  "VOUTP_FDCTHCCLEVentZStaSet5_enum"
  VTHC_FDCTHCCLEVentZStaSet7_enum/1 -> VTHC_FDCTHCCLEVentZStaSet7_enum_Inproc/1  "VTHC_FDCTHCCLEVentZStaSet7_enum"
  VTHC_FDCTHCCLEVentZStaSet7_enum_Inproc/1 -> UnitConverter770/1
  UnitConverter770/1 -> VOUTP_FDCTHCCLEVentZStaSet7_enum/1  "VOUTP_FDCTHCCLEVentZStaSet7_enum"
  VTHC_FDCTHCREVentZStaSet1_enum/1 -> VTHC_FDCTHCREVentZStaSet1_enum_Inproc/1  "VTHC_FDCTHCREVentZStaSet1_enum"
  VTHC_FDCTHCREVentZStaSet1_enum_Inproc/1 -> UnitConverter771/1
  UnitConverter771/1 -> VOUTP_FDCTHCREVentZStaSet1_enum/1  "VOUTP_FDCTHCREVentZStaSet1_enum"
  VTHC_FDCTHCREVentZStaSet2_enum/1 -> VTHC_FDCTHCREVentZStaSet2_enum_Inproc/1  "VTHC_FDCTHCREVentZStaSet2_enum"
  VTHC_FDCTHCREVentZStaSet2_enum_Inproc/1 -> UnitConverter772/1
  UnitConverter772/1 -> VOUTP_FDCTHCREVentZStaSet2_enum/1  "VOUTP_FDCTHCREVentZStaSet2_enum"
  VTHC_FDCTHCREVentZStaSet3_enum/1 -> VTHC_FDCTHCREVentZStaSet3_enum_Inproc/1  "VTHC_FDCTHCREVentZStaSet3_enum"
  VTHC_FDCTHCREVentZStaSet3_enum_Inproc/1 -> UnitConverter773/1
  UnitConverter773/1 -> VOUTP_FDCTHCREVentZStaSet3_enum/1  "VOUTP_FDCTHCREVentZStaSet3_enum"
  VTHC_FDCTHCREVentZStaSet4_enum/1 -> VTHC_FDCTHCREVentZStaSet4_enum_Inproc/1  "VTHC_FDCTHCREVentZStaSet4_enum"
  VTHC_FDCTHCREVentZStaSet4_enum_Inproc/1 -> UnitConverter774/1
  UnitConverter774/1 -> VOUTP_FDCTHCREVentZStaSet4_enum/1  "VOUTP_FDCTHCREVentZStaSet4_enum"
  VTHC_FDCTHCREVentZStaSet5_enum/1 -> VTHC_FDCTHCREVentZStaSet5_enum_Inproc/1  "VTHC_FDCTHCREVentZStaSet5_enum"
  VTHC_FDCTHCREVentZStaSet5_enum_Inproc/1 -> UnitConverter775/1
  UnitConverter775/1 -> VOUTP_FDCTHCREVentZStaSet5_enum/1  "VOUTP_FDCTHCREVentZStaSet5_enum"
  VTHC_FDCTHCREVentZStaSet7_enum/1 -> VTHC_FDCTHCREVentZStaSet7_enum_Inproc/1  "VTHC_FDCTHCREVentZStaSet7_enum"
  VTHC_FDCTHCREVentZStaSet7_enum_Inproc/1 -> UnitConverter776/1
  UnitConverter776/1 -> VOUTP_FDCTHCREVentZStaSet7_enum/1  "VOUTP_FDCTHCREVentZStaSet7_enum"
  VTHC_FDCTHCCREVentZStaSet1_enum/1 -> VTHC_FDCTHCCREVentZStaSet1_enum_Inproc/1  "VTHC_FDCTHCCREVentZStaSet1_enum"
  VTHC_FDCTHCCREVentZStaSet1_enum_Inproc/1 -> UnitConverter777/1
  UnitConverter777/1 -> VOUTP_FDCTHCCREVentZStaSet1_enum/1  "VOUTP_FDCTHCCREVentZStaSet1_enum"
  VTHC_FDCTHCCREVentZStaSet2_enum/1 -> VTHC_FDCTHCCREVentZStaSet2_enum_Inproc/1  "VTHC_FDCTHCCREVentZStaSet2_enum"
  VTHC_FDCTHCCREVentZStaSet2_enum_Inproc/1 -> UnitConverter778/1
  UnitConverter778/1 -> VOUTP_FDCTHCCREVentZStaSet2_enum/1  "VOUTP_FDCTHCCREVentZStaSet2_enum"
  VTHC_FDCTHCCREVentZStaSet3_enum/1 -> VTHC_FDCTHCCREVentZStaSet3_enum_Inproc/1  "VTHC_FDCTHCCREVentZStaSet3_enum"
  VTHC_FDCTHCCREVentZStaSet3_enum_Inproc/1 -> UnitConverter779/1
  UnitConverter779/1 -> VOUTP_FDCTHCCREVentZStaSet3_enum/1  "VOUTP_FDCTHCCREVentZStaSet3_enum"
  VTHC_FDCTHCCREVentZStaSet4_enum/1 -> VTHC_FDCTHCCREVentZStaSet4_enum_Inproc/1  "VTHC_FDCTHCCREVentZStaSet4_enum"
  VTHC_FDCTHCCREVentZStaSet4_enum_Inproc/1 -> UnitConverter780/1
  UnitConverter780/1 -> VOUTP_FDCTHCCREVentZStaSet4_enum/1  "VOUTP_FDCTHCCREVentZStaSet4_enum"
  VTHC_FDCTHCCREVentZStaSet5_enum/1 -> VTHC_FDCTHCCREVentZStaSet5_enum_Inproc/1  "VTHC_FDCTHCCREVentZStaSet5_enum"
  VTHC_FDCTHCCREVentZStaSet5_enum_Inproc/1 -> UnitConverter781/1
  UnitConverter781/1 -> VOUTP_FDCTHCCREVentZStaSet5_enum/1  "VOUTP_FDCTHCCREVentZStaSet5_enum"
  VTHC_FDCTHCCREVentZStaSet7_enum/1 -> VTHC_FDCTHCCREVentZStaSet7_enum_Inproc/1  "VTHC_FDCTHCCREVentZStaSet7_enum"
  VTHC_FDCTHCCREVentZStaSet7_enum_Inproc/1 -> UnitConverter782/1
  UnitConverter782/1 -> VOUTP_FDCTHCCREVentZStaSet7_enum/1  "VOUTP_FDCTHCCREVentZStaSet7_enum"
  VTHC_FDCTHCLEVentYStaSet1_enum/1 -> VTHC_FDCTHCLEVentYStaSet1_enum_Inproc/1  "VTHC_FDCTHCLEVentYStaSet1_enum"
  VTHC_FDCTHCLEVentYStaSet1_enum_Inproc/1 -> UnitConverter783/1
  UnitConverter783/1 -> VOUTP_FDCTHCLEVentYStaSet1_enum/1  "VOUTP_FDCTHCLEVentYStaSet1_enum"
  VTHC_FDCTHCLEVentYStaSet2_enum/1 -> VTHC_FDCTHCLEVentYStaSet2_enum_Inproc/1  "VTHC_FDCTHCLEVentYStaSet2_enum"
  VTHC_FDCTHCLEVentYStaSet2_enum_Inproc/1 -> UnitConverter784/1
  UnitConverter784/1 -> VOUTP_FDCTHCLEVentYStaSet2_enum/1  "VOUTP_FDCTHCLEVentYStaSet2_enum"
  VTHC_FDCTHCLEVentYStaSet3_enum/1 -> VTHC_FDCTHCLEVentYStaSet3_enum_Inproc/1  "VTHC_FDCTHCLEVentYStaSet3_enum"
  VTHC_FDCTHCLEVentYStaSet3_enum_Inproc/1 -> UnitConverter785/1
  UnitConverter785/1 -> VOUTP_FDCTHCLEVentYStaSet3_enum/1  "VOUTP_FDCTHCLEVentYStaSet3_enum"
  VTHC_FDCTHCLEVentYStaSet4_enum/1 -> VTHC_FDCTHCLEVentYStaSet4_enum_Inproc/1  "VTHC_FDCTHCLEVentYStaSet4_enum"
  VTHC_FDCTHCLEVentYStaSet4_enum_Inproc/1 -> UnitConverter786/1
  UnitConverter786/1 -> VOUTP_FDCTHCLEVentYStaSet4_enum/1  "VOUTP_FDCTHCLEVentYStaSet4_enum"
  VTHC_FDCTHCLEVentYStaSet5_enum/1 -> VTHC_FDCTHCLEVentYStaSet5_enum_Inproc/1  "VTHC_FDCTHCLEVentYStaSet5_enum"
  VTHC_FDCTHCLEVentYStaSet5_enum_Inproc/1 -> UnitConverter787/1
  UnitConverter787/1 -> VOUTP_FDCTHCLEVentYStaSet5_enum/1  "VOUTP_FDCTHCLEVentYStaSet5_enum"
  VTHC_FDCTHCLEVentYStaSet7_enum/1 -> VTHC_FDCTHCLEVentYStaSet7_enum_Inproc/1  "VTHC_FDCTHCLEVentYStaSet7_enum"
  VTHC_FDCTHCLEVentYStaSet7_enum_Inproc/1 -> UnitConverter788/1
  UnitConverter788/1 -> VOUTP_FDCTHCLEVentYStaSet7_enum/1  "VOUTP_FDCTHCLEVentYStaSet7_enum"
  VTHC_FDCTHCCLEVentYStaSet1_enum/1 -> VTHC_FDCTHCCLEVentYStaSet1_enum_Inproc/1  "VTHC_FDCTHCCLEVentYStaSet1_enum"
  VTHC_FDCTHCCLEVentYStaSet1_enum_Inproc/1 -> UnitConverter789/1
  UnitConverter789/1 -> VOUTP_FDCTHCCLEVentYStaSet1_enum/1  "VOUTP_FDCTHCCLEVentYStaSet1_enum"
  VTHC_FDCTHCCLEVentYStaSet2_enum/1 -> VTHC_FDCTHCCLEVentYStaSet2_enum_Inproc/1  "VTHC_FDCTHCCLEVentYStaSet2_enum"
  VTHC_FDCTHCCLEVentYStaSet2_enum_Inproc/1 -> UnitConverter790/1
  UnitConverter790/1 -> VOUTP_FDCTHCCLEVentYStaSet2_enum/1  "VOUTP_FDCTHCCLEVentYStaSet2_enum"
  VTHC_FDCTHCCLEVentYStaSet3_enum/1 -> VTHC_FDCTHCCLEVentYStaSet3_enum_Inproc/1  "VTHC_FDCTHCCLEVentYStaSet3_enum"
  VTHC_FDCTHCCLEVentYStaSet3_enum_Inproc/1 -> UnitConverter791/1
  UnitConverter791/1 -> VOUTP_FDCTHCCLEVentYStaSet3_enum/1  "VOUTP_FDCTHCCLEVentYStaSet3_enum"
  VTHC_FDCTHCCLEVentYStaSet4_enum/1 -> VTHC_FDCTHCCLEVentYStaSet4_enum_Inproc/1  "VTHC_FDCTHCCLEVentYStaSet4_enum"
  VTHC_FDCTHCCLEVentYStaSet4_enum_Inproc/1 -> UnitConverter792/1
  UnitConverter792/1 -> VOUTP_FDCTHCCLEVentYStaSet4_enum/1  "VOUTP_FDCTHCCLEVentYStaSet4_enum"
  VTHC_FDCTHCCLEVentYStaSet5_enum/1 -> VTHC_FDCTHCCLEVentYStaSet5_enum_Inproc/1  "VTHC_FDCTHCCLEVentYStaSet5_enum"
  VTHC_FDCTHCCLEVentYStaSet5_enum_Inproc/1 -> UnitConverter793/1
  UnitConverter793/1 -> VOUTP_FDCTHCCLEVentYStaSet5_enum/1  "VOUTP_FDCTHCCLEVentYStaSet5_enum"
  VTHC_FDCTHCCLEVentYStaSet7_enum/1 -> VTHC_FDCTHCCLEVentYStaSet7_enum_Inproc/1  "VTHC_FDCTHCCLEVentYStaSet7_enum"
  VTHC_FDCTHCCLEVentYStaSet7_enum_Inproc/1 -> UnitConverter794/1
  UnitConverter794/1 -> VOUTP_FDCTHCCLEVentYStaSet7_enum/1  "VOUTP_FDCTHCCLEVentYStaSet7_enum"
  VTHC_FDCTHCREVentYStaSet1_enum/1 -> VTHC_FDCTHCREVentYStaSet1_enum_Inproc/1  "VTHC_FDCTHCREVentYStaSet1_enum"
  VTHC_FDCTHCREVentYStaSet1_enum_Inproc/1 -> UnitConverter795/1
  UnitConverter795/1 -> VOUTP_FDCTHCREVentYStaSet1_enum/1  "VOUTP_FDCTHCREVentYStaSet1_enum"
  VTHC_FDCTHCREVentYStaSet2_enum/1 -> VTHC_FDCTHCREVentYStaSet2_enum_Inproc/1  "VTHC_FDCTHCREVentYStaSet2_enum"
  VTHC_FDCTHCREVentYStaSet2_enum_Inproc/1 -> UnitConverter796/1
  UnitConverter796/1 -> VOUTP_FDCTHCREVentYStaSet2_enum/1  "VOUTP_FDCTHCREVentYStaSet2_enum"
  VTHC_FDCTHCREVentYStaSet3_enum/1 -> VTHC_FDCTHCREVentYStaSet3_enum_Inproc/1  "VTHC_FDCTHCREVentYStaSet3_enum"
  VTHC_FDCTHCREVentYStaSet3_enum_Inproc/1 -> UnitConverter797/1
  UnitConverter797/1 -> VOUTP_FDCTHCREVentYStaSet3_enum/1  "VOUTP_FDCTHCREVentYStaSet3_enum"
  VTHC_FDCTHCREVentYStaSet4_enum/1 -> VTHC_FDCTHCREVentYStaSet4_enum_Inproc/1  "VTHC_FDCTHCREVentYStaSet4_enum"
  VTHC_FDCTHCREVentYStaSet4_enum_Inproc/1 -> UnitConverter798/1
  UnitConverter798/1 -> VOUTP_FDCTHCREVentYStaSet4_enum/1  "VOUTP_FDCTHCREVentYStaSet4_enum"
  VTHC_FDCTHCREVentYStaSet5_enum/1 -> VTHC_FDCTHCREVentYStaSet5_enum_Inproc/1  "VTHC_FDCTHCREVentYStaSet5_enum"
  VTHC_FDCTHCREVentYStaSet5_enum_Inproc/1 -> UnitConverter799/1
  UnitConverter799/1 -> VOUTP_FDCTHCREVentYStaSet5_enum/1  "VOUTP_FDCTHCREVentYStaSet5_enum"
  VTHC_FDCTHCREVentYStaSet7_enum/1 -> VTHC_FDCTHCREVentYStaSet7_enum_Inproc/1  "VTHC_FDCTHCREVentYStaSet7_enum"
  VTHC_FDCTHCREVentYStaSet7_enum_Inproc/1 -> UnitConverter800/1
  UnitConverter800/1 -> VOUTP_FDCTHCREVentYStaSet7_enum/1  "VOUTP_FDCTHCREVentYStaSet7_enum"
  VTHC_FDCTHCCREVentYStaSet1_enum/1 -> VTHC_FDCTHCCREVentYStaSet1_enum_Inproc/1  "VTHC_FDCTHCCREVentYStaSet1_enum"
  VTHC_FDCTHCCREVentYStaSet1_enum_Inproc/1 -> UnitConverter801/1
  UnitConverter801/1 -> VOUTP_FDCTHCCREVentYStaSet1_enum/1  "VOUTP_FDCTHCCREVentYStaSet1_enum"
  VTHC_FDCTHCCREVentYStaSet2_enum/1 -> VTHC_FDCTHCCREVentYStaSet2_enum_Inproc/1  "VTHC_FDCTHCCREVentYStaSet2_enum"
  VTHC_FDCTHCCREVentYStaSet2_enum_Inproc/1 -> UnitConverter802/1
  UnitConverter802/1 -> VOUTP_FDCTHCCREVentYStaSet2_enum/1  "VOUTP_FDCTHCCREVentYStaSet2_enum"
  VTHC_FDCTHCCREVentYStaSet3_enum/1 -> VTHC_FDCTHCCREVentYStaSet3_enum_Inproc/1  "VTHC_FDCTHCCREVentYStaSet3_enum"
  VTHC_FDCTHCCREVentYStaSet3_enum_Inproc/1 -> UnitConverter803/1
  UnitConverter803/1 -> VOUTP_FDCTHCCREVentYStaSet3_enum/1  "VOUTP_FDCTHCCREVentYStaSet3_enum"
  VTHC_FDCTHCCREVentYStaSet4_enum/1 -> VTHC_FDCTHCCREVentYStaSet4_enum_Inproc/1  "VTHC_FDCTHCCREVentYStaSet4_enum"
  VTHC_FDCTHCCREVentYStaSet4_enum_Inproc/1 -> UnitConverter804/1
  UnitConverter804/1 -> VOUTP_FDCTHCCREVentYStaSet4_enum/1  "VOUTP_FDCTHCCREVentYStaSet4_enum"
  VTHC_FDCTHCCREVentYStaSet5_enum/1 -> VTHC_FDCTHCCREVentYStaSet5_enum_Inproc/1  "VTHC_FDCTHCCREVentYStaSet5_enum"
  VTHC_FDCTHCCREVentYStaSet5_enum_Inproc/1 -> UnitConverter805/1
  UnitConverter805/1 -> VOUTP_FDCTHCCREVentYStaSet5_enum/1  "VOUTP_FDCTHCCREVentYStaSet5_enum"
  VTHC_FDCTHCCREVentYStaSet7_enum/1 -> VTHC_FDCTHCCREVentYStaSet7_enum_Inproc/1  "VTHC_FDCTHCCREVentYStaSet7_enum"
  VTHC_FDCTHCCREVentYStaSet7_enum_Inproc/1 -> UnitConverter806/1
  UnitConverter806/1 -> VOUTP_FDCTHCCREVentYStaSet7_enum/1  "VOUTP_FDCTHCCREVentYStaSet7_enum"
  VTHC_SettempZon1Set1_enum/1 -> VTHC_SettempZon1Set1_enum_Inproc/1  "VTHC_SettempZon1Set1_enum"
  VTHC_SettempZon1Set1_enum_Inproc/1 -> UnitConverter807/1
  UnitConverter807/1 -> VOUTP_SettempZon1Set1_enum/1  "VOUTP_SettempZon1Set1_enum"
  VTHC_SettempZon1Set2_enum/1 -> VTHC_SettempZon1Set2_enum_Inproc/1  "VTHC_SettempZon1Set2_enum"
  VTHC_SettempZon1Set2_enum_Inproc/1 -> UnitConverter808/1
  UnitConverter808/1 -> VOUTP_SettempZon1Set2_enum/1  "VOUTP_SettempZon1Set2_enum"
  VTHC_SettempZon1Set3_enum/1 -> VTHC_SettempZon1Set3_enum_Inproc/1  "VTHC_SettempZon1Set3_enum"
  VTHC_SettempZon1Set3_enum_Inproc/1 -> UnitConverter809/1
  UnitConverter809/1 -> VOUTP_SettempZon1Set3_enum/1  "VOUTP_SettempZon1Set3_enum"
  VTHC_SettempZon1Set4_enum/1 -> VTHC_SettempZon1Set4_enum_Inproc/1  "VTHC_SettempZon1Set4_enum"
  VTHC_SettempZon1Set4_enum_Inproc/1 -> UnitConverter810/1
  UnitConverter810/1 -> VOUTP_SettempZon1Set4_enum/1  "VOUTP_SettempZon1Set4_enum"
  VTHC_SettempZon1Set5_enum/1 -> VTHC_SettempZon1Set5_enum_Inproc/1  "VTHC_SettempZon1Set5_enum"
  VTHC_SettempZon1Set5_enum_Inproc/1 -> UnitConverter811/1
  UnitConverter811/1 -> VOUTP_SettempZon1Set5_enum/1  "VOUTP_SettempZon1Set5_enum"
  VTHC_SettempZon1Set7_enum/1 -> VTHC_SettempZon1Set7_enum_Inproc/1  "VTHC_SettempZon1Set7_enum"
  VTHC_SettempZon1Set7_enum_Inproc/1 -> UnitConverter812/1
  UnitConverter812/1 -> VOUTP_SettempZon1Set7_enum/1  "VOUTP_SettempZon1Set7_enum"
  VTHC_ACModeSet123_enum/1 -> VTHC_ACModeSet123_enum_Inproc/1  "VTHC_ACModeSet123_enum"
  VTHC_ACModeSet123_enum_Inproc/1 -> UnitConverter813/1
  UnitConverter813/1 -> VOUTP_ACModeSet123_enum/1  "VOUTP_ACModeSet123_enum"
  VTHC_ACModeSet457_enum/1 -> VTHC_ACModeSet457_enum_Inproc/1  "VTHC_ACModeSet457_enum"
  VTHC_ACModeSet457_enum_Inproc/1 -> UnitConverter814/1
  UnitConverter814/1 -> VOUTP_ACModeSet457_enum/1  "VOUTP_ACModeSet457_enum"
  VTHC_FACESet_enum/1 -> VTHC_FACESet_enum_Inproc/1  "VTHC_FACESet_enum"
  VTHC_FACESet_enum_Inproc/1 -> UnitConverter815/1
  UnitConverter815/1 -> VOUTP_FACESet_enum/1  "VOUTP_FACESet_enum"
  VTHC_FOOTSet_enum/1 -> VTHC_FOOTSet_enum_Inproc/1  "VTHC_FOOTSet_enum"
  VTHC_FOOTSet_enum_Inproc/1 -> UnitConverter816/1
  UnitConverter816/1 -> VOUTP_FOOTSet_enum/1  "VOUTP_FOOTSet_enum"
  VTHC_FrostSet_enum/1 -> VTHC_FrostSet_enum_Inproc/1  "VTHC_FrostSet_enum"
  VTHC_FrostSet_enum_Inproc/1 -> UnitConverter817/1
  UnitConverter817/1 -> VOUTP_FrostSet_enum/1  "VOUTP_FrostSet_enum"
  VTHC_LVentEN_flg/1 -> VTHC_LVentEN_flg_Inproc/1  "VTHC_LVentEN_flg"
  VTHC_LVentEN_flg_Inproc/1 -> UnitConverter818/1
  UnitConverter818/1 -> VOUTP_LVentEN_flg/1  "VOUTP_LVentEN_flg"
  VTHC_CLVentEN_flg/1 -> VTHC_CLVentEN_flg_Inproc/1  "VTHC_CLVentEN_flg"
  VTHC_CLVentEN_flg_Inproc/1 -> UnitConverter819/1
  UnitConverter819/1 -> VOUTP_CLVentEN_flg/1  "VOUTP_CLVentEN_flg"
  VTHC_RVentEN_flg/1 -> VTHC_RVentEN_flg_Inproc/1  "VTHC_RVentEN_flg"
  VTHC_RVentEN_flg_Inproc/1 -> UnitConverter820/1
  UnitConverter820/1 -> VOUTP_RVentEN_flg/1  "VOUTP_RVentEN_flg"
  VTHC_CRVentEN_flg/1 -> VTHC_CRVentEN_flg_Inproc/1  "VTHC_CRVentEN_flg"
  VTHC_CRVentEN_flg_Inproc/1 -> UnitConverter821/1
  UnitConverter821/1 -> VOUTP_CRVentEN_flg/1  "VOUTP_CRVentEN_flg"
  VTHC_FDCFGSLearnCmd_enum/1 -> VTHC_FDCFGSLearnCmd_enum_Inproc/1  "VTHC_FDCFGSLearnCmd_enum"
  VTHC_FDCFGSLearnCmd_enum_Inproc/1 -> UnitConverter822/1
  UnitConverter822/1 -> VOUTP_FDCFGSLearnCmd_enum/1  "VOUTP_FDCFGSLearnCmd_enum"
  VTHC_FDCFGSFuncSta_flg/1 -> VTHC_FDCFGSFuncSta_flg_Inproc/1  "VTHC_FDCFGSFuncSta_flg"
  VTHC_FDCFGSFuncSta_flg_Inproc/1 -> UnitConverter823/1
  UnitConverter823/1 -> VOUTP_FDCFGSFuncSta_flg/1  "VOUTP_FDCFGSFuncSta_flg"
  VTHC_THSysErrlampReq_flg/1 -> VTHC_THSysErrlampReq_flg_Inproc/1  "VTHC_THSysErrlampReq_flg"
  VTHC_THSysErrlampReq_flg_Inproc/1 -> UnitConverter824/1
  UnitConverter824/1 -> VOUTP_THSysErrlampReq_flg/1  "VOUTP_THSysErrlampReq_flg"
  VTHC_sigCbnPTCPwrAct_W/1 -> VTHC_sigCbnPTCPwrAct_W_Inproc/1  "VTHC_sigCbnPTCPwrAct_W"
  VTHC_sigCbnPTCPwrAct_W_Inproc/1 -> UnitConverter825/1
  UnitConverter825/1 -> VOUTP_sigCbnPTCPwrAct_W/1  "VOUTP_sigCbnPTCPwrAct_W"
  VTPM_LFBatWarn_flg/1 -> VTPM_LFBatWarn_flg_Inproc/1  "VTPM_LFBatWarn_flg"
  VTPM_LFBatWarn_flg_Inproc/1 -> UnitConverter826/1
  UnitConverter826/1 -> VOUTP_LFBatWarn_flg/1  "VOUTP_LFBatWarn_flg"
  VTPM_RFBatWarn_flg/1 -> VTPM_RFBatWarn_flg_Inproc/1  "VTPM_RFBatWarn_flg"
  VTPM_RFBatWarn_flg_Inproc/1 -> UnitConverter827/1
  UnitConverter827/1 -> VOUTP_RFBatWarn_flg/1  "VOUTP_RFBatWarn_flg"
  VTPM_LRBatWarn_flg/1 -> VTPM_LRBatWarn_flg_Inproc/1  "VTPM_LRBatWarn_flg"
  VTPM_LRBatWarn_flg_Inproc/1 -> UnitConverter828/1
  UnitConverter828/1 -> VOUTP_LRBatWarn_flg/1  "VOUTP_LRBatWarn_flg"
  VTPM_RRBatWarn_flg/1 -> VTPM_RRBatWarn_flg_Inproc/1  "VTPM_RRBatWarn_flg"
  VTPM_RRBatWarn_flg_Inproc/1 -> UnitConverter829/1
  UnitConverter829/1 -> VOUTP_RRBatWarn_flg/1  "VOUTP_RRBatWarn_flg"
  VTPM_LFWheelPress_raw8/1 -> VTPM_LFWheelPress_raw8_Inproc/1  "VTPM_LFWheelPress_raw8"
  VTPM_LFWheelPress_raw8_Inproc/1 -> UnitConverter830/1
  UnitConverter830/1 -> VOUTP_LFWheelPress_raw8/1  "VOUTP_LFWheelPress_raw8"
  VTPM_RFWheelPress_raw8/1 -> VTPM_RFWheelPress_raw8_Inproc/1  "VTPM_RFWheelPress_raw8"
  VTPM_RFWheelPress_raw8_Inproc/1 -> UnitConverter831/1
  UnitConverter831/1 -> VOUTP_RFWheelPress_raw8/1  "VOUTP_RFWheelPress_raw8"
  VTPM_LRWheelPress_raw8/1 -> VTPM_LRWheelPress_raw8_Inproc/1  "VTPM_LRWheelPress_raw8"
  VTPM_LRWheelPress_raw8_Inproc/1 -> UnitConverter832/1
  UnitConverter832/1 -> VOUTP_LRWheelPress_raw8/1  "VOUTP_LRWheelPress_raw8"
  VTPM_RRWheelPress_raw8/1 -> VTPM_RRWheelPress_raw8_Inproc/1  "VTPM_RRWheelPress_raw8"
  VTPM_RRWheelPress_raw8_Inproc/1 -> UnitConverter833/1
  UnitConverter833/1 -> VOUTP_RRWheelPress_raw8/1  "VOUTP_RRWheelPress_raw8"
  VTPM_LFWheelTemp_C/1 -> VTPM_LFWheelTemp_C_Inproc/1  "VTPM_LFWheelTemp_C"
  VTPM_LFWheelTemp_C_Inproc/1 -> UnitConverter834/1
  UnitConverter834/1 -> VOUTP_LFWheelTemp_C/1  "VOUTP_LFWheelTemp_C"
  VTPM_RFWheelTemp_C/1 -> VTPM_RFWheelTemp_C_Inproc/1  "VTPM_RFWheelTemp_C"
  VTPM_RFWheelTemp_C_Inproc/1 -> UnitConverter835/1
  UnitConverter835/1 -> VOUTP_RFWheelTemp_C/1  "VOUTP_RFWheelTemp_C"
  VTPM_LRWheelTemp_C/1 -> VTPM_LRWheelTemp_C_Inproc/1  "VTPM_LRWheelTemp_C"
  VTPM_LRWheelTemp_C_Inproc/1 -> UnitConverter836/1
  UnitConverter836/1 -> VOUTP_LRWheelTemp_C/1  "VOUTP_LRWheelTemp_C"
  VTPM_RRWheelTemp_C/1 -> VTPM_RRWheelTemp_C_Inproc/1  "VTPM_RRWheelTemp_C"
  VTPM_RRWheelTemp_C_Inproc/1 -> UnitConverter837/1
  UnitConverter837/1 -> VOUTP_RRWheelTemp_C/1  "VOUTP_RRWheelTemp_C"
  VTPM_LFSensorFail_flg/1 -> VTPM_LFSensorFail_flg_Inproc/1  "VTPM_LFSensorFail_flg"
  VTPM_LFSensorFail_flg_Inproc/1 -> UnitConverter838/1
  UnitConverter838/1 -> VOUTP_LFSensorFail_flg/1  "VOUTP_LFSensorFail_flg"
  VTPM_RFSensorFail_flg/1 -> VTPM_RFSensorFail_flg_Inproc/1  "VTPM_RFSensorFail_flg"
  VTPM_RFSensorFail_flg_Inproc/1 -> UnitConverter839/1
  UnitConverter839/1 -> VOUTP_RFSensorFail_flg/1  "VOUTP_RFSensorFail_flg"
  VTPM_LRSensorFail_flg/1 -> VTPM_LRSensorFail_flg_Inproc/1  "VTPM_LRSensorFail_flg"
  VTPM_LRSensorFail_flg_Inproc/1 -> UnitConverter840/1
  UnitConverter840/1 -> VOUTP_LRSensorFail_flg/1  "VOUTP_LRSensorFail_flg"
  VTPM_RRSensorFail_flg/1 -> VTPM_RRSensorFail_flg_Inproc/1  "VTPM_RRSensorFail_flg"
  VTPM_RRSensorFail_flg_Inproc/1 -> UnitConverter841/1
  UnitConverter841/1 -> VOUTP_RRSensorFail_flg/1  "VOUTP_RRSensorFail_flg"
  VTPM_LFWheelDebug_flg/1 -> VTPM_LFWheelDebug_flg_Inproc/1  "VTPM_LFWheelDebug_flg"
  VTPM_LFWheelDebug_flg_Inproc/1 -> UnitConverter842/1
  UnitConverter842/1 -> VOUTP_LFWheelDebug_flg/1  "VOUTP_LFWheelDebug_flg"
  VTPM_LRWheelDebug_flg/1 -> VTPM_LRWheelDebug_flg_Inproc/1  "VTPM_LRWheelDebug_flg"
  VTPM_LRWheelDebug_flg_Inproc/1 -> UnitConverter843/1
  UnitConverter843/1 -> VOUTP_LRWheelDebug_flg/1  "VOUTP_LRWheelDebug_flg"
  VTPM_RFWheelDebug_flg/1 -> VTPM_RFWheelDebug_flg_Inproc/1  "VTPM_RFWheelDebug_flg"
  VTPM_RFWheelDebug_flg_Inproc/1 -> UnitConverter844/1
  UnitConverter844/1 -> VOUTP_RFWheelDebug_flg/1  "VOUTP_RFWheelDebug_flg"
  VTPM_RRWheelDebug_flg/1 -> VTPM_RRWheelDebug_flg_Inproc/1  "VTPM_RRWheelDebug_flg"
  VTPM_RRWheelDebug_flg_Inproc/1 -> UnitConverter845/1
  UnitConverter845/1 -> VOUTP_RRWheelDebug_flg/1  "VOUTP_RRWheelDebug_flg"
  VTPM_TPMSResButtAllow_flg/1 -> VTPM_TPMSResButtAllow_flg_Inproc/1  "VTPM_TPMSResButtAllow_flg"
  VTPM_TPMSResButtAllow_flg_Inproc/1 -> UnitConverter846/1
  UnitConverter846/1 -> VOUTP_TPMSResButtAllow_flg/1  "VOUTP_TPMSResButtAllow_flg"
  VTPM_TPMSCaliButtAllow_flg/1 -> VTPM_TPMSCaliButtAllow_flg_Inproc/1  "VTPM_TPMSCaliButtAllow_flg"
  VTPM_TPMSCaliButtAllow_flg_Inproc/1 -> UnitConverter847/1
  UnitConverter847/1 -> VOUTP_TPMSCaliButtAllow_flg/1  "VOUTP_TPMSCaliButtAllow_flg"
  VTPM_LFPressIndi_enum/1 -> VTPM_LFPressIndi_enum_Inproc/1  "VTPM_LFPressIndi_enum"
  VTPM_LFPressIndi_enum_Inproc/1 -> UnitConverter848/1
  UnitConverter848/1 -> VOUTP_LFPressIndi_enum/1  "VOUTP_LFPressIndi_enum"
  VTPM_RFPressIndi_enum/1 -> VTPM_RFPressIndi_enum_Inproc/1  "VTPM_RFPressIndi_enum"
  VTPM_RFPressIndi_enum_Inproc/1 -> UnitConverter849/1
  UnitConverter849/1 -> VOUTP_RFPressIndi_enum/1  "VOUTP_RFPressIndi_enum"
  VTPM_LRPressIndi_enum/1 -> VTPM_LRPressIndi_enum_Inproc/1  "VTPM_LRPressIndi_enum"
  VTPM_LRPressIndi_enum_Inproc/1 -> UnitConverter850/1
  UnitConverter850/1 -> VOUTP_LRPressIndi_enum/1  "VOUTP_LRPressIndi_enum"
  VTPM_RRPressIndi_enum/1 -> VTPM_RRPressIndi_enum_Inproc/1  "VTPM_RRPressIndi_enum"
  VTPM_RRPressIndi_enum_Inproc/1 -> UnitConverter851/1
  UnitConverter851/1 -> VOUTP_RRPressIndi_enum/1  "VOUTP_RRPressIndi_enum"
  VTPM_TPMSWarnIndi_enum/1 -> VTPM_TPMSWarnIndi_enum_Inproc/1  "VTPM_TPMSWarnIndi_enum"
  VTPM_TPMSWarnIndi_enum_Inproc/1 -> UnitConverter852/1
  UnitConverter852/1 -> VOUTP_TPMSWarnIndi_enum/1  "VOUTP_TPMSWarnIndi_enum"
  VTPM_LFWheelTmpIndi_flg/1 -> VTPM_LFWheelTmpIndi_flg_Inproc/1  "VTPM_LFWheelTmpIndi_flg"
  VTPM_LFWheelTmpIndi_flg_Inproc/1 -> UnitConverter853/1
  UnitConverter853/1 -> VOUTP_LFWheelTmpIndi_flg/1  "VOUTP_LFWheelTmpIndi_flg"
  VTPM_RFWheelTmpIndi_flg/1 -> VTPM_RFWheelTmpIndi_flg_Inproc/1  "VTPM_RFWheelTmpIndi_flg"
  VTPM_RFWheelTmpIndi_flg_Inproc/1 -> UnitConverter854/1
  UnitConverter854/1 -> VOUTP_RFWheelTmpIndi_flg/1  "VOUTP_RFWheelTmpIndi_flg"
  VTPM_LRWheelTmpIndi_flg/1 -> VTPM_LRWheelTmpIndi_flg_Inproc/1  "VTPM_LRWheelTmpIndi_flg"
  VTPM_LRWheelTmpIndi_flg_Inproc/1 -> UnitConverter855/1
  UnitConverter855/1 -> VOUTP_LRWheelTmpIndi_flg/1  "VOUTP_LRWheelTmpIndi_flg"
  VTPM_RRWheelTmpIndi_flg/1 -> VTPM_RRWheelTmpIndi_flg_Inproc/1  "VTPM_RRWheelTmpIndi_flg"
  VTPM_RRWheelTmpIndi_flg_Inproc/1 -> UnitConverter856/1
  UnitConverter856/1 -> VOUTP_RRWheelTmpIndi_flg/1  "VOUTP_RRWheelTmpIndi_flg"
  VTPM_LFWheelPSW_raw8/1 -> VTPM_LFWheelPSW_raw8_Inproc/1  "VTPM_LFWheelPSW_raw8"
  VTPM_LFWheelPSW_raw8_Inproc/1 -> UnitConverter857/1
  UnitConverter857/1 -> VOUTP_LFWheelPSW_raw8/1  "VOUTP_LFWheelPSW_raw8"
  VTPM_LRWheelPSW_raw8/1 -> VTPM_LRWheelPSW_raw8_Inproc/1  "VTPM_LRWheelPSW_raw8"
  VTPM_LRWheelPSW_raw8_Inproc/1 -> UnitConverter858/1
  UnitConverter858/1 -> VOUTP_LRWheelPSW_raw8/1  "VOUTP_LRWheelPSW_raw8"
  VTPM_RFWheelPSW_raw8/1 -> VTPM_RFWheelPSW_raw8_Inproc/1  "VTPM_RFWheelPSW_raw8"
  VTPM_RFWheelPSW_raw8_Inproc/1 -> UnitConverter859/1
  UnitConverter859/1 -> VOUTP_RFWheelPSW_raw8/1  "VOUTP_RFWheelPSW_raw8"
  VTPM_RRWheelPSW_raw8/1 -> VTPM_RRWheelPSW_raw8_Inproc/1  "VTPM_RRWheelPSW_raw8"
  VTPM_RRWheelPSW_raw8_Inproc/1 -> UnitConverter860/1
  UnitConverter860/1 -> VOUTP_RRWheelPSW_raw8/1  "VOUTP_RRWheelPSW_raw8"
  VTPM_CWheelTips_enum/1 -> VTPM_CWheelTips_enum_Inproc/1  "VTPM_CWheelTips_enum"
  VTPM_CWheelTips_enum_Inproc/1 -> UnitConverter861/1
  UnitConverter861/1 -> VOUTP_CWheelTips_enum/1  "VOUTP_CWheelTips_enum"
  VTPM_AutoLTips_enum/1 -> VTPM_AutoLTips_enum_Inproc/1  "VTPM_AutoLTips_enum"
  VTPM_AutoLTips_enum_Inproc/1 -> UnitConverter862/1
  UnitConverter862/1 -> VOUTP_AutoLTips_enum/1  "VOUTP_AutoLTips_enum"
  VTPM_LFSensorMode_flg/1 -> VTPM_LFSensorMode_flg_Inproc/1  "VTPM_LFSensorMode_flg"
  VTPM_LFSensorMode_flg_Inproc/1 -> UnitConverter863/1
  UnitConverter863/1 -> VOUTP_LFSensorMode_flg/1  "VOUTP_LFSensorMode_flg"
  VTPM_RFSensorMode_flg/1 -> VTPM_RFSensorMode_flg_Inproc/1  "VTPM_RFSensorMode_flg"
  VTPM_RFSensorMode_flg_Inproc/1 -> UnitConverter864/1
  UnitConverter864/1 -> VOUTP_RFSensorMode_flg/1  "VOUTP_RFSensorMode_flg"
  VTPM_LRSensorMode_flg/1 -> VTPM_LRSensorMode_flg_Inproc/1  "VTPM_LRSensorMode_flg"
  VTPM_LRSensorMode_flg_Inproc/1 -> UnitConverter865/1
  UnitConverter865/1 -> VOUTP_LRSensorMode_flg/1  "VOUTP_LRSensorMode_flg"
  VTPM_RRSensorMode_flg/1 -> VTPM_RRSensorMode_flg_Inproc/1  "VTPM_RRSensorMode_flg"
  VTPM_RRSensorMode_flg_Inproc/1 -> UnitConverter866/1
  UnitConverter866/1 -> VOUTP_RRSensorMode_flg/1  "VOUTP_RRSensorMode_flg"
  VTPM_S1ID_raw32/1 -> VTPM_S1ID_raw32_Inproc/1  "VTPM_S1ID_raw32"
  VTPM_S1ID_raw32_Inproc/1 -> UnitConverter867/1
  UnitConverter867/1 -> VOUTP_S1ID_raw32/1  "VOUTP_S1ID_raw32"
  VTPM_S2ID_raw32/1 -> VTPM_S2ID_raw32_Inproc/1  "VTPM_S2ID_raw32"
  VTPM_S2ID_raw32_Inproc/1 -> UnitConverter868/1
  UnitConverter868/1 -> VOUTP_S2ID_raw32/1  "VOUTP_S2ID_raw32"
  VTPM_S3ID_raw32/1 -> VTPM_S3ID_raw32_Inproc/1  "VTPM_S3ID_raw32"
  VTPM_S3ID_raw32_Inproc/1 -> UnitConverter869/1
  UnitConverter869/1 -> VOUTP_S3ID_raw32/1  "VOUTP_S3ID_raw32"
  VTPM_S4ID_raw32/1 -> VTPM_S4ID_raw32_Inproc/1  "VTPM_S4ID_raw32"
  VTPM_S4ID_raw32_Inproc/1 -> UnitConverter870/1
  UnitConverter870/1 -> VOUTP_S4ID_raw32/1  "VOUTP_S4ID_raw32"
  VTPM_S1L_enum/1 -> VTPM_S1L_enum_Inproc/1  "VTPM_S1L_enum"
  VTPM_S1L_enum_Inproc/1 -> UnitConverter871/1
  UnitConverter871/1 -> VOUTP_S1L_enum/1  "VOUTP_S1L_enum"
  VTPM_S2L_enum/1 -> VTPM_S2L_enum_Inproc/1  "VTPM_S2L_enum"
  VTPM_S2L_enum_Inproc/1 -> UnitConverter872/1
  UnitConverter872/1 -> VOUTP_S2L_enum/1  "VOUTP_S2L_enum"
  VTPM_S3L_enum/1 -> VTPM_S3L_enum_Inproc/1  "VTPM_S3L_enum"
  VTPM_S3L_enum_Inproc/1 -> UnitConverter873/1
  UnitConverter873/1 -> VOUTP_S3L_enum/1  "VOUTP_S3L_enum"
  VTPM_S4L_enum/1 -> VTPM_S4L_enum_Inproc/1  "VTPM_S4L_enum"
  VTPM_S4L_enum_Inproc/1 -> UnitConverter874/1
  UnitConverter874/1 -> VOUTP_S4L_enum/1  "VOUTP_S4L_enum"
  VTPM_ALFin_flg/1 -> VTPM_ALFin_flg_Inproc/1  "VTPM_ALFin_flg"
  VTPM_ALFin_flg_Inproc/1 -> UnitConverter875/1
  UnitConverter875/1 -> VOUTP_ALFin_flg/1  "VOUTP_ALFin_flg"
  VTPM_LFP20_raw8/1 -> VTPM_LFP20_raw8_Inproc/1  "VTPM_LFP20_raw8"
  VTPM_LFP20_raw8_Inproc/1 -> UnitConverter876/1
  UnitConverter876/1 -> VOUTP_LFP20_raw8/1  "VOUTP_LFP20_raw8"
  VTPM_RFP20_raw8/1 -> VTPM_RFP20_raw8_Inproc/1  "VTPM_RFP20_raw8"
  VTPM_RFP20_raw8_Inproc/1 -> UnitConverter877/1
  UnitConverter877/1 -> VOUTP_RFP20_raw8/1  "VOUTP_RFP20_raw8"
  VTPM_LRP20_raw8/1 -> VTPM_LRP20_raw8_Inproc/1  "VTPM_LRP20_raw8"
  VTPM_LRP20_raw8_Inproc/1 -> UnitConverter878/1
  UnitConverter878/1 -> VOUTP_LRP20_raw8/1  "VOUTP_LRP20_raw8"
  VTPM_RRP20_raw8/1 -> VTPM_RRP20_raw8_Inproc/1  "VTPM_RRP20_raw8"
  VTPM_RRP20_raw8_Inproc/1 -> UnitConverter879/1
  UnitConverter879/1 -> VOUTP_RRP20_raw8/1  "VOUTP_RRP20_raw8"
  VTPM_FAT_flg/1 -> VTPM_FAT_flg_Inproc/1  "VTPM_FAT_flg"
  VTPM_FAT_flg_Inproc/1 -> UnitConverter880/1
  UnitConverter880/1 -> VOUTP_FAT_flg/1  "VOUTP_FAT_flg"
  VTPM_IDin_raw32/1 -> VTPM_IDin_raw32_Inproc/1  "VTPM_IDin_raw32"
  VTPM_IDin_raw32_Inproc/1 -> UnitConverter881/1
  UnitConverter881/1 -> VOUTP_IDin_raw32/1  "VOUTP_IDin_raw32"
  VTPM_S1WheelDebugALTU_pct/1 -> VTPM_S1WheelDebugALTU_pct_Inproc/1  "VTPM_S1WheelDebugALTU_pct"
  VTPM_S1WheelDebugALTU_pct_Inproc/1 -> UnitConverter882/1
  UnitConverter882/1 -> VOUTP_S1WheelDebugALTU_pct/1  "VOUTP_S1WheelDebugALTU_pct"
  VTPM_S2WheelDebugALTU_pct/1 -> VTPM_S2WheelDebugALTU_pct_Inproc/1  "VTPM_S2WheelDebugALTU_pct"
  VTPM_S2WheelDebugALTU_pct_Inproc/1 -> UnitConverter883/1
  UnitConverter883/1 -> VOUTP_S2WheelDebugALTU_pct/1  "VOUTP_S2WheelDebugALTU_pct"
  VTPM_S3WheelDebugALTU_pct/1 -> VTPM_S3WheelDebugALTU_pct_Inproc/1  "VTPM_S3WheelDebugALTU_pct"
  VTPM_S3WheelDebugALTU_pct_Inproc/1 -> UnitConverter884/1
  UnitConverter884/1 -> VOUTP_S3WheelDebugALTU_pct/1  "VOUTP_S3WheelDebugALTU_pct"
  VTPM_S4WheelDebugALTU_pct/1 -> VTPM_S4WheelDebugALTU_pct_Inproc/1  "VTPM_S4WheelDebugALTU_pct"
  VTPM_S4WheelDebugALTU_pct_Inproc/1 -> UnitConverter885/1
  UnitConverter885/1 -> VOUTP_S4WheelDebugALTU_pct/1  "VOUTP_S4WheelDebugALTU_pct"
  VTPM_ID1messageALTU_raw8/1 -> VTPM_ID1messageALTU_raw8_Inproc/1  "VTPM_ID1messageALTU_raw8"
  VTPM_ID1messageALTU_raw8_Inproc/1 -> UnitConverter886/1
  UnitConverter886/1 -> VOUTP_ID1messageALTU_raw8/1  "VOUTP_ID1messageALTU_raw8"
  VTPM_ID2messageALTU_raw8/1 -> VTPM_ID2messageALTU_raw8_Inproc/1  "VTPM_ID2messageALTU_raw8"
  VTPM_ID2messageALTU_raw8_Inproc/1 -> UnitConverter887/1
  UnitConverter887/1 -> VOUTP_ID2messageALTU_raw8/1  "VOUTP_ID2messageALTU_raw8"
  VTPM_ID3messageALTU_raw8/1 -> VTPM_ID3messageALTU_raw8_Inproc/1  "VTPM_ID3messageALTU_raw8"
  VTPM_ID3messageALTU_raw8_Inproc/1 -> UnitConverter888/1
  UnitConverter888/1 -> VOUTP_ID3messageALTU_raw8/1  "VOUTP_ID3messageALTU_raw8"
  VTPM_ID4messageALTU_raw8/1 -> VTPM_ID4messageALTU_raw8_Inproc/1  "VTPM_ID4messageALTU_raw8"
  VTPM_ID4messageALTU_raw8_Inproc/1 -> UnitConverter889/1
  UnitConverter889/1 -> VOUTP_ID4messageALTU_raw8/1  "VOUTP_ID4messageALTU_raw8"
  VTPM_Chkfin_flg/1 -> VTPM_Chkfin_flg_Inproc/1  "VTPM_Chkfin_flg"
  VTPM_Chkfin_flg_Inproc/1 -> UnitConverter890/1
  UnitConverter890/1 -> VOUTP_Chkfin_flg/1  "VOUTP_Chkfin_flg"
  VTPM_SetIDLoc_flg/1 -> VTPM_SetIDLoc_flg_Inproc/1  "VTPM_SetIDLoc_flg"
  VTPM_SetIDLoc_flg_Inproc/1 -> UnitConverter891/1
  UnitConverter891/1 -> VOUTP_SetIDLoc_flg/1  "VOUTP_SetIDLoc_flg"
  VTPM_TPMSStorge_flg/1 -> VTPM_TPMSStorge_flg_Inproc/1  "VTPM_TPMSStorge_flg"
  VTPM_TPMSStorge_flg_Inproc/1 -> UnitConverter892/1
  UnitConverter892/1 -> VOUTP_TPMSStorge_flg/1  "VOUTP_TPMSStorge_flg"
  VTPM_ChkStorge_flg/1 -> VTPM_ChkStorge_flg_Inproc/1  "VTPM_ChkStorge_flg"
  VTPM_ChkStorge_flg_Inproc/1 -> UnitConverter893/1
  UnitConverter893/1 -> VOUTP_ChkStorge_flg/1  "VOUTP_ChkStorge_flg"
  VTPM_TPMSResButt_flg/1 -> VTPM_TPMSResButt_flg_Inproc/1  "VTPM_TPMSResButt_flg"
  VTPM_TPMSResButt_flg_Inproc/1 -> UnitConverter894/1
  UnitConverter894/1 -> VOUTP_TPMSResButt_flg/1  "VOUTP_TPMSResButt_flg"
  VTPM_LFPindi_enum/1 -> VTPM_LFPindi_enum_Inproc/1  "VTPM_LFPindi_enum"
  VTPM_LFPindi_enum_Inproc/1 -> UnitConverter895/1
  UnitConverter895/1 -> VOUTP_LFPindi_enum/1  "VOUTP_LFPindi_enum"
  VTPM_RFPind_enum/1 -> VTPM_RFPind_enum_Inproc/1  "VTPM_RFPind_enum"
  VTPM_RFPind_enum_Inproc/1 -> UnitConverter896/1
  UnitConverter896/1 -> VOUTP_RFPind_enum/1  "VOUTP_RFPind_enum"
  VTPM_LRPindi_enum/1 -> VTPM_LRPindi_enum_Inproc/1  "VTPM_LRPindi_enum"
  VTPM_LRPindi_enum_Inproc/1 -> UnitConverter897/1
  UnitConverter897/1 -> VOUTP_LRPindi_enum/1  "VOUTP_LRPindi_enum"
  VTPM_RRPindi_enum/1 -> VTPM_RRPindi_enum_Inproc/1  "VTPM_RRPindi_enum"
  VTPM_RRPindi_enum_Inproc/1 -> UnitConverter898/1
  UnitConverter898/1 -> VOUTP_RRPindi_enum/1  "VOUTP_RRPindi_enum"
